simulink model "COMPONENT_MDL_Lag_QUAD_and_PEND_with_Ab"  (R2020b)
(part 3 of 12)

A = reshape([sin(THE_Theta).*(I_xx.*sin(THE_Theta).*(-1.0./2.0)+(I_xz.*cos(THE_Psi).*cos(THE_Theta))./2.0+(I_xy.*cos(THE_Theta).*sin(THE_Psi))./2.0).*-2.0-sin(THE_Theta).*(Iprop_xx.*sin(THE_Theta).*(-1.0./2.0)+(Iprop_xz.*cos(THE_Psi).*cos(THE_Theta))./2.0+(Iprop_xy.*cos(THE_Theta).*sin(THE_Psi))./2.0).*8.0+mprop.*(-cos(THE_Theta).*sin(THE_Psi).*(cg_to_mot_H.*sin(THE_Theta)+cg_to_mot_L.*cos(THE_Psi).*cos(THE_Theta))+cg_to_mot_H.*cos(THE_Theta).*sin(THE_Psi).*sin(THE_Theta)+cg_to_mot_L.*cos(THE_Psi).*cos(THE_Theta).^2.*sin(THE_Psi)).*(cos(THE_Theta).*sin(THE_Psi).*(cg_to_mot_H.*sin(THE_Theta)+cg_to_mot_L.*cos(THE_Psi).*cos(THE_Theta)).*(-1.0./2.0)+(cg_to_mot_H.*cos(THE_Theta).*sin(THE_Psi).*sin(THE_Theta))./2.0+(cg_to_mot_L.*cos(THE_Psi).*cos(THE_Theta).^2.*sin(THE_Psi))./2.0).*2.0+mprop.*(cos(THE_Theta).*sin(THE_Psi).*(cg_to_mot_H.*sin(THE_Theta)-cg_to_mot_L.*cos(THE_Psi).*cos(THE_Theta))-cg_to_mot_H.*cos(THE_Theta).*sin(THE_Psi).*sin(THE_Theta)+cg_to_mot_L.*cos(THE_Psi).*cos(THE_Theta).^2.*sin(THE_Psi)).*((cos(THE_Theta).*sin(THE_Psi).*(cg_to_mot_H.*sin(THE_Theta)-cg_to_mot_L.*cos(THE_Psi).*cos(THE_Theta)))./2.0-(cg_to_mot_H.*cos(THE_Theta).*sin(THE_Psi).*sin(THE_Theta))./2.0+(cg_to_mot_L.*cos(THE_Psi).*cos(THE_Theta).^2.*sin(THE_Psi))./2.0).*2.0+mprop.*((cg_to_mot_H.*sin(THE_Theta)+cg_to_mot_L.*cos(THE_Psi).*cos(THE_Theta)).*(cos(THE_Psi).*sin(THE_Phi)-cos(THE_Phi).*sin(THE_Psi).*sin(THE_Theta))+cg_to_mot_L.*cos(THE_Theta).*sin(THE_Psi).*(sin(THE_Phi).*sin(THE_Psi)+cos(THE_Phi).*cos(THE_Psi).*sin(THE_Theta))-cg_to_mot_H.*cos(THE_Phi).*cos(THE_Theta).^2.*sin(THE_Psi)).*(((cg_to_mot_H.*sin(THE_Theta)+cg_to_mot_L.*cos(THE_Psi).*cos(THE_Theta)).*(cos(THE_Psi).*sin(THE_Phi)-cos(THE_Phi).*sin(THE_Psi).*sin(THE_Theta)))./2.0+(cg_to_mot_L.*cos(THE_Theta).*sin(THE_Psi).*(sin(THE_Phi).*sin(THE_Psi)+cos(THE_Phi).*cos(THE_Psi).*sin(THE_Theta)))./2.0-(cg_to_mot_H.*cos(THE_Phi).*cos(THE_Theta).^2.*sin(THE_Psi))./2.0).*2.0+mprop.*(-(cg_to_mot_H.*sin(THE_Theta)-cg_to_mot_L.*cos(THE_Psi).*cos(THE_Theta)).*(cos(THE_Psi).*sin(THE_Phi)-cos(THE_Phi).*sin(THE_Psi).*sin(THE_Theta))+cg_to_mot_L.*cos(THE_Theta).*sin(THE_Psi).*(sin(THE_Phi).*sin(THE_Psi)+cos(THE_Phi).*cos(THE_Psi).*sin(THE_Theta))+cg_to_mot_H.*cos(THE_Phi).*cos(THE_Theta).^2.*sin(THE_Psi)).*((cg_to_mot_H.*sin(THE_Theta)-cg_to_mot_L.*cos(THE_Psi).*cos(THE_Theta)).*(cos(THE_Psi).*sin(THE_Phi)-cos(THE_Phi).*sin(THE_Psi).*sin(THE_Theta)).*(-1.0./2.0)+(cg_to_mot_L.*cos(THE_Theta).*sin(THE_Psi).*(sin(THE_Phi).*sin(THE_Psi)+cos(THE_Phi).*cos(THE_Psi).*sin(THE_Theta)))./2.0+(cg_to_mot_H.*cos(THE_Phi).*cos(THE_Theta).^2.*sin(THE_Psi))./2.0).*2.0+mprop.*((cg_to_mot_H.*sin(THE_Theta)+cg_to_mot_L.*cos(THE_Psi).*cos(THE_Theta)).*(cos(THE_Phi).*cos(THE_Psi)+sin(THE_Phi).*sin(THE_Psi).*sin(THE_Theta))+cg_to_mot_L.*cos(THE_Theta).*sin(THE_Psi).*(cos(THE_Phi).*sin(THE_Psi)-cos(THE_Psi).*sin(THE_Phi).*sin(THE_Theta))+cg_to_mot_H.*cos(THE_Theta).^2.*sin(THE_Phi).*sin(THE_Psi)).*(((cg_to_mot_H.*sin(THE_Theta)+cg_to_mot_L.*cos(THE_Psi).*cos(THE_Theta)).*(cos(THE_Phi).*cos(THE_Psi)+sin(THE_Phi).*sin(THE_Psi).*sin(THE_Theta)))./2.0+(cg_to_mot_L.*cos(THE_Theta).*sin(THE_Psi).*(cos(THE_Phi).*sin(THE_Psi)-cos(THE_Psi).*sin(THE_Phi).*sin(THE_Theta)))./2.0+(cg_to_mot_H.*cos(THE_Theta).^2.*sin(THE_Phi).*sin(THE_Psi))./2.0).*2.0+mprop.*((cg_to_mot_H.*sin(THE_Theta)-cg_to_mot_L.*cos(THE_Psi).*cos(THE_Theta)).*(cos(THE_Phi).*cos(THE_Psi)+sin(THE_Phi).*sin(THE_Psi).*sin(THE_Theta))-cg_to_mot_L.*cos(THE_Theta).*sin(THE_Psi).*(cos(THE_Phi).*sin(THE_Psi)-cos(THE_Psi).*sin(THE_Phi).*sin(THE_Theta))+cg_to_mot_H.*cos(THE_Theta).^2.*sin(THE_Phi).*sin(THE_Psi)).*(((cg_to_mot_H.*sin(THE_Theta)-cg_to_mot_L.*cos(THE_Psi).*cos(THE_Theta)).*(cos(THE_Phi).*cos(THE_Psi)+sin(THE_Phi).*sin(THE_Psi).*sin(THE_Theta)))./2.0-(cg_to_mot_L.*cos(THE_Theta).*sin(THE_Psi).*(cos(THE_Phi).*sin(THE_Psi)-cos(THE_Psi).*sin(THE_Phi).*sin(THE_Theta)))./2.0+(cg_to_mot_H.*cos(THE_Theta).^2.*sin(THE_Phi).*sin(THE_Psi))./2.0).*2.0+mprop.*(-sin(THE_Theta).*(cg_to_mot_L.*cos(THE_Psi).*cos(THE_Theta)+cg_to_mot_H.*cos(THE_Theta).*sin(THE_Psi))+cg_to_mot_H.*cos(THE_Theta).*sin(THE_Psi).*sin(THE_Theta)+cg_to_mot_L.*cos(THE_Psi).*cos(THE_Theta).*sin(THE_Theta)).*(sin(THE_Theta).*(cg_to_mot_L.*cos(THE_Psi).*cos(THE_Theta)+cg_to_mot_H.*cos(THE_Theta).*sin(THE_Psi)).*(-1.0./2.0)+(cg_to_mot_H.*cos(THE_Theta).*sin(THE_Psi).*sin(THE_Theta))./2.0+(cg_to_mot_L.*cos(THE_Psi).*cos(THE_Theta).*sin(THE_Theta))./2.0).*2.0+mprop.*(sin(THE_Theta).*(cg_to_mot_L.*cos(THE_Psi).*cos(THE_Theta)-cg_to_mot_H.*cos(THE_Theta).*sin(THE_Psi))+cg_to_mot_H.*cos(THE_Theta).*sin(THE_Psi).*sin(THE_Theta)-cg_to_mot_L.*cos(THE_Psi).*cos(THE_Theta).*sin(THE_Theta)).*((sin(THE_Theta).*(cg_to_mot_L.*cos(THE_Psi).*cos(THE_Theta)-cg_to_mot_H.*cos(THE_Theta).*sin(THE_Psi)))./2.0+(cg_to_mot_H.*cos(THE_Theta).*sin(THE_Psi).*sin(THE_Theta))./2.0-(cg_to_mot_L.*cos(THE_Psi).*cos(THE_Theta).*sin(THE_Theta))./2.0).*2.0+mprop.*(-cg_to_mot_H.*sin(THE_Theta).*(cos(THE_Psi).*sin(THE_Phi)-cos(THE_Phi).*sin(THE_Psi).*sin(THE_Theta))+cg_to_mot_L.*sin(THE_Theta).*(sin(THE_Phi).*sin(THE_Psi)+cos(THE_Phi).*cos(THE_Psi).*sin(THE_Theta))+cos(THE_Phi).*cos(THE_Theta).*(cg_to_mot_L.*cos(THE_Psi).*cos(THE_Theta)+cg_to_mot_H.*cos(THE_Theta).*sin(THE_Psi))).*(cg_to_mot_H.*sin(THE_Theta).*(cos(THE_Psi).*sin(THE_Phi)-cos(THE_Phi).*sin(THE_Psi).*sin(THE_Theta)).*(-1.0./2.0)+(cg_to_mot_L.*sin(THE_Theta).*(sin(THE_Phi).*sin(THE_Psi)+cos(THE_Phi).*cos(THE_Psi).*sin(THE_Theta)))./2.0+(cos(THE_Phi).*cos(THE_Theta).*(cg_to_mot_L.*cos(THE_Psi).*cos(THE_Theta)+cg_to_mot_H.*cos(THE_Theta).*sin(THE_Psi)))./2.0).*2.0+mprop.*(cg_to_mot_H.*sin(THE_Theta).*(cos(THE_Psi).*sin(THE_Phi)-cos(THE_Phi).*sin(THE_Psi).*sin(THE_Theta))+cg_to_mot_L.*sin(THE_Theta).*(sin(THE_Phi).*sin(THE_Psi)+cos(THE_Phi).*cos(THE_Psi).*sin(THE_Theta))+cos(THE_Phi).*cos(THE_Theta).*(cg_to_mot_L.*cos(THE_Psi).*cos(THE_Theta)-cg_to_mot_H.*cos(THE_Theta).*sin(THE_Psi))).*((cg_to_mot_H.*sin(THE_Theta).*(cos(THE_Psi).*sin(THE_Phi)-cos(THE_Phi).*sin(THE_Psi).*sin(THE_Theta)))./2.0+(cg_to_mot_L.*sin(THE_Theta).*(sin(THE_Phi).*sin(THE_Psi)+cos(THE_Phi).*cos(THE_Psi).*sin(THE_Theta)))./2.0+(cos(THE_Phi).*cos(THE_Theta).*(cg_to_mot_L.*cos(THE_Psi).*cos(THE_Theta)-cg_to_mot_H.*cos(THE_Theta).*sin(THE_Psi)))./2.0).*2.0+m_pend.*((Tv_Z_pend+(Lz_pend.*cos(THE_Psi_pend).*cos(THE_Theta_pend))./2.0).*(sin(THE_Phi).*sin(THE_Psi)+cos(THE_Phi).*cos(THE_Psi).*sin(THE_Theta))+(Lz_pend.*(cos(THE_Psi).*sin(THE_Phi)-cos(THE_Phi).*sin(THE_Psi).*sin(THE_Theta)).*(cos(THE_Phi_pend).*sin(THE_Psi_pend)-cos(THE_Psi_pend).*sin(THE_Phi_pend).*sin(THE_Theta_pend)))./2.0+(Lz_pend.*cos(THE_Phi).*cos(THE_Theta).*(sin(THE_Phi_pend).*sin(THE_Psi_pend)+cos(THE_Phi_pend).*cos(THE_Psi_pend).*sin(THE_Theta_pend)))./2.0).*(((Tv_Z_pend+(Lz_pend.*cos(THE_Psi_pend).*cos(THE_Theta_pend))./2.0).*(sin(THE_Phi).*sin(THE_Psi)+cos(THE_Phi).*cos(THE_Psi).*sin(THE_Theta)))./2.0+(Lz_pend.*(cos(THE_Psi).*sin(THE_Phi)-cos(THE_Phi).*sin(THE_Psi).*sin(THE_Theta)).*(cos(THE_Phi_pend).*sin(THE_Psi_pend)-cos(THE_Psi_pend).*sin(THE_Phi_pend).*sin(THE_Theta_pend)))./4.0+(Lz_pend.*cos(THE_Phi).*cos(THE_Theta).*(sin(THE_Phi_pend).*sin(THE_Psi_pend)+cos(THE_Phi_pend).*cos(THE_Psi_pend).*sin(THE_Theta_pend)))./4.0).*2.0+mprop.*(cg_to_mot_H.*sin(THE_Theta).*(cos(THE_Phi).*cos(THE_Psi)+sin(THE_Phi).*sin(THE_Psi).*sin(THE_Theta))-cg_to_mot_L.*sin(THE_Theta).*(cos(THE_Phi).*sin(THE_Psi)-cos(THE_Psi).*sin(THE_Phi).*sin(THE_Theta))+cos(THE_Theta).*sin(THE_Phi).*(cg_to_mot_L.*cos(THE_Psi).*cos(THE_Theta)+cg_to_mot_H.*cos(THE_Theta).*sin(THE_Psi))).*((cg_to_mot_H.*sin(THE_Theta).*(cos(THE_Phi).*cos(THE_Psi)+sin(THE_Phi).*sin(THE_Psi).*sin(THE_Theta)))./2.0-(cg_to_mot_L.*sin(THE_Theta).*(cos(THE_Phi).*sin(THE_Psi)-cos(THE_Psi).*sin(THE_Phi).*sin(THE_Theta)))./2.0+(cos(THE_Theta).*sin(THE_Phi).*(cg_to_mot_L.*cos(THE_Psi).*cos(THE_Theta)+cg_to_mot_H.*cos(THE_Theta).*sin(THE_Psi)))./2.0).*2.0+mprop.*(cg_to_mot_H.*sin(THE_Theta).*(cos(THE_Phi).*cos(THE_Psi)+sin(THE_Phi).*sin(THE_Psi).*sin(THE_Theta))+cg_to_mot_L.*sin(THE_Theta).*(cos(THE_Phi).*sin(THE_Psi)-cos(THE_Psi).*sin(THE_Phi).*sin(THE_Theta))-cos(THE_Theta).*sin(THE_Phi).*(cg_to_mot_L.*cos(THE_Psi).*cos(THE_Theta)-cg_to_mot_H.*cos(THE_Theta).*sin(THE_Psi))).*((cg_to_mot_H.*sin(THE_Theta).*(cos(THE_Phi).*cos(THE_Psi)+sin(THE_Phi).*sin(THE_Psi).*sin(THE_Theta)))./2.0+(cg_to_mot_L.*sin(THE_Theta).*(cos(THE_Phi).*sin(THE_Psi)-cos(THE_Psi).*sin(THE_Phi).*sin(THE_Theta)))./2.0-(cos(THE_Theta).*sin(THE_Phi).*(cg_to_mot_L.*cos(THE_Psi).*cos(THE_Theta)-cg_to_mot_H.*cos(THE_Theta).*sin(THE_Psi)))./2.0).*2.0+m_pend.*((Tv_Z_pend+(Lz_pend.*cos(THE_Psi_pend).*cos(THE_Theta_pend))./2.0).*(cos(THE_Phi).*sin(THE_Psi)-cos(THE_Psi).*sin(THE_Phi).*sin(THE_Theta))+(Lz_pend.*(cos(THE_Phi).*cos(THE_Psi)+sin(THE_Phi).*sin(THE_Psi).*sin(THE_Theta)).*(cos(THE_Phi_pend).*sin(THE_Psi_pend)-cos(THE_Psi_pend).*sin(THE_Phi_pend).*sin(THE_Theta_pend)))./2.0-(Lz_pend.*cos(THE_Theta).*sin(THE_Phi).*(sin(THE_Phi_pend).*sin(THE_Psi_pend)+cos(THE_Phi_pend).*cos(THE_Psi_pend).*sin(THE_Theta_pend)))./2.0).*(((Tv_Z_pend+(Lz_pend.*cos(THE_Psi_pend).*cos(THE_Theta_pend))./2.0).*(cos(THE_Phi).*sin(THE_Psi)-cos(THE_Psi).*sin(THE_Phi).*sin(THE_Theta)))./2.0+(Lz_pend.*(cos(THE_Phi).*cos(THE_Psi)+sin(THE_Phi).*sin(THE_Psi).*sin(THE_Theta)).*(cos(THE_Phi_pend).*sin(THE_Psi_pend)-cos(THE_Psi_pend).*sin(THE_Phi_pend).*sin(THE_Theta_pend)))./4.0-(Lz_pend.*cos(THE_Theta).*sin(THE_Phi).*(sin(THE_Phi_pend).*sin(THE_Psi_pend)+cos(THE_Phi_pend).*cos(THE_Psi_pend).*sin(THE_Theta_pend)))./4.0).*2.0+cos(THE_Psi).*cos(THE_Theta).*(I_xz.*sin(THE_Theta).*(-1.0./2.0)+(I_zz.*cos(THE_Psi).*cos(THE_Theta))./2.0+(I_yz.*cos(THE_Theta).*sin(THE_Psi))./2.0).*2.0+cos(THE_Psi).*cos(THE_Theta).*(Iprop_xz.*sin(THE_Theta).*(-1.0./2.0)+(Iprop_zz.*cos(THE_Psi).*cos(THE_Theta))./2.0+(Iprop_yz.*cos(THE_Theta).*sin(THE_Psi))./2.0).*8.0+cos(THE_Theta).*sin(THE_Psi).*(I_xy.*sin(THE_Theta).*(-1.0./2.0)+(I_yz.*cos(THE_Psi).*cos(THE_Theta))./2.0+(I_yy.*cos(THE_Theta).*sin(THE_Psi))./2.0).*2.0+cos(THE_Theta).*sin(THE_Psi).*(Iprop_xy.*sin(THE_Theta).*(-1.0./2.0)+(Iprop_yz.*cos(THE_Psi).*cos(THE_Theta))./2.0+(Iprop_yy.*cos(THE_Theta).*sin(THE_Psi))./2.0).*8.0+m_pend.*(Ly_pend.^2./1.2e+1+Lz_pend.^2./1.2e+1).*(cos(THE_Psi).*cos(THE_Theta).*sin(THE_Theta_pend)+cos(THE_Phi_pend).*cos(THE_Theta_pend).*sin(THE_Theta)-cos(THE_Theta).*cos(THE_Theta_pend).*sin(THE_Psi).*sin(THE_Phi_pend)).*((cos(THE_Psi).*cos(THE_Theta).*sin(THE_Theta_pend))./2.0+(cos(THE_Phi_pend).*cos(THE_Theta_pend).*sin(THE_Theta))./2.0-(cos(THE_Theta).*cos(THE_Theta_pend).*sin(THE_Psi).*sin(THE_Phi_pend))./2.0).*2.0+m_pend.*(Lx_pend.^2./1.2e+1+Ly_pend.^2./1.2e+1).*(sin(THE_Theta).*(sin(THE_Phi_pend).*sin(THE_Psi_pend)+cos(THE_Phi_pend).*cos(THE_Psi_pend).*sin(THE_Theta_pend))+cos(THE_Theta).*sin(THE_Psi).*(cos(THE_Phi_pend).*sin(THE_Psi_pend)-cos(THE_Psi_pend).*sin(THE_Phi_pend).*sin(THE_Theta_pend))-cos(THE_Psi).*cos(THE_Theta).*cos(THE_Psi_pend).*cos(THE_Theta_pend)).*((sin(THE_Theta).*(sin(THE_Phi_pend).*sin(THE_Psi_pend)+cos(THE_Phi_pend).*cos(THE_Psi_pend).*sin(THE_Theta_pend)))./2.0+(cos(THE_Theta).*sin(THE_Psi).*(cos(THE_Phi_pend).*sin(THE_Psi_pend)-cos(THE_Psi_pend).*sin(THE_Phi_pend).*sin(THE_Theta_pend)))./2.0-(cos(THE_Psi).*cos(THE_Theta).*cos(THE_Psi_pend).*cos(THE_Theta_pend))./2.0).*2.0+m_pend.*(Lx_pend.^2./1.2e+1+Lz_pend.^2./1.2e+1).*(sin(THE_Theta).*(cos(THE_Psi_pend).*sin(THE_Phi_pend)-cos(THE_Phi_pend).*sin(THE_Psi_pend).*sin(THE_Theta_pend))+cos(THE_Theta).*sin(THE_Psi).*(cos(THE_Phi_pend).*cos(THE_Psi_pend)+sin(THE_Phi_pend).*sin(THE_Psi_pend).*sin(THE_Theta_pend))+cos(THE_Psi).*cos(THE_Theta).*cos(THE_Theta_pend).*sin(THE_Psi_pend)).*((sin(THE_Theta).*(cos(THE_Psi_pend).*sin(THE_Phi_pend)-cos(THE_Phi_pend).*sin(THE_Psi_pend).*sin(THE_Theta_pend)))./2.0+(cos(THE_Theta).*sin(THE_Psi).*(cos(THE_Phi_pend).*cos(THE_Psi_pend)+sin(THE_Phi_pend).*sin(THE_Psi_pend).*sin(THE_Theta_pend)))./2.0+(cos(THE_Psi).*cos(THE_Theta).*cos(THE_Theta_pend).*sin(THE_Psi_pend))./2.0).*2.0,cos(THE_Psi).*(I_xy.*sin(THE_Theta).*(-1.0./2.0)+(I_yz.*cos(THE_Psi).*cos(THE_Theta))./2.0+(I_yy.*cos(THE_Theta).*sin(THE_Psi))./2.0)+cos(THE_Psi).*(Iprop_xy.*sin(THE_Theta).*(-1.0./2.0)+(Iprop_yz.*cos(THE_Psi).*cos(THE_Theta))./2.0+(Iprop_yy.*cos(THE_Theta).*sin(THE_Psi))./2.0).*4.0-sin(THE_Psi).*(I_xz.*sin(THE_Theta).*(-1.0./2.0)+(I_zz.*cos(THE_Psi).*cos(THE_Theta))./2.0+(I_yz.*cos(THE_Theta).*sin(THE_Psi))./2.0)-sin(THE_Psi).*(Iprop_xz.*sin(THE_Theta).*(-1.0./2.0)+(Iprop_zz.*cos(THE_Psi).*cos(THE_Theta))./2.0+(Iprop_yz.*cos(THE_Theta).*sin(THE_Psi))./2.0).*4.0-sin(THE_Theta).*((I_xy.*cos(THE_Psi))./2.0-(I_xz.*sin(THE_Psi))./2.0)-sin(THE_Theta).*((Iprop_xy.*cos(THE_Psi))./2.0-(Iprop_xz.*sin(THE_Psi))./2.0).*4.0+cos(THE_Theta).*sin(THE_Psi).*((I_yy.*cos(THE_Psi))./2.0-(I_yz.*sin(THE_Psi))./2.0)+cos(THE_Theta).*sin(THE_Psi).*((Iprop_yy.*cos(THE_Psi))./2.0-(Iprop_yz.*sin(THE_Psi))./2.0).*4.0-mprop.*(-cg_to_mot_L.*cos(THE_Psi).*(sin(THE_Phi).*sin(THE_Psi)+cos(THE_Phi).*cos(THE_Psi).*sin(THE_Theta))+cg_to_mot_L.*sin(THE_Psi).*(cos(THE_Psi).*sin(THE_Phi)-cos(THE_Phi).*sin(THE_Psi).*sin(THE_Theta))+cg_to_mot_H.*cos(THE_Phi).*cos(THE_Psi).*cos(THE_Theta)).*(((cg_to_mot_H.*sin(THE_Theta)+cg_to_mot_L.*cos(THE_Psi).*cos(THE_Theta)).*(cos(THE_Psi).*sin(THE_Phi)-cos(THE_Phi).*sin(THE_Psi).*sin(THE_Theta)))./2.0+(cg_to_mot_L.*cos(THE_Theta).*sin(THE_Psi).*(sin(THE_Phi).*sin(THE_Psi)+cos(THE_Phi).*cos(THE_Psi).*sin(THE_Theta)))./2.0-(cg_to_mot_H.*cos(THE_Phi).*cos(THE_Theta).^2.*sin(THE_Psi))./2.0)-mprop.*(cg_to_mot_L.*cos(THE_Psi).*(sin(THE_Phi).*sin(THE_Psi)+cos(THE_Phi).*cos(THE_Psi).*sin(THE_Theta)).*(-1.0./2.0)+(cg_to_mot_L.*sin(THE_Psi).*(cos(THE_Psi).*sin(THE_Phi)-cos(THE_Phi).*sin(THE_Psi).*sin(THE_Theta)))./2.0+(cg_to_mot_H.*cos(THE_Phi).*cos(THE_Psi).*cos(THE_Theta))./2.0).*((cg_to_mot_H.*sin(THE_Theta)+cg_to_mot_L.*cos(THE_Psi).*cos(THE_Theta)).*(cos(THE_Psi).*sin(THE_Phi)-cos(THE_Phi).*sin(THE_Psi).*sin(THE_Theta))+cg_to_mot_L.*cos(THE_Theta).*sin(THE_Psi).*(sin(THE_Phi).*sin(THE_Psi)+cos(THE_Phi).*cos(THE_Psi).*sin(THE_Theta))-cg_to_mot_H.*cos(THE_Phi).*cos(THE_Theta).^2.*sin(THE_Psi))+mprop.*(cg_to_mot_L.*cos(THE_Psi).*(sin(THE_Phi).*sin(THE_Psi)+cos(THE_Phi).*cos(THE_Psi).*sin(THE_Theta))-cg_to_mot_L.*sin(THE_Psi).*(cos(THE_Psi).*sin(THE_Phi)-cos(THE_Phi).*sin(THE_Psi).*sin(THE_Theta))+cg_to_mot_H.*cos(THE_Phi).*cos(THE_Psi).*cos(THE_Theta)).*((cg_to_mot_H.*sin(THE_Theta)-cg_to_mot_L.*cos(THE_Psi).*cos(THE_Theta)).*(cos(THE_Psi).*sin(THE_Phi)-cos(THE_Phi).*sin(THE_Psi).*sin(THE_Theta)).*(-1.0./2.0)+(cg_to_mot_L.*cos(THE_Theta).*sin(THE_Psi).*(sin(THE_Phi).*sin(THE_Psi)+cos(THE_Phi).*cos(THE_Psi).*sin(THE_Theta)))./2.0+(cg_to_mot_H.*cos(THE_Phi).*cos(THE_Theta).^2.*sin(THE_Psi))./2.0)+mprop.*((cg_to_mot_L.*cos(THE_Psi).*(sin(THE_Phi).*sin(THE_Psi)+cos(THE_Phi).*cos(THE_Psi).*sin(THE_Theta)))./2.0-(cg_to_mot_L.*sin(THE_Psi).*(cos(THE_Psi).*sin(THE_Phi)-cos(THE_Phi).*sin(THE_Psi).*sin(THE_Theta)))./2.0+(cg_to_mot_H.*cos(THE_Phi).*cos(THE_Psi).*cos(THE_Theta))./2.0).*(-(cg_to_mot_H.*sin(THE_Theta)-cg_to_mot_L.*cos(THE_Psi).*cos(THE_Theta)).*(cos(THE_Psi).*sin(THE_Phi)-cos(THE_Phi).*sin(THE_Psi).*sin(THE_Theta))+cg_to_mot_L.*cos(THE_Theta).*sin(THE_Psi).*(sin(THE_Phi).*sin(THE_Psi)+cos(THE_Phi).*cos(THE_Psi).*sin(THE_Theta))+cg_to_mot_H.*cos(THE_Phi).*cos(THE_Theta).^2.*sin(THE_Psi))+mprop.*((cg_to_mot_L.*cos(THE_Psi).*(cos(THE_Phi).*sin(THE_Psi)-cos(THE_Psi).*sin(THE_Phi).*sin(THE_Theta)))./2.0-(cg_to_mot_L.*sin(THE_Psi).*(cos(THE_Phi).*cos(THE_Psi)+sin(THE_Phi).*sin(THE_Psi).*sin(THE_Theta)))./2.0+(cg_to_mot_H.*cos(THE_Psi).*cos(THE_Theta).*sin(THE_Phi))./2.0).*((cg_to_mot_H.*sin(THE_Theta)+cg_to_mot_L.*cos(THE_Psi).*cos(THE_Theta)).*(cos(THE_Phi).*cos(THE_Psi)+sin(THE_Phi).*sin(THE_Psi).*sin(THE_Theta))+cg_to_mot_L.*cos(THE_Theta).*sin(THE_Psi).*(cos(THE_Phi).*sin(THE_Psi)-cos(THE_Psi).*sin(THE_Phi).*sin(THE_Theta))+cg_to_mot_H.*cos(THE_Theta).^2.*sin(THE_Phi).*sin(THE_Psi))+mprop.*(cg_to_mot_L.*cos(THE_Psi).*(cos(THE_Phi).*sin(THE_Psi)-cos(THE_Psi).*sin(THE_Phi).*sin(THE_Theta))-cg_to_mot_L.*sin(THE_Psi).*(cos(THE_Phi).*cos(THE_Psi)+sin(THE_Phi).*sin(THE_Psi).*sin(THE_Theta))+cg_to_mot_H.*cos(THE_Psi).*cos(THE_Theta).*sin(THE_Phi)).*(((cg_to_mot_H.*sin(THE_Theta)+cg_to_mot_L.*cos(THE_Psi).*cos(THE_Theta)).*(cos(THE_Phi).*cos(THE_Psi)+sin(THE_Phi).*sin(THE_Psi).*sin(THE_Theta)))./2.0+(cg_to_mot_L.*cos(THE_Theta).*sin(THE_Psi).*(cos(THE_Phi).*sin(THE_Psi)-cos(THE_Psi).*sin(THE_Phi).*sin(THE_Theta)))./2.0+(cg_to_mot_H.*cos(THE_Theta).^2.*sin(THE_Phi).*sin(THE_Psi))./2.0)+mprop.*(-cg_to_mot_L.*cos(THE_Psi).*(cos(THE_Phi).*sin(THE_Psi)-cos(THE_Psi).*sin(THE_Phi).*sin(THE_Theta))+cg_to_mot_L.*sin(THE_Psi).*(cos(THE_Phi).*cos(THE_Psi)+sin(THE_Phi).*sin(THE_Psi).*sin(THE_Theta))+cg_to_mot_H.*cos(THE_Psi).*cos(THE_Theta).*sin(THE_Phi)).*(((cg_to_mot_H.*sin(THE_Theta)-cg_to_mot_L.*cos(THE_Psi).*cos(THE_Theta)).*(cos(THE_Phi).*cos(THE_Psi)+sin(THE_Phi).*sin(THE_Psi).*sin(THE_Theta)))./2.0-(cg_to_mot_L.*cos(THE_Theta).*sin(THE_Psi).*(cos(THE_Phi).*sin(THE_Psi)-cos(THE_Psi).*sin(THE_Phi).*sin(THE_Theta)))./2.0+(cg_to_mot_H.*cos(THE_Theta).^2.*sin(THE_Phi).*sin(THE_Psi))./2.0)+mprop.*(cg_to_mot_L.*cos(THE_Psi).*(cos(THE_Phi).*sin(THE_Psi)-cos(THE_Psi).*sin(THE_Phi).*sin(THE_Theta)).*(-1.0./2.0)+(cg_to_mot_L.*sin(THE_Psi).*(cos(THE_Phi).*cos(THE_Psi)+sin(THE_Phi).*sin(THE_Psi).*sin(THE_Theta)))./2.0+(cg_to_mot_H.*cos(THE_Psi).*cos(THE_Theta).*sin(THE_Phi))./2.0).*((cg_to_mot_H.*sin(THE_Theta)-cg_to_mot_L.*cos(THE_Psi).*cos(THE_Theta)).*(cos(THE_Phi).*cos(THE_Psi)+sin(THE_Phi).*sin(THE_Psi).*sin(THE_Theta))-cg_to_mot_L.*cos(THE_Theta).*sin(THE_Psi).*(cos(THE_Phi).*sin(THE_Psi)-cos(THE_Psi).*sin(THE_Phi).*sin(THE_Theta))+cg_to_mot_H.*cos(THE_Theta).^2.*sin(THE_Phi).*sin(THE_Psi))-m_pend.*((Lz_pend.*cos(THE_Phi).*sin(THE_Theta).*(sin(THE_Phi_pend).*sin(THE_Psi_pend)+cos(THE_Phi_pend).*cos(THE_Psi_pend).*sin(THE_Theta_pend)))./4.0-(cos(THE_Phi).*cos(THE_Psi).*cos(THE_Theta).*(Tv_Z_pend+(Lz_pend.*cos(THE_Psi_pend).*cos(THE_Theta_pend))./2.0))./2.0+(Lz_pend.*cos(THE_Phi).*cos(THE_Theta).*sin(THE_Psi).*(cos(THE_Phi_pend).*sin(THE_Psi_pend)-cos(THE_Psi_pend).*sin(THE_Phi_pend).*sin(THE_Theta_pend)))./4.0).*((Tv_Z_pend+(Lz_pend.*cos(THE_Psi_pend).*cos(THE_Theta_pend))./2.0).*(cos(THE_Phi).*sin(THE_Psi)-cos(THE_Psi).*sin(THE_Phi).*sin(THE_Theta))+(Lz_pend.*(cos(THE_Phi).*cos(THE_Psi)+sin(THE_Phi).*sin(THE_Psi).*sin(THE_Theta)).*(cos(THE_Phi_pend).*sin(THE_Psi_pend)-cos(THE_Psi_pend).*sin(THE_Phi_pend).*sin(THE_Theta_pend)))./2.0-(Lz_pend.*cos(THE_Theta).*sin(THE_Phi).*(sin(THE_Phi_pend).*sin(THE_Psi_pend)+cos(THE_Phi_pend).*cos(THE_Psi_pend).*sin(THE_Theta_pend)))./2.0)-m_pend.*((Lz_pend.*cos(THE_Phi).*sin(THE_Theta).*(sin(THE_Phi_pend).*sin(THE_Psi_pend)+cos(THE_Phi_pend).*cos(THE_Psi_pend).*sin(THE_Theta_pend)))./2.0-cos(THE_Phi).*cos(THE_Psi).*cos(THE_Theta).*(Tv_Z_pend+(Lz_pend.*cos(THE_Psi_pend).*cos(THE_Theta_pend))./2.0)+(Lz_pend.*cos(THE_Phi).*cos(THE_Theta).*sin(THE_Psi).*(cos(THE_Phi_pend).*sin(THE_Psi_pend)-cos(THE_Psi_pend).*sin(THE_Phi_pend).*sin(THE_Theta_pend)))./2.0).*(((Tv_Z_pend+(Lz_pend.*cos(THE_Psi_pend).*cos(THE_Theta_pend))./2.0).*(cos(THE_Phi).*sin(THE_Psi)-cos(THE_Psi).*sin(THE_Phi).*sin(THE_Theta)))./2.0+(Lz_pend.*(cos(THE_Phi).*cos(THE_Psi)+sin(THE_Phi).*sin(THE_Psi).*sin(THE_Theta)).*(cos(THE_Phi_pend).*sin(THE_Psi_pend)-cos(THE_Psi_pend).*sin(THE_Phi_pend).*sin(THE_Theta_pend)))./4.0-(Lz_pend.*cos(THE_Theta).*sin(THE_Phi).*(sin(THE_Phi_pend).*sin(THE_Psi_pend)+cos(THE_Phi_pend).*cos(THE_Psi_pend).*sin(THE_Theta_pend)))./4.0)+mprop.*(cos(THE_Theta).*sin(THE_Psi).*(cg_to_mot_H.*sin(THE_Theta)+cg_to_mot_L.*cos(THE_Psi).*cos(THE_Theta)).*(-1.0./2.0)+(cg_to_mot_H.*cos(THE_Theta).*sin(THE_Psi).*sin(THE_Theta))./2.0+(cg_to_mot_L.*cos(THE_Psi).*cos(THE_Theta).^2.*sin(THE_Psi))./2.0).*(cg_to_mot_H.*cos(THE_Psi).*sin(THE_Theta)+cg_to_mot_L.*cos(THE_Psi).^2.*cos(THE_Theta)+cg_to_mot_L.*cos(THE_Theta).*sin(THE_Psi).^2)+mprop.*(-cos(THE_Theta).*sin(THE_Psi).*(cg_to_mot_H.*sin(THE_Theta)+cg_to_mot_L.*cos(THE_Psi).*cos(THE_Theta))+cg_to_mot_H.*cos(THE_Theta).*sin(THE_Psi).*sin(THE_Theta)+cg_to_mot_L.*cos(THE_Psi).*cos(THE_Theta).^2.*sin(THE_Psi)).*((cg_to_mot_H.*cos(THE_Psi).*sin(THE_Theta))./2.0+(cg_to_mot_L.*cos(THE_Psi).^2.*cos(THE_Theta))./2.0+(cg_to_mot_L.*cos(THE_Theta).*sin(THE_Psi).^2)./2.0)+mprop.*(cos(THE_Theta).*sin(THE_Psi).*(cg_to_mot_H.*sin(THE_Theta)-cg_to_mot_L.*cos(THE_Psi).*cos(THE_Theta))-cg_to_mot_H.*cos(THE_Theta).*sin(THE_Psi).*sin(THE_Theta)+cg_to_mot_L.*cos(THE_Psi).*cos(THE_Theta).^2.*sin(THE_Psi)).*(cg_to_mot_H.*cos(THE_Psi).*sin(THE_Theta).*(-1.0./2.0)+(cg_to_mot_L.*cos(THE_Psi).^2.*cos(THE_Theta))./2.0+(cg_to_mot_L.*cos(THE_Theta).*sin(THE_Psi).^2)./2.0)+mprop.*((cos(THE_Theta).*sin(THE_Psi).*(cg_to_mot_H.*sin(THE_Theta)-cg_to_mot_L.*cos(THE_Psi).*cos(THE_Theta)))./2.0-(cg_to_mot_H.*cos(THE_Theta).*sin(THE_Psi).*sin(THE_Theta))./2.0+(cg_to_mot_L.*cos(THE_Psi).*cos(THE_Theta).^2.*sin(THE_Psi))./2.0).*(-cg_to_mot_H.*cos(THE_Psi).*sin(THE_Theta)+cg_to_mot_L.*cos(THE_Psi).^2.*cos(THE_Theta)+cg_to_mot_L.*cos(THE_Theta).*sin(THE_Psi).^2)-m_pend.*((Lz_pend.*sin(THE_Phi).*sin(THE_Theta).*(sin(THE_Phi_pend).*sin(THE_Psi_pend)+cos(THE_Phi_pend).*cos(THE_Psi_pend).*sin(THE_Theta_pend)))./4.0-(cos(THE_Psi).*cos(THE_Theta).*sin(THE_Phi).*(Tv_Z_pend+(Lz_pend.*cos(THE_Psi_pend).*cos(THE_Theta_pend))./2.0))./2.0+(Lz_pend.*cos(THE_Theta).*sin(THE_Phi).*sin(THE_Psi).*(cos(THE_Phi_pend).*sin(THE_Psi_pend)-cos(THE_Psi_pend).*sin(THE_Phi_pend).*sin(THE_Theta_pend)))./4.0).*((Tv_Z_pend+(Lz_pend.*cos(THE_Psi_pend).*cos(THE_Theta_pend))./2.0).*(sin(THE_Phi).*sin(THE_Psi)+cos(THE_Phi).*cos(THE_Psi).*sin(THE_Theta))+(Lz_pend.*(cos(THE_Psi).*sin(THE_Phi)-cos(THE_Phi).*sin(THE_Psi).*sin(THE_Theta)).*(cos(THE_Phi_pend).*sin(THE_Psi_pend)-cos(THE_Psi_pend).*sin(THE_Phi_pend).*sin(THE_Theta_pend)))./2.0+(Lz_pend.*cos(THE_Phi).*cos(THE_Theta).*(sin(THE_Phi_pend).*sin(THE_Psi_pend)+cos(THE_Phi_pend).*cos(THE_Psi_pend).*sin(THE_Theta_pend)))./2.0)-m_pend.*((Lz_pend.*sin(THE_Phi).*sin(THE_Theta).*(sin(THE_Phi_pend).*sin(THE_Psi_pend)+cos(THE_Phi_pend).*cos(THE_Psi_pend).*sin(THE_Theta_pend)))./2.0-cos(THE_Psi).*cos(THE_Theta).*sin(THE_Phi).*(Tv_Z_pend+(Lz_pend.*cos(THE_Psi_pend).*cos(THE_Theta_pend))./2.0)+(Lz_pend.*cos(THE_Theta).*sin(THE_Phi).*sin(THE_Psi).*(cos(THE_Phi_pend).*sin(THE_Psi_pend)-cos(THE_Psi_pend).*sin(THE_Phi_pend).*sin(THE_Theta_pend)))./2.0).*(((Tv_Z_pend+(Lz_pend.*cos(THE_Psi_pend).*cos(THE_Theta_pend))./2.0).*(sin(THE_Phi).*sin(THE_Psi)+cos(THE_Phi).*cos(THE_Psi).*sin(THE_Theta)))./2.0+(Lz_pend.*(cos(THE_Psi).*sin(THE_Phi)-cos(THE_Phi).*sin(THE_Psi).*sin(THE_Theta)).*(cos(THE_Phi_pend).*sin(THE_Psi_pend)-cos(THE_Psi_pend).*sin(THE_Phi_pend).*sin(THE_Theta_pend)))./4.0+(Lz_pend.*cos(THE_Phi).*cos(THE_Theta).*(sin(THE_Phi_pend).*sin(THE_Psi_pend)+cos(THE_Phi_pend).*cos(THE_Psi_pend).*sin(THE_Theta_pend)))./4.0)+cos(THE_Psi).*cos(THE_Theta).*((I_yz.*cos(THE_Psi))./2.0-(I_zz.*sin(THE_Psi))./2.0)+cos(THE_Psi).*cos(THE_Theta).*((Iprop_yz.*cos(THE_Psi))./2.0-(Iprop_zz.*sin(THE_Psi))./2.0).*4.0-m_pend.*(Ly_pend.^2./1.2e+1+Lz_pend.^2./1.2e+1).*((sin(THE_Psi).*sin(THE_Theta_pend))./2.0+(cos(THE_Psi).*cos(THE_Theta_pend).*sin(THE_Phi_pend))./2.0).*(cos(THE_Psi).*cos(THE_Theta).*sin(THE_Theta_pend)+cos(THE_Phi_pend).*cos(THE_Theta_pend).*sin(THE_Theta)-cos(THE_Theta).*cos(THE_Theta_pend).*sin(THE_Psi).*sin(THE_Phi_pend))-m_pend.*(Ly_pend.^2./1.2e+1+Lz_pend.^2./1.2e+1).*(sin(THE_Psi).*sin(THE_Theta_pend)+cos(THE_Psi).*cos(THE_Theta_pend).*sin(THE_Phi_pend)).*((cos(THE_Psi).*cos(THE_Theta).*sin(THE_Theta_pend))./2.0+(cos(THE_Phi_pend).*cos(THE_Theta_pend).*sin(THE_Theta))./2.0-(cos(THE_Theta).*cos(THE_Theta_pend).*sin(THE_Psi).*sin(THE_Phi_pend))./2.0)-(mprop.*sin(THE_Theta).*(cg_to_mot_H.*cos(THE_Psi)+cg_to_mot_L.*sin(THE_Psi)).*(sin(THE_Theta).*(cg_to_mot_L.*cos(THE_Psi).*cos(THE_Theta)-cg_to_mot_H.*cos(THE_Theta).*sin(THE_Psi))+cg_to_mot_H.*cos(THE_Theta).*sin(THE_Psi).*sin(THE_Theta)-cg_to_mot_L.*cos(THE_Psi).*cos(THE_Theta).*sin(THE_Theta)))./2.0-(mprop.*sin(THE_Theta).*(cg_to_mot_H.*cos(THE_Psi)-cg_to_mot_L.*sin(THE_Psi)).*(-sin(THE_Theta).*(cg_to_mot_L.*cos(THE_Psi).*cos(THE_Theta)+cg_to_mot_H.*cos(THE_Theta).*sin(THE_Psi))+cg_to_mot_H.*cos(THE_Theta).*sin(THE_Psi).*sin(THE_Theta)+cg_to_mot_L.*cos(THE_Psi).*cos(THE_Theta).*sin(THE_Theta)))./2.0-mprop.*sin(THE_Theta).*(cg_to_mot_H.*cos(THE_Psi)+cg_to_mot_L.*sin(THE_Psi)).*((sin(THE_Theta).*(cg_to_mot_L.*cos(THE_Psi).*cos(THE_Theta)-cg_to_mot_H.*cos(THE_Theta).*sin(THE_Psi)))./2.0+(cg_to_mot_H.*cos(THE_Theta).*sin(THE_Psi).*sin(THE_Theta))./2.0-(cg_to_mot_L.*cos(THE_Psi).*cos(THE_Theta).*sin(THE_Theta))./2.0)-mprop.*sin(THE_Theta).*(cg_to_mot_H.*cos(THE_Psi)-cg_to_mot_L.*sin(THE_Psi)).*(sin(THE_Theta).*(cg_to_mot_L.*cos(THE_Psi).*cos(THE_Theta)+cg_to_mot_H.*cos(THE_Theta).*sin(THE_Psi)).*(-1.0./2.0)+(cg_to_mot_H.*cos(THE_Theta).*sin(THE_Psi).*sin(THE_Theta))./2.0+(cg_to_mot_L.*cos(THE_Psi).*cos(THE_Theta).*sin(THE_Theta))./2.0)+m_pend.*(Lx_pend.^2./1.2e+1+Ly_pend.^2./1.2e+1).*((cos(THE_Psi).*(cos(THE_Phi_pend).*sin(THE_Psi_pend)-cos(THE_Psi_pend).*sin(THE_Phi_pend).*sin(THE_Theta_pend)))./2.0+(cos(THE_Psi_pend).*cos(THE_Theta_pend).*sin(THE_Psi))./2.0).*(sin(THE_Theta).*(sin(THE_Phi_pend).*sin(THE_Psi_pend)+cos(THE_Phi_pend).*cos(THE_Psi_pend).*sin(THE_Theta_pend))+cos(THE_Theta).*sin(THE_Psi).*(cos(THE_Phi_pend).*sin(THE_Psi_pend)-cos(THE_Psi_pend).*sin(THE_Phi_pend).*sin(THE_Theta_pend))-cos(THE_Psi).*cos(THE_Theta).*cos(THE_Psi_pend).*cos(THE_Theta_pend))+m_pend.*(Lx_pend.^2./1.2e+1+Ly_pend.^2./1.2e+1).*(cos(THE_Psi).*(cos(THE_Phi_pend).*sin(THE_Psi_pend)-cos(THE_Psi_pend).*sin(THE_Phi_pend).*sin(THE_Theta_pend))+cos(THE_Psi_pend).*cos(THE_Theta_pend).*sin(THE_Psi)).*((sin(THE_Theta).*(sin(THE_Phi_pend).*sin(THE_Psi_pend)+cos(THE_Phi_pend).*cos(THE_Psi_pend).*sin(THE_Theta_pend)))./2.0+(cos(THE_Theta).*sin(THE_Psi).*(cos(THE_Phi_pend).*sin(THE_Psi_pend)-cos(THE_Psi_pend).*sin(THE_Phi_pend).*sin(THE_Theta_pend)))./2.0-(cos(THE_Psi).*cos(THE_Theta).*cos(THE_Psi_pend).*cos(THE_Theta_pend))./2.0)+m_pend.*((cos(THE_Psi).*(cos(THE_Phi_pend).*cos(THE_Psi_pend)+sin(THE_Phi_pend).*sin(THE_Psi_pend).*sin(THE_Theta_pend)))./2.0-(cos(THE_Theta_pend).*sin(THE_Psi).*sin(THE_Psi_pend))./2.0).*(Lx_pend.^2./1.2e+1+Lz_pend.^2./1.2e+1).*(sin(THE_Theta).*(cos(THE_Psi_pend).*sin(THE_Phi_pend)-cos(THE_Phi_pend).*sin(THE_Psi_pend).*sin(THE_Theta_pend))+cos(THE_Theta).*sin(THE_Psi).*(cos(THE_Phi_pend).*cos(THE_Psi_pend)+sin(THE_Phi_pend).*sin(THE_Psi_pend).*sin(THE_Theta_pend))+cos(THE_Psi).*cos(THE_Theta).*cos(THE_Theta_pend).*sin(THE_Psi_pend))+m_pend.*(cos(THE_Psi).*(cos(THE_Phi_pend).*cos(THE_Psi_pend)+sin(THE_Phi_pend).*sin(THE_Psi_pend).*sin(THE_Theta_pend))-cos(THE_Theta_pend).*sin(THE_Psi).*sin(THE_Psi_pend)).*(Lx_pend.^2./1.2e+1+Lz_pend.^2./1.2e+1).*((sin(THE_Theta).*(cos(THE_Psi_pend).*sin(THE_Phi_pend)-cos(THE_Phi_pend).*sin(THE_Psi_pend).*sin(THE_Theta_pend)))./2.0+(cos(THE_Theta).*sin(THE_Psi).*(cos(THE_Phi_pend).*cos(THE_Psi_pend)+sin(THE_Phi_pend).*sin(THE_Psi_pend).*sin(THE_Theta_pend)))./2.0+(cos(THE_Psi).*cos(THE_Theta).*cos(THE_Theta_pend).*sin(THE_Psi_pend))./2.0)-(mprop.*cos(THE_Phi).*cos(THE_Theta).*(cg_to_mot_H.*cos(THE_Psi)+cg_to_mot_L.*sin(THE_Psi)).*(cg_to_mot_H.*sin(THE_Theta).*(cos(THE_Psi).*sin(THE_Phi)-cos(THE_Phi).*sin(THE_Psi).*sin(THE_Theta))+cg_to_mot_L.*sin(THE_Theta).*(sin(THE_Phi).*sin(THE_Psi)+cos(THE_Phi).*cos(THE_Psi).*sin(THE_Theta))+cos(THE_Phi).*cos(THE_Theta).*(cg_to_mot_L.*cos(THE_Psi).*cos(THE_Theta)-cg_to_mot_H.*cos(THE_Theta).*sin(THE_Psi))))./2.0+(mprop.*cos(THE_Phi).*cos(THE_Theta).*(cg_to_mot_H.*cos(THE_Psi)-cg_to_mot_L.*sin(THE_Psi)).*(-cg_to_mot_H.*sin(THE_Theta).*(cos(THE_Psi).*sin(THE_Phi)-cos(THE_Phi).*sin(THE_Psi).*sin(THE_Theta))+cg_to_mot_L.*sin(THE_Theta).*(sin(THE_Phi).*sin(THE_Psi)+cos(THE_Phi).*cos(THE_Psi).*sin(THE_Theta))+cos(THE_Phi).*cos(THE_Theta).*(cg_to_mot_L.*cos(THE_Psi).*cos(THE_Theta)+cg_to_mot_H.*cos(THE_Theta).*sin(THE_Psi))))./2.0-mprop.*cos(THE_Phi).*cos(THE_Theta).*(cg_to_mot_H.*cos(THE_Psi)+cg_to_mot_L.*sin(THE_Psi)).*((cg_to_mot_H.*sin(THE_Theta).*(cos(THE_Psi).*sin(THE_Phi)-cos(THE_Phi).*sin(THE_Psi).*sin(THE_Theta)))./2.0+(cg_to_mot_L.*sin(THE_Theta).*(sin(THE_Phi).*sin(THE_Psi)+cos(THE_Phi).*cos(THE_Psi).*sin(THE_Theta)))./2.0+(cos(THE_Phi).*cos(THE_Theta).*(cg_to_mot_L.*cos(THE_Psi).*cos(THE_Theta)-cg_to_mot_H.*cos(THE_Theta).*sin(THE_Psi)))./2.0)+mprop.*cos(THE_Phi).*cos(THE_Theta).*(cg_to_mot_H.*cos(THE_Psi)-cg_to_mot_L.*sin(THE_Psi)).*(cg_to_mot_H.*sin(THE_Theta).*(cos(THE_Psi).*sin(THE_Phi)-cos(THE_Phi).*sin(THE_Psi).*sin(THE_Theta)).*(-1.0./2.0)+(cg_to_mot_L.*sin(THE_Theta).*(sin(THE_Phi).*sin(THE_Psi)+cos(THE_Phi).*cos(THE_Psi).*sin(THE_Theta)))./2.0+(cos(THE_Phi).*cos(THE_Theta).*(cg_to_mot_L.*cos(THE_Psi).*cos(THE_Theta)+cg_to_mot_H.*cos(THE_Theta).*sin(THE_Psi)))./2.0)+(mprop.*cos(THE_Theta).*sin(THE_Phi).*(cg_to_mot_H.*cos(THE_Psi)+cg_to_mot_L.*sin(THE_Psi)).*(cg_to_mot_H.*sin(THE_Theta).*(cos(THE_Phi).*cos(THE_Psi)+sin(THE_Phi).*sin(THE_Psi).*sin(THE_Theta))+cg_to_mot_L.*sin(THE_Theta).*(cos(THE_Phi).*sin(THE_Psi)-cos(THE_Psi).*sin(THE_Phi).*sin(THE_Theta))-cos(THE_Theta).*sin(THE_Phi).*(cg_to_mot_L.*cos(THE_Psi).*cos(THE_Theta)-cg_to_mot_H.*cos(THE_Theta).*sin(THE_Psi))))./2.0+(mprop.*cos(THE_Theta).*sin(THE_Phi).*(cg_to_mot_H.*cos(THE_Psi)-cg_to_mot_L.*sin(THE_Psi)).*(cg_to_mot_H.*sin(THE_Theta).*(cos(THE_Phi).*cos(THE_Psi)+sin(THE_Phi).*sin(THE_Psi).*sin(THE_Theta))-cg_to_mot_L.*sin(THE_Theta).*(cos(THE_Phi).*sin(THE_Psi)-cos(THE_Psi).*sin(THE_Phi).*sin(THE_Theta))+cos(THE_Theta).*sin(THE_Phi).*(cg_to_mot_L.*cos(THE_Psi).*cos(THE_Theta)+cg_to_mot_H.*cos(THE_Theta).*sin(THE_Psi))))./2.0+mprop.*cos(THE_Theta).*sin(THE_Phi).*(cg_to_mot_H.*cos(THE_Psi)+cg_to_mot_L.*sin(THE_Psi)).*((cg_to_mot_H.*sin(THE_Theta).*(cos(THE_Phi).*cos(THE_Psi)+sin(THE_Phi).*sin(THE_Psi).*sin(THE_Theta)))./2.0+(cg_to_mot_L.*sin(THE_Theta).*(cos(THE_Phi).*sin(THE_Psi)-cos(THE_Psi).*sin(THE_Phi).*sin(THE_Theta)))./2.0-(cos(THE_Theta).*sin(THE_Phi).*(cg_to_mot_L.*cos(THE_Psi).*cos(THE_Theta)-cg_to_mot_H.*cos(THE_Theta).*sin(THE_Psi)))./2.0)+mprop.*cos(THE_Theta).*sin(THE_Phi).*(cg_to_mot_H.*cos(THE_Psi)-cg_to_mot_L.*sin(THE_Psi)).*((cg_to_mot_H.*sin(THE_Theta).*(cos(THE_Phi).*cos(THE_Psi)+sin(THE_Phi).*sin(THE_Psi).*sin(THE_Theta)))./2.0-(cg_to_mot_L.*sin(THE_Theta).*(cos(THE_Phi).*sin(THE_Psi)-cos(THE_Psi).*sin(THE_Phi).*sin(THE_Theta)))./2.0+(cos(THE_Theta).*sin(THE_Phi).*(cg_to_mot_L.*cos(THE_Psi).*cos(THE_Theta)+cg_to_mot_H.*cos(THE_Theta).*sin(THE_Psi)))./2.0),-I_xx.*sin(THE_Theta)-Iprop_xx.*sin(THE_Theta).*4.0+I_xz.*cos(THE_Psi).*cos(THE_Theta)+Iprop_xz.*cos(THE_Psi).*cos(THE_Theta).*4.0+I_xy.*cos(THE_Theta).*sin(THE_Psi)+Iprop_xy.*cos(THE_Theta).*sin(THE_Psi).*4.0+mprop.*((cg_to_mot_H.*(cos(THE_Psi).*sin(THE_Phi)-cos(THE_Phi).*sin(THE_Psi).*sin(THE_Theta)))./2.0-(cg_to_mot_L.*(sin(THE_Phi).*sin(THE_Psi)+cos(THE_Phi).*cos(THE_Psi).*sin(THE_Theta)))./2.0).*(-cg_to_mot_H.*sin(THE_Theta).*(cos(THE_Psi).*sin(THE_Phi)-cos(THE_Phi).*sin(THE_Psi).*sin(THE_Theta))+cg_to_mot_L.*sin(THE_Theta).*(sin(THE_Phi).*sin(THE_Psi)+cos(THE_Phi).*cos(THE_Psi).*sin(THE_Theta))+cos(THE_Phi).*cos(THE_Theta).*(cg_to_mot_L.*cos(THE_Psi).*cos(THE_Theta)+cg_to_mot_H.*cos(THE_Theta).*sin(THE_Psi)))-mprop.*((cg_to_mot_H.*(cos(THE_Psi).*sin(THE_Phi)-cos(THE_Phi).*sin(THE_Psi).*sin(THE_Theta)))./2.0+(cg_to_mot_L.*(sin(THE_Phi).*sin(THE_Psi)+cos(THE_Phi).*cos(THE_Psi).*sin(THE_Theta)))./2.0).*(cg_to_mot_H.*sin(THE_Theta).*(cos(THE_Psi).*sin(THE_Phi)-cos(THE_Phi).*sin(THE_Psi).*sin(THE_Theta))+cg_to_mot_L.*sin(THE_Theta).*(sin(THE_Phi).*sin(THE_Psi)+cos(THE_Phi).*cos(THE_Psi).*sin(THE_Theta))+cos(THE_Phi).*cos(THE_Theta).*(cg_to_mot_L.*cos(THE_Psi).*cos(THE_Theta)-cg_to_mot_H.*cos(THE_Theta).*sin(THE_Psi)))-mprop.*(cg_to_mot_H.*(cos(THE_Psi).*sin(THE_Phi)-cos(THE_Phi).*sin(THE_Psi).*sin(THE_Theta))+cg_to_mot_L.*(sin(THE_Phi).*sin(THE_Psi)+cos(THE_Phi).*cos(THE_Psi).*sin(THE_Theta))).*((cg_to_mot_H.*sin(THE_Theta).*(cos(THE_Psi).*sin(THE_Phi)-cos(THE_Phi).*sin(THE_Psi).*sin(THE_Theta)))./2.0+(cg_to_mot_L.*sin(THE_Theta).*(sin(THE_Phi).*sin(THE_Psi)+cos(THE_Phi).*cos(THE_Psi).*sin(THE_Theta)))./2.0+(cos(THE_Phi).*cos(THE_Theta).*(cg_to_mot_L.*cos(THE_Psi).*cos(THE_Theta)-cg_to_mot_H.*cos(THE_Theta).*sin(THE_Psi)))./2.0)+mprop.*(cg_to_mot_H.*(cos(THE_Psi).*sin(THE_Phi)-cos(THE_Phi).*sin(THE_Psi).*sin(THE_Theta))-cg_to_mot_L.*(sin(THE_Phi).*sin(THE_Psi)+cos(THE_Phi).*cos(THE_Psi).*sin(THE_Theta))).*(cg_to_mot_H.*sin(THE_Theta).*(cos(THE_Psi).*sin(THE_Phi)-cos(THE_Phi).*sin(THE_Psi).*sin(THE_Theta)).*(-1.0./2.0)+(cg_to_mot_L.*sin(THE_Theta).*(sin(THE_Phi).*sin(THE_Psi)+cos(THE_Phi).*cos(THE_Psi).*sin(THE_Theta)))./2.0+(cos(THE_Phi).*cos(THE_Theta).*(cg_to_mot_L.*cos(THE_Psi).*cos(THE_Theta)+cg_to_mot_H.*cos(THE_Theta).*sin(THE_Psi)))./2.0)-mprop.*((cg_to_mot_H.*(cos(THE_Phi).*cos(THE_Psi)+sin(THE_Phi).*sin(THE_Psi).*sin(THE_Theta)))./2.0-(cg_to_mot_L.*(cos(THE_Phi).*sin(THE_Psi)-cos(THE_Psi).*sin(THE_Phi).*sin(THE_Theta)))./2.0).*(cg_to_mot_H.*sin(THE_Theta).*(cos(THE_Phi).*cos(THE_Psi)+sin(THE_Phi).*sin(THE_Psi).*sin(THE_Theta))-cg_to_mot_L.*sin(THE_Theta).*(cos(THE_Phi).*sin(THE_Psi)-cos(THE_Psi).*sin(THE_Phi).*sin(THE_Theta))+cos(THE_Theta).*sin(THE_Phi).*(cg_to_mot_L.*cos(THE_Psi).*cos(THE_Theta)+cg_to_mot_H.*cos(THE_Theta).*sin(THE_Psi)))-mprop.*((cg_to_mot_H.*(cos(THE_Phi).*cos(THE_Psi)+sin(THE_Phi).*sin(THE_Psi).*sin(THE_Theta)))./2.0+(cg_to_mot_L.*(cos(THE_Phi).*sin(THE_Psi)-cos(THE_Psi).*sin(THE_Phi).*sin(THE_Theta)))./2.0).*(cg_to_mot_H.*sin(THE_Theta).*(cos(THE_Phi).*cos(THE_Psi)+sin(THE_Phi).*sin(THE_Psi).*sin(THE_Theta))+cg_to_mot_L.*sin(THE_Theta).*(cos(THE_Phi).*sin(THE_Psi)-cos(THE_Psi).*sin(THE_Phi).*sin(THE_Theta))-cos(THE_Theta).*sin(THE_Phi).*(cg_to_mot_L.*cos(THE_Psi).*cos(THE_Theta)-cg_to_mot_H.*cos(THE_Theta).*sin(THE_Psi)))-mprop.*(cg_to_mot_H.*(cos(THE_Phi).*cos(THE_Psi)+sin(THE_Phi).*sin(THE_Psi).*sin(THE_Theta))+cg_to_mot_L.*(cos(THE_Phi).*sin(THE_Psi)-cos(THE_Psi).*sin(THE_Phi).*sin(THE_Theta))).*((cg_to_mot_H.*sin(THE_Theta).*(cos(THE_Phi).*cos(THE_Psi)+sin(THE_Phi).*sin(THE_Psi).*sin(THE_Theta)))./2.0+(cg_to_mot_L.*sin(THE_Theta).*(cos(THE_Phi).*sin(THE_Psi)-cos(THE_Psi).*sin(THE_Phi).*sin(THE_Theta)))./2.0-(cos(THE_Theta).*sin(THE_Phi).*(cg_to_mot_L.*cos(THE_Psi).*cos(THE_Theta)-cg_to_mot_H.*cos(THE_Theta).*sin(THE_Psi)))./2.0)-mprop.*(cg_to_mot_H.*(cos(THE_Phi).*cos(THE_Psi)+sin(THE_Phi).*sin(THE_Psi).*sin(THE_Theta))-cg_to_mot_L.*(cos(THE_Phi).*sin(THE_Psi)-cos(THE_Psi).*sin(THE_Phi).*sin(THE_Theta))).*((cg_to_mot_H.*sin(THE_Theta).*(cos(THE_Phi).*cos(THE_Psi)+sin(THE_Phi).*sin(THE_Psi).*sin(THE_Theta)))./2.0-(cg_to_mot_L.*sin(THE_Theta).*(cos(THE_Phi).*sin(THE_Psi)-cos(THE_Psi).*sin(THE_Phi).*sin(THE_Theta)))./2.0+(cos(THE_Theta).*sin(THE_Phi).*(cg_to_mot_L.*cos(THE_Psi).*cos(THE_Theta)+cg_to_mot_H.*cos(THE_Theta).*sin(THE_Psi)))./2.0)-m_pend.*(((Tv_Z_pend+(Lz_pend.*cos(THE_Psi_pend).*cos(THE_Theta_pend))./2.0).*(cos(THE_Phi).*cos(THE_Psi)+sin(THE_Phi).*sin(THE_Psi).*sin(THE_Theta)))./2.0-(Lz_pend.*(cos(THE_Phi).*sin(THE_Psi)-cos(THE_Psi).*sin(THE_Phi).*sin(THE_Theta)).*(cos(THE_Phi_pend).*sin(THE_Psi_pend)-cos(THE_Psi_pend).*sin(THE_Phi_pend).*sin(THE_Theta_pend)))./4.0).*((Tv_Z_pend+(Lz_pend.*cos(THE_Psi_pend).*cos(THE_Theta_pend))./2.0).*(sin(THE_Phi).*sin(THE_Psi)+cos(THE_Phi).*cos(THE_Psi).*sin(THE_Theta))+(Lz_pend.*(cos(THE_Psi).*sin(THE_Phi)-cos(THE_Phi).*sin(THE_Psi).*sin(THE_Theta)).*(cos(THE_Phi_pend).*sin(THE_Psi_pend)-cos(THE_Psi_pend).*sin(THE_Phi_pend).*sin(THE_Theta_pend)))./2.0+(Lz_pend.*cos(THE_Phi).*cos(THE_Theta).*(sin(THE_Phi_pend).*sin(THE_Psi_pend)+cos(THE_Phi_pend).*cos(THE_Psi_pend).*sin(THE_Theta_pend)))./2.0)-m_pend.*((Tv_Z_pend+(Lz_pend.*cos(THE_Psi_pend).*cos(THE_Theta_pend))./2.0).*(cos(THE_Phi).*cos(THE_Psi)+sin(THE_Phi).*sin(THE_Psi).*sin(THE_Theta))-(Lz_pend.*(cos(THE_Phi).*sin(THE_Psi)-cos(THE_Psi).*sin(THE_Phi).*sin(THE_Theta)).*(cos(THE_Phi_pend).*sin(THE_Psi_pend)-cos(THE_Psi_pend).*sin(THE_Phi_pend).*sin(THE_Theta_pend)))./2.0).*(((Tv_Z_pend+(Lz_pend.*cos(THE_Psi_pend).*cos(THE_Theta_pend))./2.0).*(sin(THE_Phi).*sin(THE_Psi)+cos(THE_Phi).*cos(THE_Psi).*sin(THE_Theta)))./2.0+(Lz_pend.*(cos(THE_Psi).*sin(THE_Phi)-cos(THE_Phi).*sin(THE_Psi).*sin(THE_Theta)).*(cos(THE_Phi_pend).*sin(THE_Psi_pend)-cos(THE_Psi_pend).*sin(THE_Phi_pend).*sin(THE_Theta_pend)))./4.0+(Lz_pend.*cos(THE_Phi).*cos(THE_Theta).*(sin(THE_Phi_pend).*sin(THE_Psi_pend)+cos(THE_Phi_pend).*cos(THE_Psi_pend).*sin(THE_Theta_pend)))./4.0)+m_pend.*(((Tv_Z_pend+(Lz_pend.*cos(THE_Psi_pend).*cos(THE_Theta_pend))./2.0).*(cos(THE_Psi).*sin(THE_Phi)-cos(THE_Phi).*sin(THE_Psi).*sin(THE_Theta)))./2.0-(Lz_pend.*(sin(THE_Phi).*sin(THE_Psi)+cos(THE_Phi).*cos(THE_Psi).*sin(THE_Theta)).*(cos(THE_Phi_pend).*sin(THE_Psi_pend)-cos(THE_Psi_pend).*sin(THE_Phi_pend).*sin(THE_Theta_pend)))./4.0).*((Tv_Z_pend+(Lz_pend.*cos(THE_Psi_pend).*cos(THE_Theta_pend))./2.0).*(cos(THE_Phi).*sin(THE_Psi)-cos(THE_Psi).*sin(THE_Phi).*sin(THE_Theta))+(Lz_pend.*(cos(THE_Phi).*cos(THE_Psi)+sin(THE_Phi).*sin(THE_Psi).*sin(THE_Theta)).*(cos(THE_Phi_pend).*sin(THE_Psi_pend)-cos(THE_Psi_pend).*sin(THE_Phi_pend).*sin(THE_Theta_pend)))./2.0-(Lz_pend.*cos(THE_Theta).*sin(THE_Phi).*(sin(THE_Phi_pend).*sin(THE_Psi_pend)+cos(THE_Phi_pend).*cos(THE_Psi_pend).*sin(THE_Theta_pend)))./2.0)+m_pend.*((Tv_Z_pend+(Lz_pend.*cos(THE_Psi_pend).*cos(THE_Theta_pend))./2.0).*(cos(THE_Psi).*sin(THE_Phi)-cos(THE_Phi).*sin(THE_Psi).*sin(THE_Theta))-(Lz_pend.*(sin(THE_Phi).*sin(THE_Psi)+cos(THE_Phi).*cos(THE_Psi).*sin(THE_Theta)).*(cos(THE_Phi_pend).*sin(THE_Psi_pend)-cos(THE_Psi_pend).*sin(THE_Phi_pend).*sin(THE_Theta_pend)))./2.0).*(((Tv_Z_pend+(Lz_pend.*cos(THE_Psi_pend).*cos(THE_Theta_pend))./2.0).*(cos(THE_Phi).*sin(THE_Psi)-cos(THE_Psi).*sin(THE_Phi).*sin(THE_Theta)))./2.0+(Lz_pend.*(cos(THE_Phi).*cos(THE_Psi)+sin(THE_Phi).*sin(THE_Psi).*sin(THE_Theta)).*(cos(THE_Phi_pend).*sin(THE_Psi_pend)-cos(THE_Psi_pend).*sin(THE_Phi_pend).*sin(THE_Theta_pend)))./4.0-(Lz_pend.*cos(THE_Theta).*sin(THE_Phi).*(sin(THE_Phi_pend).*sin(THE_Psi_pend)+cos(THE_Phi_pend).*cos(THE_Psi_pend).*sin(THE_Theta_pend)))./4.0)-mprop.*((cg_to_mot_L.*cos(THE_Psi).*cos(THE_Theta))./2.0+(cg_to_mot_H.*cos(THE_Theta).*sin(THE_Psi))./2.0).*(-sin(THE_Theta).*(cg_to_mot_L.*cos(THE_Psi).*cos(THE_Theta)+cg_to_mot_H.*cos(THE_Theta).*sin(THE_Psi))+cg_to_mot_H.*cos(THE_Theta).*sin(THE_Psi).*sin(THE_Theta)+cg_to_mot_L.*cos(THE_Psi).*cos(THE_Theta).*sin(THE_Theta))+mprop.*((cg_to_mot_L.*cos(THE_Psi).*cos(THE_Theta))./2.0-(cg_to_mot_H.*cos(THE_Theta).*sin(THE_Psi))./2.0).*(sin(THE_Theta).*(cg_to_mot_L.*cos(THE_Psi).*cos(THE_Theta)-cg_to_mot_H.*cos(THE_Theta).*sin(THE_Psi))+cg_to_mot_H.*cos(THE_Theta).*sin(THE_Psi).*sin(THE_Theta)-cg_to_mot_L.*cos(THE_Psi).*cos(THE_Theta).*sin(THE_Theta))-mprop.*(cg_to_mot_L.*cos(THE_Psi).*cos(THE_Theta)+cg_to_mot_H.*cos(THE_Theta).*sin(THE_Psi)).*(sin(THE_Theta).*(cg_to_mot_L.*cos(THE_Psi).*cos(THE_Theta)+cg_to_mot_H.*cos(THE_Theta).*sin(THE_Psi)).*(-1.0./2.0)+(cg_to_mot_H.*cos(THE_Theta).*sin(THE_Psi).*sin(THE_Theta))./2.0+(cg_to_mot_L.*cos(THE_Psi).*cos(THE_Theta).*sin(THE_Theta))./2.0)+mprop.*(cg_to_mot_L.*cos(THE_Psi).*cos(THE_Theta)-cg_to_mot_H.*cos(THE_Theta).*sin(THE_Psi)).*((sin(THE_Theta).*(cg_to_mot_L.*cos(THE_Psi).*cos(THE_Theta)-cg_to_mot_H.*cos(THE_Theta).*sin(THE_Psi)))./2.0+(cg_to_mot_H.*cos(THE_Theta).*sin(THE_Psi).*sin(THE_Theta))./2.0-(cg_to_mot_L.*cos(THE_Psi).*cos(THE_Theta).*sin(THE_Theta))./2.0)-(cg_to_mot_H.*mprop.*(cos(THE_Psi).*sin(THE_Phi)-cos(THE_Phi).*sin(THE_Psi).*sin(THE_Theta)).*((cg_to_mot_H.*sin(THE_Theta)+cg_to_mot_L.*cos(THE_Psi).*cos(THE_Theta)).*(cos(THE_Psi).*sin(THE_Phi)-cos(THE_Phi).*sin(THE_Psi).*sin(THE_Theta))+cg_to_mot_L.*cos(THE_Theta).*sin(THE_Psi).*(sin(THE_Phi).*sin(THE_Psi)+cos(THE_Phi).*cos(THE_Psi).*sin(THE_Theta))-cg_to_mot_H.*cos(THE_Phi).*cos(THE_Theta).^2.*sin(THE_Psi)))./2.0+(cg_to_mot_H.*mprop.*(cos(THE_Psi).*sin(THE_Phi)-cos(THE_Phi).*sin(THE_Psi).*sin(THE_Theta)).*(-(cg_to_mot_H.*sin(THE_Theta)-cg_to_mot_L.*cos(THE_Psi).*cos(THE_Theta)).*(cos(THE_Psi).*sin(THE_Phi)-cos(THE_Phi).*sin(THE_Psi).*sin(THE_Theta))+cg_to_mot_L.*cos(THE_Theta).*sin(THE_Psi).*(sin(THE_Phi).*sin(THE_Psi)+cos(THE_Phi).*cos(THE_Psi).*sin(THE_Theta))+cg_to_mot_H.*cos(THE_Phi).*cos(THE_Theta).^2.*sin(THE_Psi)))./2.0-cg_to_mot_H.*mprop.*(cos(THE_Psi).*sin(THE_Phi)-cos(THE_Phi).*sin(THE_Psi).*sin(THE_Theta)).*(((cg_to_mot_H.*sin(THE_Theta)+cg_to_mot_L.*cos(THE_Psi).*cos(THE_Theta)).*(cos(THE_Psi).*sin(THE_Phi)-cos(THE_Phi).*sin(THE_Psi).*sin(THE_Theta)))./2.0+(cg_to_mot_L.*cos(THE_Theta).*sin(THE_Psi).*(sin(THE_Phi).*sin(THE_Psi)+cos(THE_Phi).*cos(THE_Psi).*sin(THE_Theta)))./2.0-(cg_to_mot_H.*cos(THE_Phi).*cos(THE_Theta).^2.*sin(THE_Psi))./2.0)+cg_to_mot_H.*mprop.*(cos(THE_Psi).*sin(THE_Phi)-cos(THE_Phi).*sin(THE_Psi).*sin(THE_Theta)).*((cg_to_mot_H.*sin(THE_Theta)-cg_to_mot_L.*cos(THE_Psi).*cos(THE_Theta)).*(cos(THE_Psi).*sin(THE_Phi)-cos(THE_Phi).*sin(THE_Psi).*sin(THE_Theta)).*(-1.0./2.0)+(cg_to_mot_L.*cos(THE_Theta).*sin(THE_Psi).*(sin(THE_Phi).*sin(THE_Psi)+cos(THE_Phi).*cos(THE_Psi).*sin(THE_Theta)))./2.0+(cg_to_mot_H.*cos(THE_Phi).*cos(THE_Theta).^2.*sin(THE_Psi))./2.0)-(cg_to_mot_H.*mprop.*(cos(THE_Phi).*cos(THE_Psi)+sin(THE_Phi).*sin(THE_Psi).*sin(THE_Theta)).*((cg_to_mot_H.*sin(THE_Theta)+cg_to_mot_L.*cos(THE_Psi).*cos(THE_Theta)).*(cos(THE_Phi).*cos(THE_Psi)+sin(THE_Phi).*sin(THE_Psi).*sin(THE_Theta))+cg_to_mot_L.*cos(THE_Theta).*sin(THE_Psi).*(cos(THE_Phi).*sin(THE_Psi)-cos(THE_Psi).*sin(THE_Phi).*sin(THE_Theta))+cg_to_mot_H.*cos(THE_Theta).^2.*sin(THE_Phi).*sin(THE_Psi)))./2.0-(cg_to_mot_H.*mprop.*(cos(THE_Phi).*cos(THE_Psi)+sin(THE_Phi).*sin(THE_Psi).*sin(THE_Theta)).*((cg_to_mot_H.*sin(THE_Theta)-cg_to_mot_L.*cos(THE_Psi).*cos(THE_Theta)).*(cos(THE_Phi).*cos(THE_Psi)+sin(THE_Phi).*sin(THE_Psi).*sin(THE_Theta))-cg_to_mot_L.*cos(THE_Theta).*sin(THE_Psi).*(cos(THE_Phi).*sin(THE_Psi)-cos(THE_Psi).*sin(THE_Phi).*sin(THE_Theta))+cg_to_mot_H.*cos(THE_Theta).^2.*sin(THE_Phi).*sin(THE_Psi)))./2.0-cg_to_mot_H.*mprop.*(cos(THE_Phi).*cos(THE_Psi)+sin(THE_Phi).*sin(THE_Psi).*sin(THE_Theta)).*(((cg_to_mot_H.*sin(THE_Theta)+cg_to_mot_L.*cos(THE_Psi).*cos(THE_Theta)).*(cos(THE_Phi).*cos(THE_Psi)+sin(THE_Phi).*sin(THE_Psi).*sin(THE_Theta)))./2.0+(cg_to_mot_L.*cos(THE_Theta).*sin(THE_Psi).*(cos(THE_Phi).*sin(THE_Psi)-cos(THE_Psi).*sin(THE_Phi).*sin(THE_Theta)))./2.0+(cg_to_mot_H.*cos(THE_Theta).^2.*sin(THE_Phi).*sin(THE_Psi))./2.0)-cg_to_mot_H.*mprop.*(cos(THE_Phi).*cos(THE_Psi)+sin(THE_Phi).*sin(THE_Psi).*sin(THE_Theta)).*(((cg_to_mot_H.*sin(THE_Theta)-cg_to_mot_L.*cos(THE_Psi).*cos(THE_Theta)).*(cos(THE_Phi).*cos(THE_Psi)+sin(THE_Phi).*sin(THE_Psi).*sin(THE_Theta)))./2.0-(cg_to_mot_L.*cos(THE_Theta).*sin(THE_Psi).*(cos(THE_Phi).*sin(THE_Psi)-cos(THE_Psi).*sin(THE_Phi).*sin(THE_Theta)))./2.0+(cg_to_mot_H.*cos(THE_Theta).^2.*sin(THE_Phi).*sin(THE_Psi))./2.0)-m_pend.*(Lx_pend.^2./1.2e+1+Ly_pend.^2./1.2e+1).*((sin(THE_Phi_pend).*sin(THE_Psi_pend))./2.0+(cos(THE_Phi_pend).*cos(THE_Psi_pend).*sin(THE_Theta_pend))./2.0).*(sin(THE_Theta).*(sin(THE_Phi_pend).*sin(THE_Psi_pend)+cos(THE_Phi_pend).*cos(THE_Psi_pend).*sin(THE_Theta_pend))+cos(THE_Theta).*sin(THE_Psi).*(cos(THE_Phi_pend).*sin(THE_Psi_pend)-cos(THE_Psi_pend).*sin(THE_Phi_pend).*sin(THE_Theta_pend))-cos(THE_Psi).*cos(THE_Theta).*cos(THE_Psi_pend).*cos(THE_Theta_pend))-m_pend.*(Lx_pend.^2./1.2e+1+Ly_pend.^2./1.2e+1).*(sin(THE_Phi_pend).*sin(THE_Psi_pend)+cos(THE_Phi_pend).*cos(THE_Psi_pend).*sin(THE_Theta_pend)).*((sin(THE_Theta).*(sin(THE_Phi_pend).*sin(THE_Psi_pend)+cos(THE_Phi_pend).*cos(THE_Psi_pend).*sin(THE_Theta_pend)))./2.0+(cos(THE_Theta).*sin(THE_Psi).*(cos(THE_Phi_pend).*sin(THE_Psi_pend)-cos(THE_Psi_pend).*sin(THE_Phi_pend).*sin(THE_Theta_pend)))./2.0-(cos(THE_Psi).*cos(THE_Theta).*cos(THE_Psi_pend).*cos(THE_Theta_pend))./2.0)-m_pend.*(Lx_pend.^2./1.2e+1+Lz_pend.^2./1.2e+1).*((cos(THE_Psi_pend).*sin(THE_Phi_pend))./2.0-(cos(THE_Phi_pend).*sin(THE_Psi_pend).*sin(THE_Theta_pend))./2.0).*(sin(THE_Theta).*(cos(THE_Psi_pend).*sin(THE_Phi_pend)-cos(THE_Phi_pend).*sin(THE_Psi_pend).*sin(THE_Theta_pend))+cos(THE_Theta).*sin(THE_Psi).*(cos(THE_Phi_pend).*cos(THE_Psi_pend)+sin(THE_Phi_pend).*sin(THE_Psi_pend).*sin(THE_Theta_pend))+cos(THE_Psi).*cos(THE_Theta).*cos(THE_Theta_pend).*sin(THE_Psi_pend))-m_pend.*(Lx_pend.^2./1.2e+1+Lz_pend.^2./1.2e+1).*(cos(THE_Psi_pend).*sin(THE_Phi_pend)-cos(THE_Phi_pend).*sin(THE_Psi_pend).*sin(THE_Theta_pend)).*((sin(THE_Theta).*(cos(THE_Psi_pend).*sin(THE_Phi_pend)-cos(THE_Phi_pend).*sin(THE_Psi_pend).*sin(THE_Theta_pend)))./2.0+(cos(THE_Theta).*sin(THE_Psi).*(cos(THE_Phi_pend).*cos(THE_Psi_pend)+sin(THE_Phi_pend).*sin(THE_Psi_pend).*sin(THE_Theta_pend)))./2.0+(cos(THE_Psi).*cos(THE_Theta).*cos(THE_Theta_pend).*sin(THE_Psi_pend))./2.0)+(cg_to_mot_H.*mprop.*cos(THE_Theta).*sin(THE_Psi).*(-cos(THE_Theta).*sin(THE_Psi).*(cg_to_mot_H.*sin(THE_Theta)+cg_to_mot_L.*cos(THE_Psi).*cos(THE_Theta))+cg_to_mot_H.*cos(THE_Theta).*sin(THE_Psi).*sin(THE_Theta)+cg_to_mot_L.*cos(THE_Psi).*cos(THE_Theta).^2.*sin(THE_Psi)))./2.0-(cg_to_mot_H.*mprop.*cos(THE_Theta).*sin(THE_Psi).*(cos(THE_Theta).*sin(THE_Psi).*(cg_to_mot_H.*sin(THE_Theta)-cg_to_mot_L.*cos(THE_Psi).*cos(THE_Theta))-cg_to_mot_H.*cos(THE_Theta).*sin(THE_Psi).*sin(THE_Theta)+cg_to_mot_L.*cos(THE_Psi).*cos(THE_Theta).^2.*sin(THE_Psi)))./2.0+cg_to_mot_H.*mprop.*cos(THE_Theta).*sin(THE_Psi).*(cos(THE_Theta).*sin(THE_Psi).*(cg_to_mot_H.*sin(THE_Theta)+cg_to_mot_L.*cos(THE_Psi).*cos(THE_Theta)).*(-1.0./2.0)+(cg_to_mot_H.*cos(THE_Theta).*sin(THE_Psi).*sin(THE_Theta))./2.0+(cg_to_mot_L.*cos(THE_Psi).*cos(THE_Theta).^2.*sin(THE_Psi))./2.0)-cg_to_mot_H.*mprop.*cos(THE_Theta).*sin(THE_Psi).*((cos(THE_Theta).*sin(THE_Psi).*(cg_to_mot_H.*sin(THE_Theta)-cg_to_mot_L.*cos(THE_Psi).*cos(THE_Theta)))./2.0-(cg_to_mot_H.*cos(THE_Theta).*sin(THE_Psi).*sin(THE_Theta))./2.0+(cg_to_mot_L.*cos(THE_Psi).*cos(THE_Theta).^2.*sin(THE_Psi))./2.0)-(m_pend.*cos(THE_Phi_pend).*cos(THE_Theta_pend).*(Ly_pend.^2./1.2e+1+Lz_pend.^2./1.2e+1).*(cos(THE_Psi).*cos(THE_Theta).*sin(THE_Theta_pend)+cos(THE_Phi_pend).*cos(THE_Theta_pend).*sin(THE_Theta)-cos(THE_Theta).*cos(THE_Theta_pend).*sin(THE_Psi).*sin(THE_Phi_pend)))./2.0-m_pend.*cos(THE_Phi_pend).*cos(THE_Theta_pend).*(Ly_pend.^2./1.2e+1+Lz_pend.^2./1.2e+1).*((cos(THE_Psi).*cos(THE_Theta).*sin(THE_Theta_pend))./2.0+(cos(THE_Phi_pend).*cos(THE_Theta_pend).*sin(THE_Theta))./2.0-(cos(THE_Theta).*cos(THE_Theta_pend).*sin(THE_Psi).*sin(THE_Phi_pend))./2.0),mprop.*((cg_to_mot_H.*sin(THE_Theta)+cg_to_mot_L.*cos(THE_Psi).*cos(THE_Theta)).*(cos(THE_Psi).*sin(THE_Phi)-cos(THE_Phi).*sin(THE_Psi).*sin(THE_Theta))+cg_to_mot_L.*cos(THE_Theta).*sin(THE_Psi).*(sin(THE_Phi).*sin(THE_Psi)+cos(THE_Phi).*cos(THE_Psi).*sin(THE_Theta))-cg_to_mot_H.*cos(THE_Phi).*cos(THE_Theta).^2.*sin(THE_Psi)).*(-1.0./2.0)+(mprop.*(-(cg_to_mot_H.*sin(THE_Theta)-cg_to_mot_L.*cos(THE_Psi).*cos(THE_Theta)).*(cos(THE_Psi).*sin(THE_Phi)-cos(THE_Phi).*sin(THE_Psi).*sin(THE_Theta))+cg_to_mot_L.*cos(THE_Theta).*sin(THE_Psi).*(sin(THE_Phi).*sin(THE_Psi)+cos(THE_Phi).*cos(THE_Psi).*sin(THE_Theta))+cg_to_mot_H.*cos(THE_Phi).*cos(THE_Theta).^2.*sin(THE_Psi)))./2.0-mprop.*(((cg_to_mot_H.*sin(THE_Theta)+cg_to_mot_L.*cos(THE_Psi).*cos(THE_Theta)).*(cos(THE_Psi).*sin(THE_Phi)-cos(THE_Phi).*sin(THE_Psi).*sin(THE_Theta)))./2.0+(cg_to_mot_L.*cos(THE_Theta).*sin(THE_Psi).*(sin(THE_Phi).*sin(THE_Psi)+cos(THE_Phi).*cos(THE_Psi).*sin(THE_Theta)))./2.0-(cg_to_mot_H.*cos(THE_Phi).*cos(THE_Theta).^2.*sin(THE_Psi))./2.0)+mprop.*((cg_to_mot_H.*sin(THE_Theta)-cg_to_mot_L.*cos(THE_Psi).*cos(THE_Theta)).*(cos(THE_Psi).*sin(THE_Phi)-cos(THE_Phi).*sin(THE_Psi).*sin(THE_Theta)).*(-1.0./2.0)+(cg_to_mot_L.*cos(THE_Theta).*sin(THE_Psi).*(sin(THE_Phi).*sin(THE_Psi)+cos(THE_Phi).*cos(THE_Psi).*sin(THE_Theta)))./2.0+(cg_to_mot_H.*cos(THE_Phi).*cos(THE_Theta).^2.*sin(THE_Psi))./2.0)-(mprop.*(cg_to_mot_H.*sin(THE_Theta).*(cos(THE_Psi).*sin(THE_Phi)-cos(THE_Phi).*sin(THE_Psi).*sin(THE_Theta))+cg_to_mot_L.*sin(THE_Theta).*(sin(THE_Phi).*sin(THE_Psi)+cos(THE_Phi).*cos(THE_Psi).*sin(THE_Theta))+cos(THE_Phi).*cos(THE_Theta).*(cg_to_mot_L.*cos(THE_Psi).*cos(THE_Theta)-cg_to_mot_H.*cos(THE_Theta).*sin(THE_Psi))))./2.0+(mprop.*(-cg_to_mot_H.*sin(THE_Theta).*(cos(THE_Psi).*sin(THE_Phi)-cos(THE_Phi).*sin(THE_Psi).*sin(THE_Theta))+cg_to_mot_L.*sin(THE_Theta).*(sin(THE_Phi).*sin(THE_Psi)+cos(THE_Phi).*cos(THE_Psi).*sin(THE_Theta))+cos(THE_Phi).*cos(THE_Theta).*(cg_to_mot_L.*cos(THE_Psi).*cos(THE_Theta)+cg_to_mot_H.*cos(THE_Theta).*sin(THE_Psi))))./2.0+mprop.*(cg_to_mot_H.*sin(THE_Theta).*(cos(THE_Psi).*sin(THE_Phi)-cos(THE_Phi).*sin(THE_Psi).*sin(THE_Theta)).*(-1.0./2.0)+(cg_to_mot_L.*sin(THE_Theta).*(sin(THE_Phi).*sin(THE_Psi)+cos(THE_Phi).*cos(THE_Psi).*sin(THE_Theta)))./2.0+(cos(THE_Phi).*cos(THE_Theta).*(cg_to_mot_L.*cos(THE_Psi).*cos(THE_Theta)+cg_to_mot_H.*cos(THE_Theta).*sin(THE_Psi)))./2.0)-mprop.*((cg_to_mot_H.*sin(THE_Theta).*(cos(THE_Psi).*sin(THE_Phi)-cos(THE_Phi).*sin(THE_Psi).*sin(THE_Theta)))./2.0+(cg_to_mot_L.*sin(THE_Theta).*(sin(THE_Phi).*sin(THE_Psi)+cos(THE_Phi).*cos(THE_Psi).*sin(THE_Theta)))./2.0+(cos(THE_Phi).*cos(THE_Theta).*(cg_to_mot_L.*cos(THE_Psi).*cos(THE_Theta)-cg_to_mot_H.*cos(THE_Theta).*sin(THE_Psi)))./2.0)+(m_pend.*((Tv_Z_pend+(Lz_pend.*cos(THE_Psi_pend).*cos(THE_Theta_pend))./2.0).*(cos(THE_Phi).*sin(THE_Psi)-cos(THE_Psi).*sin(THE_Phi).*sin(THE_Theta))+(Lz_pend.*(cos(THE_Phi).*cos(THE_Psi)+sin(THE_Phi).*sin(THE_Psi).*sin(THE_Theta)).*(cos(THE_Phi_pend).*sin(THE_Psi_pend)-cos(THE_Psi_pend).*sin(THE_Phi_pend).*sin(THE_Theta_pend)))./2.0-(Lz_pend.*cos(THE_Theta).*sin(THE_Phi).*(sin(THE_Phi_pend).*sin(THE_Psi_pend)+cos(THE_Phi_pend).*cos(THE_Psi_pend).*sin(THE_Theta_pend)))./2.0))./2.0+m_pend.*(((Tv_Z_pend+(Lz_pend.*cos(THE_Psi_pend).*cos(THE_Theta_pend))./2.0).*(cos(THE_Phi).*sin(THE_Psi)-cos(THE_Psi).*sin(THE_Phi).*sin(THE_Theta)))./2.0+(Lz_pend.*(cos(THE_Phi).*cos(THE_Psi)+sin(THE_Phi).*sin(THE_Psi).*sin(THE_Theta)).*(cos(THE_Phi_pend).*sin(THE_Psi_pend)-cos(THE_Psi_pend).*sin(THE_Phi_pend).*sin(THE_Theta_pend)))./4.0-(Lz_pend.*cos(THE_Theta).*sin(THE_Phi).*(sin(THE_Phi_pend).*sin(THE_Psi_pend)+cos(THE_Phi_pend).*cos(THE_Psi_pend).*sin(THE_Theta_pend)))./4.0),(mprop.*((cg_to_mot_H.*sin(THE_Theta)+cg_to_mot_L.*cos(THE_Psi).*cos(THE_Theta)).*(cos(THE_Phi).*cos(THE_Psi)+sin(THE_Phi).*sin(THE_Psi).*sin(THE_Theta))+cg_to_mot_L.*cos(THE_Theta).*sin(THE_Psi).*(cos(THE_Phi).*sin(THE_Psi)-cos(THE_Psi).*sin(THE_Phi).*sin(THE_Theta))+cg_to_mot_H.*cos(THE_Theta).^2.*sin(THE_Phi).*sin(THE_Psi)))./2.0+(mprop.*((cg_to_mot_H.*sin(THE_Theta)-cg_to_mot_L.*cos(THE_Psi).*cos(THE_Theta)).*(cos(THE_Phi).*cos(THE_Psi)+sin(THE_Phi).*sin(THE_Psi).*sin(THE_Theta))-cg_to_mot_L.*cos(THE_Theta).*sin(THE_Psi).*(cos(THE_Phi).*sin(THE_Psi)-cos(THE_Psi).*sin(THE_Phi).*sin(THE_Theta))+cg_to_mot_H.*cos(THE_Theta).^2.*sin(THE_Phi).*sin(THE_Psi)))./2.0+mprop.*(((cg_to_mot_H.*sin(THE_Theta)+cg_to_mot_L.*cos(THE_Psi).*cos(THE_Theta)).*(cos(THE_Phi).*cos(THE_Psi)+sin(THE_Phi).*sin(THE_Psi).*sin(THE_Theta)))./2.0+(cg_to_mot_L.*cos(THE_Theta).*sin(THE_Psi).*(cos(THE_Phi).*sin(THE_Psi)-cos(THE_Psi).*sin(THE_Phi).*sin(THE_Theta)))./2.0+(cg_to_mot_H.*cos(THE_Theta).^2.*sin(THE_Phi).*sin(THE_Psi))./2.0)+mprop.*(((cg_to_mot_H.*sin(THE_Theta)-cg_to_mot_L.*cos(THE_Psi).*cos(THE_Theta)).*(cos(THE_Phi).*cos(THE_Psi)+sin(THE_Phi).*sin(THE_Psi).*sin(THE_Theta)))./2.0-(cg_to_mot_L.*cos(THE_Theta).*sin(THE_Psi).*(cos(THE_Phi).*sin(THE_Psi)-cos(THE_Psi).*sin(THE_Phi).*sin(THE_Theta)))./2.0+(cg_to_mot_H.*cos(THE_Theta).^2.*sin(THE_Phi).*sin(THE_Psi))./2.0)+(m_pend.*((Tv_Z_pend+(Lz_pend.*cos(THE_Psi_pend).*cos(THE_Theta_pend))./2.0).*(sin(THE_Phi).*sin(THE_Psi)+cos(THE_Phi).*cos(THE_Psi).*sin(THE_Theta))+(Lz_pend.*(cos(THE_Psi).*sin(THE_Phi)-cos(THE_Phi).*sin(THE_Psi).*sin(THE_Theta)).*(cos(THE_Phi_pend).*sin(THE_Psi_pend)-cos(THE_Psi_pend).*sin(THE_Phi_pend).*sin(THE_Theta_pend)))./2.0+(Lz_pend.*cos(THE_Phi).*cos(THE_Theta).*(sin(THE_Phi_pend).*sin(THE_Psi_pend)+cos(THE_Phi_pend).*cos(THE_Psi_pend).*sin(THE_Theta_pend)))./2.0))./2.0+m_pend.*(((Tv_Z_pend+(Lz_pend.*cos(THE_Psi_pend).*cos(THE_Theta_pend))./2.0).*(sin(THE_Phi).*sin(THE_Psi)+cos(THE_Phi).*cos(THE_Psi).*sin(THE_Theta)))./2.0+(Lz_pend.*(cos(THE_Psi).*sin(THE_Phi)-cos(THE_Phi).*sin(THE_Psi).*sin(THE_Theta)).*(cos(THE_Phi_pend).*sin(THE_Psi_pend)-cos(THE_Psi_pend).*sin(THE_Phi_pend).*sin(THE_Theta_pend)))./4.0+(Lz_pend.*cos(THE_Phi).*cos(THE_Theta).*(sin(THE_Phi_pend).*sin(THE_Psi_pend)+cos(THE_Phi_pend).*cos(THE_Psi_pend).*sin(THE_Theta_pend)))./4.0)+(mprop.*(cg_to_mot_H.*sin(THE_Theta).*(cos(THE_Phi).*cos(THE_Psi)+sin(THE_Phi).*sin(THE_Psi).*sin(THE_Theta))-cg_to_mot_L.*sin(THE_Theta).*(cos(THE_Phi).*sin(THE_Psi)-cos(THE_Psi).*sin(THE_Phi).*sin(THE_Theta))+cos(THE_Theta).*sin(THE_Phi).*(cg_to_mot_L.*cos(THE_Psi).*cos(THE_Theta)+cg_to_mot_H.*cos(THE_Theta).*sin(THE_Psi))))./2.0+(mprop.*(cg_to_mot_H.*sin(THE_Theta).*(cos(THE_Phi).*cos(THE_Psi)+sin(THE_Phi).*sin(THE_Psi).*sin(THE_Theta))+cg_to_mot_L.*sin(THE_Theta).*(cos(THE_Phi).*sin(THE_Psi)-cos(THE_Psi).*sin(THE_Phi).*sin(THE_Theta))-cos(THE_Theta).*sin(THE_Phi).*(cg_to_mot_L.*cos(THE_Psi).*cos(THE_Theta)-cg_to_mot_H.*cos(THE_Theta).*sin(THE_Psi))))./2.0+mprop.*((cg_to_mot_H.*sin(THE_Theta).*(cos(THE_Phi).*cos(THE_Psi)+sin(THE_Phi).*sin(THE_Psi).*sin(THE_Theta)))./2.0-(cg_to_mot_L.*sin(THE_Theta).*(cos(THE_Phi).*sin(THE_Psi)-cos(THE_Psi).*sin(THE_Phi).*sin(THE_Theta)))./2.0+(cos(THE_Theta).*sin(THE_Phi).*(cg_to_mot_L.*cos(THE_Psi).*cos(THE_Theta)+cg_to_mot_H.*cos(THE_Theta).*sin(THE_Psi)))./2.0)+mprop.*((cg_to_mot_H.*sin(THE_Theta).*(cos(THE_Phi).*cos(THE_Psi)+sin(THE_Phi).*sin(THE_Psi).*sin(THE_Theta)))./2.0+(cg_to_mot_L.*sin(THE_Theta).*(cos(THE_Phi).*sin(THE_Psi)-cos(THE_Psi).*sin(THE_Phi).*sin(THE_Theta)))./2.0-(cos(THE_Theta).*sin(THE_Phi).*(cg_to_mot_L.*cos(THE_Psi).*cos(THE_Theta)-cg_to_mot_H.*cos(THE_Theta).*sin(THE_Psi)))./2.0),(mprop.*(-sin(THE_Theta).*(cg_to_mot_L.*cos(THE_Psi).*cos(THE_Theta)+cg_to_mot_H.*cos(THE_Theta).*sin(THE_Psi))+cg_to_mot_H.*cos(THE_Theta).*sin(THE_Psi).*sin(THE_Theta)+cg_to_mot_L.*cos(THE_Psi).*cos(THE_Theta).*sin(THE_Theta)))./2.0+(mprop.*(sin(THE_Theta).*(cg_to_mot_L.*cos(THE_Psi).*cos(THE_Theta)-cg_to_mot_H.*cos(THE_Theta).*sin(THE_Psi))+cg_to_mot_H.*cos(THE_Theta).*sin(THE_Psi).*sin(THE_Theta)-cg_to_mot_L.*cos(THE_Psi).*cos(THE_Theta).*sin(THE_Theta)))./2.0+mprop.*(sin(THE_Theta).*(cg_to_mot_L.*cos(THE_Psi).*cos(THE_Theta)+cg_to_mot_H.*cos(THE_Theta).*sin(THE_Psi)).*(-1.0./2.0)+(cg_to_mot_H.*cos(THE_Theta).*sin(THE_Psi).*sin(THE_Theta))./2.0+(cg_to_mot_L.*cos(THE_Psi).*cos(THE_Theta).*sin(THE_Theta))./2.0)+mprop.*((sin(THE_Theta).*(cg_to_mot_L.*cos(THE_Psi).*cos(THE_Theta)-cg_to_mot_H.*cos(THE_Theta).*sin(THE_Psi)))./2.0+(cg_to_mot_H.*cos(THE_Theta).*sin(THE_Psi).*sin(THE_Theta))./2.0-(cg_to_mot_L.*cos(THE_Psi).*cos(THE_Theta).*sin(THE_Theta))./2.0)-(mprop.*(-cos(THE_Theta).*sin(THE_Psi).*(cg_to_mot_H.*sin(THE_Theta)+cg_to_mot_L.*cos(THE_Psi).*cos(THE_Theta))+cg_to_mot_H.*cos(THE_Theta).*sin(THE_Psi).*sin(THE_Theta)+cg_to_mot_L.*cos(THE_Psi).*cos(THE_Theta).^2.*sin(THE_Psi)))./2.0+(mprop.*(cos(THE_Theta).*sin(THE_Psi).*(cg_to_mot_H.*sin(THE_Theta)-cg_to_mot_L.*cos(THE_Psi).*cos(THE_Theta))-cg_to_mot_H.*cos(THE_Theta).*sin(THE_Psi).*sin(THE_Theta)+cg_to_mot_L.*cos(THE_Psi).*cos(THE_Theta).^2.*sin(THE_Psi)))./2.0-mprop.*(cos(THE_Theta).*sin(THE_Psi).*(cg_to_mot_H.*sin(THE_Theta)+cg_to_mot_L.*cos(THE_Psi).*cos(THE_Theta)).*(-1.0./2.0)+(cg_to_mot_H.*cos(THE_Theta).*sin(THE_Psi).*sin(THE_Theta))./2.0+(cg_to_mot_L.*cos(THE_Psi).*cos(THE_Theta).^2.*sin(THE_Psi))./2.0)+mprop.*((cos(THE_Theta).*sin(THE_Psi).*(cg_to_mot_H.*sin(THE_Theta)-cg_to_mot_L.*cos(THE_Psi).*cos(THE_Theta)))./2.0-(cg_to_mot_H.*cos(THE_Theta).*sin(THE_Psi).*sin(THE_Theta))./2.0+(cg_to_mot_L.*cos(THE_Psi).*cos(THE_Theta).^2.*sin(THE_Psi))./2.0),m_pend.*((Lz_pend.*(cos(THE_Phi).*cos(THE_Psi)+sin(THE_Phi).*sin(THE_Psi).*sin(THE_Theta)).*(sin(THE_Phi_pend).*sin(THE_Psi_pend)+cos(THE_Phi_pend).*cos(THE_Psi_pend).*sin(THE_Theta_pend)))./4.0+(Lz_pend.*cos(THE_Theta).*sin(THE_Phi).*(cos(THE_Phi_pend).*sin(THE_Psi_pend)-cos(THE_Psi_pend).*sin(THE_Phi_pend).*sin(THE_Theta_pend)))./4.0).*((Tv_Z_pend+(Lz_pend.*cos(THE_Psi_pend).*cos(THE_Theta_pend))./2.0).*(sin(THE_Phi).*sin(THE_Psi)+cos(THE_Phi).*cos(THE_Psi).*sin(THE_Theta))+(Lz_pend.*(cos(THE_Psi).*sin(THE_Phi)-cos(THE_Phi).*sin(THE_Psi).*sin(THE_Theta)).*(cos(THE_Phi_pend).*sin(THE_Psi_pend)-cos(THE_Psi_pend).*sin(THE_Phi_pend).*sin(THE_Theta_pend)))./2.0+(Lz_pend.*cos(THE_Phi).*cos(THE_Theta).*(sin(THE_Phi_pend).*sin(THE_Psi_pend)+cos(THE_Phi_pend).*cos(THE_Psi_pend).*sin(THE_Theta_pend)))./2.0)-m_pend.*((Lz_pend.*(cos(THE_Psi).*sin(THE_Phi)-cos(THE_Phi).*sin(THE_Psi).*sin(THE_Theta)).*(sin(THE_Phi_pend).*sin(THE_Psi_pend)+cos(THE_Phi_pend).*cos(THE_Psi_pend).*sin(THE_Theta_pend)))./4.0-(Lz_pend.*cos(THE_Phi).*cos(THE_Theta).*(cos(THE_Phi_pend).*sin(THE_Psi_pend)-cos(THE_Psi_pend).*sin(THE_Phi_pend).*sin(THE_Theta_pend)))./4.0).*((Tv_Z_pend+(Lz_pend.*cos(THE_Psi_pend).*cos(THE_Theta_pend))./2.0).*(cos(THE_Phi).*sin(THE_Psi)-cos(THE_Psi).*sin(THE_Phi).*sin(THE_Theta))+(Lz_pend.*(cos(THE_Phi).*cos(THE_Psi)+sin(THE_Phi).*sin(THE_Psi).*sin(THE_Theta)).*(cos(THE_Phi_pend).*sin(THE_Psi_pend)-cos(THE_Psi_pend).*sin(THE_Phi_pend).*sin(THE_Theta_pend)))./2.0-(Lz_pend.*cos(THE_Theta).*sin(THE_Phi).*(sin(THE_Phi_pend).*sin(THE_Psi_pend)+cos(THE_Phi_pend).*cos(THE_Psi_pend).*sin(THE_Theta_pend)))./2.0)+m_pend.*((Lz_pend.*(cos(THE_Phi).*cos(THE_Psi)+sin(THE_Phi).*sin(THE_Psi).*sin(THE_Theta)).*(sin(THE_Phi_pend).*sin(THE_Psi_pend)+cos(THE_Phi_pend).*cos(THE_Psi_pend).*sin(THE_Theta_pend)))./2.0+(Lz_pend.*cos(THE_Theta).*sin(THE_Phi).*(cos(THE_Phi_pend).*sin(THE_Psi_pend)-cos(THE_Psi_pend).*sin(THE_Phi_pend).*sin(THE_Theta_pend)))./2.0).*(((Tv_Z_pend+(Lz_pend.*cos(THE_Psi_pend).*cos(THE_Theta_pend))./2.0).*(sin(THE_Phi).*sin(THE_Psi)+cos(THE_Phi).*cos(THE_Psi).*sin(THE_Theta)))./2.0+(Lz_pend.*(cos(THE_Psi).*sin(THE_Phi)-cos(THE_Phi).*sin(THE_Psi).*sin(THE_Theta)).*(cos(THE_Phi_pend).*sin(THE_Psi_pend)-cos(THE_Psi_pend).*sin(THE_Phi_pend).*sin(THE_Theta_pend)))./4.0+(Lz_pend.*cos(THE_Phi).*cos(THE_Theta).*(sin(THE_Phi_pend).*sin(THE_Psi_pend)+cos(THE_Phi_pend).*cos(THE_Psi_pend).*sin(THE_Theta_pend)))./4.0)-m_pend.*((Lz_pend.*(cos(THE_Psi).*sin(THE_Phi)-cos(THE_Phi).*sin(THE_Psi).*sin(THE_Theta)).*(sin(THE_Phi_pend).*sin(THE_Psi_pend)+cos(THE_Phi_pend).*cos(THE_Psi_pend).*sin(THE_Theta_pend)))./2.0-(Lz_pend.*cos(THE_Phi).*cos(THE_Theta).*(cos(THE_Phi_pend).*sin(THE_Psi_pend)-cos(THE_Psi_pend).*sin(THE_Phi_pend).*sin(THE_Theta_pend)))./2.0).*(((Tv_Z_pend+(Lz_pend.*cos(THE_Psi_pend).*cos(THE_Theta_pend))./2.0).*(cos(THE_Phi).*sin(THE_Psi)-cos(THE_Psi).*sin(THE_Phi).*sin(THE_Theta)))./2.0+(Lz_pend.*(cos(THE_Phi).*cos(THE_Psi)+sin(THE_Phi).*sin(THE_Psi).*sin(THE_Theta)).*(cos(THE_Phi_pend).*sin(THE_Psi_pend)-cos(THE_Psi_pend).*sin(THE_Phi_pend).*sin(THE_Theta_pend)))./4.0-(Lz_pend.*cos(THE_Theta).*sin(THE_Phi).*(sin(THE_Phi_pend).*sin(THE_Psi_pend)+cos(THE_Phi_pend).*cos(THE_Psi_pend).*sin(THE_Theta_pend)))./4.0)+(m_pend.*sin(THE_Theta_pend).*(Ly_pend.^2./1.2e+1+Lz_pend.^2./1.2e+1).*(cos(THE_Psi).*cos(THE_Theta).*sin(THE_Theta_pend)+cos(THE_Phi_pend).*cos(THE_Theta_pend).*sin(THE_Theta)-cos(THE_Theta).*cos(THE_Theta_pend).*sin(THE_Psi).*sin(THE_Phi_pend)))./2.0+m_pend.*sin(THE_Theta_pend).*(Ly_pend.^2./1.2e+1+Lz_pend.^2./1.2e+1).*((cos(THE_Psi).*cos(THE_Theta).*sin(THE_Theta_pend))./2.0+(cos(THE_Phi_pend).*cos(THE_Theta_pend).*sin(THE_Theta))./2.0-(cos(THE_Theta).*cos(THE_Theta_pend).*sin(THE_Psi).*sin(THE_Phi_pend))./2.0)-(m_pend.*cos(THE_Psi_pend).*cos(THE_Theta_pend).*(Lx_pend.^2./1.2e+1+Ly_pend.^2./1.2e+1).*(sin(THE_Theta).*(sin(THE_Phi_pend).*sin(THE_Psi_pend)+cos(THE_Phi_pend).*cos(THE_Psi_pend).*sin(THE_Theta_pend))+cos(THE_Theta).*sin(THE_Psi).*(cos(THE_Phi_pend).*sin(THE_Psi_pend)-cos(THE_Psi_pend).*sin(THE_Phi_pend).*sin(THE_Theta_pend))-cos(THE_Psi).*cos(THE_Theta).*cos(THE_Psi_pend).*cos(THE_Theta_pend)))./2.0-m_pend.*cos(THE_Psi_pend).*cos(THE_Theta_pend).*(Lx_pend.^2./1.2e+1+Ly_pend.^2./1.2e+1).*((sin(THE_Theta).*(sin(THE_Phi_pend).*sin(THE_Psi_pend)+cos(THE_Phi_pend).*cos(THE_Psi_pend).*sin(THE_Theta_pend)))./2.0+(cos(THE_Theta).*sin(THE_Psi).*(cos(THE_Phi_pend).*sin(THE_Psi_pend)-cos(THE_Psi_pend).*sin(THE_Phi_pend).*sin(THE_Theta_pend)))./2.0-(cos(THE_Psi).*cos(THE_Theta).*cos(THE_Psi_pend).*cos(THE_Theta_pend))./2.0)+(m_pend.*cos(THE_Theta_pend).*sin(THE_Psi_pend).*(Lx_pend.^2./1.2e+1+Lz_pend.^2./1.2e+1).*(sin(THE_Theta).*(cos(THE_Psi_pend).*sin(THE_Phi_pend)-cos(THE_Phi_pend).*sin(THE_Psi_pend).*sin(THE_Theta_pend))+cos(THE_Theta).*sin(THE_Psi).*(cos(THE_Phi_pend).*cos(THE_Psi_pend)+sin(THE_Phi_pend).*sin(THE_Psi_pend).*sin(THE_Theta_pend))+cos(THE_Psi).*cos(THE_Theta).*cos(THE_Theta_pend).*sin(THE_Psi_pend)))./2.0+m_pend.*cos(THE_Theta_pend).*sin(THE_Psi_pend).*(Lx_pend.^2./1.2e+1+Lz_pend.^2./1.2e+1).*((sin(THE_Theta).*(cos(THE_Psi_pend).*sin(THE_Phi_pend)-cos(THE_Phi_pend).*sin(THE_Psi_pend).*sin(THE_Theta_pend)))./2.0+(cos(THE_Theta).*sin(THE_Psi).*(cos(THE_Phi_pend).*cos(THE_Psi_pend)+sin(THE_Phi_pend).*sin(THE_Psi_pend).*sin(THE_Theta_pend)))./2.0+(cos(THE_Psi).*cos(THE_Theta).*cos(THE_Theta_pend).*sin(THE_Psi_pend))./2.0),-m_pend.*((Lz_pend.*cos(THE_Psi_pend).*sin(THE_Theta_pend).*(sin(THE_Phi).*sin(THE_Psi)+cos(THE_Phi).*cos(THE_Psi).*sin(THE_Theta)))./4.0+(Lz_pend.*cos(THE_Psi_pend).*cos(THE_Theta_pend).*sin(THE_Phi_pend).*(cos(THE_Psi).*sin(THE_Phi)-cos(THE_Phi).*sin(THE_Psi).*sin(THE_Theta)))./4.0-(Lz_pend.*cos(THE_Phi).*cos(THE_Theta).*cos(THE_Phi_pend).*cos(THE_Psi_pend).*cos(THE_Theta_pend))./4.0).*((Tv_Z_pend+(Lz_pend.*cos(THE_Psi_pend).*cos(THE_Theta_pend))./2.0).*(cos(THE_Phi).*sin(THE_Psi)-cos(THE_Psi).*sin(THE_Phi).*sin(THE_Theta))+(Lz_pend.*(cos(THE_Phi).*cos(THE_Psi)+sin(THE_Phi).*sin(THE_Psi).*sin(THE_Theta)).*(cos(THE_Phi_pend).*sin(THE_Psi_pend)-cos(THE_Psi_pend).*sin(THE_Phi_pend).*sin(THE_Theta_pend)))./2.0-(Lz_pend.*cos(THE_Theta).*sin(THE_Phi).*(sin(THE_Phi_pend).*sin(THE_Psi_pend)+cos(THE_Phi_pend).*cos(THE_Psi_pend).*sin(THE_Theta_pend)))./2.0)+m_pend.*((Lz_pend.*cos(THE_Psi_pend).*sin(THE_Theta_pend).*(cos(THE_Phi).*sin(THE_Psi)-cos(THE_Psi).*sin(THE_Phi).*sin(THE_Theta)))./4.0+(Lz_pend.*cos(THE_Psi_pend).*cos(THE_Theta_pend).*sin(THE_Phi_pend).*(cos(THE_Phi).*cos(THE_Psi)+sin(THE_Phi).*sin(THE_Psi).*sin(THE_Theta)))./4.0+(Lz_pend.*cos(THE_Theta).*cos(THE_Phi_pend).*cos(THE_Psi_pend).*cos(THE_Theta_pend).*sin(THE_Phi))./4.0).*((Tv_Z_pend+(Lz_pend.*cos(THE_Psi_pend).*cos(THE_Theta_pend))./2.0).*(sin(THE_Phi).*sin(THE_Psi)+cos(THE_Phi).*cos(THE_Psi).*sin(THE_Theta))+(Lz_pend.*(cos(THE_Psi).*sin(THE_Phi)-cos(THE_Phi).*sin(THE_Psi).*sin(THE_Theta)).*(cos(THE_Phi_pend).*sin(THE_Psi_pend)-cos(THE_Psi_pend).*sin(THE_Phi_pend).*sin(THE_Theta_pend)))./2.0+(Lz_pend.*cos(THE_Phi).*cos(THE_Theta).*(sin(THE_Phi_pend).*sin(THE_Psi_pend)+cos(THE_Phi_pend).*cos(THE_Psi_pend).*sin(THE_Theta_pend)))./2.0)-m_pend.*((Lz_pend.*cos(THE_Psi_pend).*sin(THE_Theta_pend).*(sin(THE_Phi).*sin(THE_Psi)+cos(THE_Phi).*cos(THE_Psi).*sin(THE_Theta)))./2.0+(Lz_pend.*cos(THE_Psi_pend).*cos(THE_Theta_pend).*sin(THE_Phi_pend).*(cos(THE_Psi).*sin(THE_Phi)-cos(THE_Phi).*sin(THE_Psi).*sin(THE_Theta)))./2.0-(Lz_pend.*cos(THE_Phi).*cos(THE_Theta).*cos(THE_Phi_pend).*cos(THE_Psi_pend).*cos(THE_Theta_pend))./2.0).*(((Tv_Z_pend+(Lz_pend.*cos(THE_Psi_pend).*cos(THE_Theta_pend))./2.0).*(cos(THE_Phi).*sin(THE_Psi)-cos(THE_Psi).*sin(THE_Phi).*sin(THE_Theta)))./2.0+(Lz_pend.*(cos(THE_Phi).*cos(THE_Psi)+sin(THE_Phi).*sin(THE_Psi).*sin(THE_Theta)).*(cos(THE_Phi_pend).*sin(THE_Psi_pend)-cos(THE_Psi_pend).*sin(THE_Phi_pend).*sin(THE_Theta_pend)))./4.0-(Lz_pend.*cos(THE_Theta).*sin(THE_Phi).*(sin(THE_Phi_pend).*sin(THE_Psi_pend)+cos(THE_Phi_pend).*cos(THE_Psi_pend).*sin(THE_Theta_pend)))./4.0)+m_pend.*((Lz_pend.*cos(THE_Psi_pend).*sin(THE_Theta_pend).*(cos(THE_Phi).*sin(THE_Psi)-cos(THE_Psi).*sin(THE_Phi).*sin(THE_Theta)))./2.0+(Lz_pend.*cos(THE_Psi_pend).*cos(THE_Theta_pend).*sin(THE_Phi_pend).*(cos(THE_Phi).*cos(THE_Psi)+sin(THE_Phi).*sin(THE_Psi).*sin(THE_Theta)))./2.0+(Lz_pend.*cos(THE_Theta).*cos(THE_Phi_pend).*cos(THE_Psi_pend).*cos(THE_Theta_pend).*sin(THE_Phi))./2.0).*(((Tv_Z_pend+(Lz_pend.*cos(THE_Psi_pend).*cos(THE_Theta_pend))./2.0).*(sin(THE_Phi).*sin(THE_Psi)+cos(THE_Phi).*cos(THE_Psi).*sin(THE_Theta)))./2.0+(Lz_pend.*(cos(THE_Psi).*sin(THE_Phi)-cos(THE_Phi).*sin(THE_Psi).*sin(THE_Theta)).*(cos(THE_Phi_pend).*sin(THE_Psi_pend)-cos(THE_Psi_pend).*sin(THE_Phi_pend).*sin(THE_Theta_pend)))./4.0+(Lz_pend.*cos(THE_Phi).*cos(THE_Theta).*(sin(THE_Phi_pend).*sin(THE_Psi_pend)+cos(THE_Phi_pend).*cos(THE_Psi_pend).*sin(THE_Theta_pend)))./4.0)+(m_pend.*sin(THE_Psi_pend).*(Lx_pend.^2./1.2e+1+Ly_pend.^2./1.2e+1).*(sin(THE_Theta).*(sin(THE_Phi_pend).*sin(THE_Psi_pend)+cos(THE_Phi_pend).*cos(THE_Psi_pend).*sin(THE_Theta_pend))+cos(THE_Theta).*sin(THE_Psi).*(cos(THE_Phi_pend).*sin(THE_Psi_pend)-cos(THE_Psi_pend).*sin(THE_Phi_pend).*sin(THE_Theta_pend))-cos(THE_Psi).*cos(THE_Theta).*cos(THE_Psi_pend).*cos(THE_Theta_pend)))./2.0+m_pend.*sin(THE_Psi_pend).*(Lx_pend.^2./1.2e+1+Ly_pend.^2./1.2e+1).*((sin(THE_Theta).*(sin(THE_Phi_pend).*sin(THE_Psi_pend)+cos(THE_Phi_pend).*cos(THE_Psi_pend).*sin(THE_Theta_pend)))./2.0+(cos(THE_Theta).*sin(THE_Psi).*(cos(THE_Phi_pend).*sin(THE_Psi_pend)-cos(THE_Psi_pend).*sin(THE_Phi_pend).*sin(THE_Theta_pend)))./2.0-(cos(THE_Psi).*cos(THE_Theta).*cos(THE_Psi_pend).*cos(THE_Theta_pend))./2.0)+(m_pend.*cos(THE_Psi_pend).*(Lx_pend.^2./1.2e+1+Lz_pend.^2./1.2e+1).*(sin(THE_Theta).*(cos(THE_Psi_pend).*sin(THE_Phi_pend)-cos(THE_Phi_pend).*sin(THE_Psi_pend).*sin(THE_Theta_pend))+cos(THE_Theta).*sin(THE_Psi).*(cos(THE_Phi_pend).*cos(THE_Psi_pend)+sin(THE_Phi_pend).*sin(THE_Psi_pend).*sin(THE_Theta_pend))+cos(THE_Psi).*cos(THE_Theta).*cos(THE_Theta_pend).*sin(THE_Psi_pend)))./2.0+m_pend.*cos(THE_Psi_pend).*(Lx_pend.^2./1.2e+1+Lz_pend.^2./1.2e+1).*((sin(THE_Theta).*(cos(THE_Psi_pend).*sin(THE_Phi_pend)-cos(THE_Phi_pend).*sin(THE_Psi_pend).*sin(THE_Theta_pend)))./2.0+(cos(THE_Theta).*sin(THE_Psi).*(cos(THE_Phi_pend).*cos(THE_Psi_pend)+sin(THE_Phi_pend).*sin(THE_Psi_pend).*sin(THE_Theta_pend)))./2.0+(cos(THE_Psi).*cos(THE_Theta).*cos(THE_Theta_pend).*sin(THE_Psi_pend))./2.0),m_pend.*(Ly_pend.^2./1.2e+1+Lz_pend.^2./1.2e+1).*(cos(THE_Psi).*cos(THE_Theta).*sin(THE_Theta_pend)+cos(THE_Phi_pend).*cos(THE_Theta_pend).*sin(THE_Theta)-cos(THE_Theta).*cos(THE_Theta_pend).*sin(THE_Psi).*sin(THE_Phi_pend)).*(-1.0./2.0)-m_pend.*(Ly_pend.^2./1.2e+1+Lz_pend.^2./1.2e+1).*((cos(THE_Psi).*cos(THE_Theta).*sin(THE_Theta_pend))./2.0+(cos(THE_Phi_pend).*cos(THE_Theta_pend).*sin(THE_Theta))./2.0-(cos(THE_Theta).*cos(THE_Theta_pend).*sin(THE_Psi).*sin(THE_Phi_pend))./2.0)+m_pend.*((Lz_pend.*(cos(THE_Psi).*sin(THE_Phi)-cos(THE_Phi).*sin(THE_Psi).*sin(THE_Theta)).*(cos(THE_Phi_pend).*cos(THE_Psi_pend)+sin(THE_Phi_pend).*sin(THE_Psi_pend).*sin(THE_Theta_pend)))./4.0+(Lz_pend.*cos(THE_Phi).*cos(THE_Theta).*(cos(THE_Psi_pend).*sin(THE_Phi_pend)-cos(THE_Phi_pend).*sin(THE_Psi_pend).*sin(THE_Theta_pend)))./4.0-(Lz_pend.*cos(THE_Theta_pend).*sin(THE_Psi_pend).*(sin(THE_Phi).*sin(THE_Psi)+cos(THE_Phi).*cos(THE_Psi).*sin(THE_Theta)))./4.0).*((Tv_Z_pend+(Lz_pend.*cos(THE_Psi_pend).*cos(THE_Theta_pend))./2.0).*(cos(THE_Phi).*sin(THE_Psi)-cos(THE_Psi).*sin(THE_Phi).*sin(THE_Theta))+(Lz_pend.*(cos(THE_Phi).*cos(THE_Psi)+sin(THE_Phi).*sin(THE_Psi).*sin(THE_Theta)).*(cos(THE_Phi_pend).*sin(THE_Psi_pend)-cos(THE_Psi_pend).*sin(THE_Phi_pend).*sin(THE_Theta_pend)))./2.0-(Lz_pend.*cos(THE_Theta).*sin(THE_Phi).*(sin(THE_Phi_pend).*sin(THE_Psi_pend)+cos(THE_Phi_pend).*cos(THE_Psi_pend).*sin(THE_Theta_pend)))./2.0)+m_pend.*((Tv_Z_pend+(Lz_pend.*cos(THE_Psi_pend).*cos(THE_Theta_pend))./2.0).*(sin(THE_Phi).*sin(THE_Psi)+cos(THE_Phi).*cos(THE_Psi).*sin(THE_Theta))+(Lz_pend.*(cos(THE_Psi).*sin(THE_Phi)-cos(THE_Phi).*sin(THE_Psi).*sin(THE_Theta)).*(cos(THE_Phi_pend).*sin(THE_Psi_pend)-cos(THE_Psi_pend).*sin(THE_Phi_pend).*sin(THE_Theta_pend)))./2.0+(Lz_pend.*cos(THE_Phi).*cos(THE_Theta).*(sin(THE_Phi_pend).*sin(THE_Psi_pend)+cos(THE_Phi_pend).*cos(THE_Psi_pend).*sin(THE_Theta_pend)))./2.0).*(Lz_pend.*(cos(THE_Phi).*cos(THE_Psi)+sin(THE_Phi).*sin(THE_Psi).*sin(THE_Theta)).*(cos(THE_Phi_pend).*cos(THE_Psi_pend)+sin(THE_Phi_pend).*sin(THE_Psi_pend).*sin(THE_Theta_pend)).*(-1.0./4.0)+(Lz_pend.*cos(THE_Theta_pend).*sin(THE_Psi_pend).*(cos(THE_Phi).*sin(THE_Psi)-cos(THE_Psi).*sin(THE_Phi).*sin(THE_Theta)))./4.0+(Lz_pend.*cos(THE_Theta).*sin(THE_Phi).*(cos(THE_Psi_pend).*sin(THE_Phi_pend)-cos(THE_Phi_pend).*sin(THE_Psi_pend).*sin(THE_Theta_pend)))./4.0)+m_pend.*((Lz_pend.*(cos(THE_Psi).*sin(THE_Phi)-cos(THE_Phi).*sin(THE_Psi).*sin(THE_Theta)).*(cos(THE_Phi_pend).*cos(THE_Psi_pend)+sin(THE_Phi_pend).*sin(THE_Psi_pend).*sin(THE_Theta_pend)))./2.0+(Lz_pend.*cos(THE_Phi).*cos(THE_Theta).*(cos(THE_Psi_pend).*sin(THE_Phi_pend)-cos(THE_Phi_pend).*sin(THE_Psi_pend).*sin(THE_Theta_pend)))./2.0-(Lz_pend.*cos(THE_Theta_pend).*sin(THE_Psi_pend).*(sin(THE_Phi).*sin(THE_Psi)+cos(THE_Phi).*cos(THE_Psi).*sin(THE_Theta)))./2.0).*(((Tv_Z_pend+(Lz_pend.*cos(THE_Psi_pend).*cos(THE_Theta_pend))./2.0).*(cos(THE_Phi).*sin(THE_Psi)-cos(THE_Psi).*sin(THE_Phi).*sin(THE_Theta)))./2.0+(Lz_pend.*(cos(THE_Phi).*cos(THE_Psi)+sin(THE_Phi).*sin(THE_Psi).*sin(THE_Theta)).*(cos(THE_Phi_pend).*sin(THE_Psi_pend)-cos(THE_Psi_pend).*sin(THE_Phi_pend).*sin(THE_Theta_pend)))./4.0-(Lz_pend.*cos(THE_Theta).*sin(THE_Phi).*(sin(THE_Phi_pend).*sin(THE_Psi_pend)+cos(THE_Phi_pend).*cos(THE_Psi_pend).*sin(THE_Theta_pend)))./4.0)+m_pend.*(((Tv_Z_pend+(Lz_pend.*cos(THE_Psi_pend).*cos(THE_Theta_pend))./2.0).*(sin(THE_Phi).*sin(THE_Psi)+cos(THE_Phi).*cos(THE_Psi).*sin(THE_Theta)))./2.0+(Lz_pend.*(cos(THE_Psi).*sin(THE_Phi)-cos(THE_Phi).*sin(THE_Psi).*sin(THE_Theta)).*(cos(THE_Phi_pend).*sin(THE_Psi_pend)-cos(THE_Psi_pend).*sin(THE_Phi_pend).*sin(THE_Theta_pend)))./4.0+(Lz_pend.*cos(THE_Phi).*cos(THE_Theta).*(sin(THE_Phi_pend).*sin(THE_Psi_pend)+cos(THE_Phi_pend).*cos(THE_Psi_pend).*sin(THE_Theta_pend)))./4.0).*(Lz_pend.*(cos(THE_Phi).*cos(THE_Psi)+sin(THE_Phi).*sin(THE_Psi).*sin(THE_Theta)).*(cos(THE_Phi_pend).*cos(THE_Psi_pend)+sin(THE_Phi_pend).*sin(THE_Psi_pend).*sin(THE_Theta_pend)).*(-1.0./2.0)+(Lz_pend.*cos(THE_Theta_pend).*sin(THE_Psi_pend).*(cos(THE_Phi).*sin(THE_Psi)-cos(THE_Psi).*sin(THE_Phi).*sin(THE_Theta)))./2.0+(Lz_pend.*cos(THE_Theta).*sin(THE_Phi).*(cos(THE_Psi_pend).*sin(THE_Phi_pend)-cos(THE_Phi_pend).*sin(THE_Psi_pend).*sin(THE_Theta_pend)))./2.0),cos(THE_Psi).*(I_xy.*sin(THE_Theta).*(-1.0./2.0)+(I_yz.*cos(THE_Psi).*cos(THE_Theta))./2.0+(I_yy.*cos(THE_Theta).*sin(THE_Psi))./2.0)+cos(THE_Psi).*(Iprop_xy.*sin(THE_Theta).*(-1.0./2.0)+(Iprop_yz.*cos(THE_Psi).*cos(THE_Theta))./2.0+(Iprop_yy.*cos(THE_Theta).*sin(THE_Psi))./2.0).*4.0-sin(THE_Psi).*(I_xz.*sin(THE_Theta).*(-1.0./2.0)+(I_zz.*cos(THE_Psi).*cos(THE_Theta))./2.0+(I_yz.*cos(THE_Theta).*sin(THE_Psi))./2.0)-sin(THE_Psi).*(Iprop_xz.*sin(THE_Theta).*(-1.0./2.0)+(Iprop_zz.*cos(THE_Psi).*cos(THE_Theta))./2.0+(Iprop_yz.*cos(THE_Theta).*sin(THE_Psi))./2.0).*4.0-sin(THE_Theta).*((I_xy.*cos(THE_Psi))./2.0-(I_xz.*sin(THE_Psi))./2.0)-sin(THE_Theta).*((Iprop_xy.*cos(THE_Psi))./2.0-(Iprop_xz.*sin(THE_Psi))./2.0).*4.0+cos(THE_Theta).*sin(THE_Psi).*((I_yy.*cos(THE_Psi))./2.0-(I_yz.*sin(THE_Psi))./2.0)+cos(THE_Theta).*sin(THE_Psi).*((Iprop_yy.*cos(THE_Psi))./2.0-(Iprop_yz.*sin(THE_Psi))./2.0).*4.0-mprop.*(-cg_to_mot_L.*cos(THE_Psi).*(sin(THE_Phi).*sin(THE_Psi)+cos(THE_Phi).*cos(THE_Psi).*sin(THE_Theta))+cg_to_mot_L.*sin(THE_Psi).*(cos(THE_Psi).*sin(THE_Phi)-cos(THE_Phi).*sin(THE_Psi).*sin(THE_Theta))+cg_to_mot_H.*cos(THE_Phi).*cos(THE_Psi).*cos(THE_Theta)).*(((cg_to_mot_H.*sin(THE_Theta)+cg_to_mot_L.*cos(THE_Psi).*cos(THE_Theta)).*(cos(THE_Psi).*sin(THE_Phi)-cos(THE_Phi).*sin(THE_Psi).*sin(THE_Theta)))./2.0+(cg_to_mot_L.*cos(THE_Theta).*sin(THE_Psi).*(sin(THE_Phi).*sin(THE_Psi)+cos(THE_Phi).*cos(THE_Psi).*sin(THE_Theta)))./2.0-(cg_to_mot_H.*cos(THE_Phi).*cos(THE_Theta).^2.*sin(THE_Psi))./2.0)-mprop.*(cg_to_mot_L.*cos(THE_Psi).*(sin(THE_Phi).*sin(THE_Psi)+cos(THE_Phi).*cos(THE_Psi).*sin(THE_Theta)).*(-1.0./2.0)+(cg_to_mot_L.*sin(THE_Psi).*(cos(THE_Psi).*sin(THE_Phi)-cos(THE_Phi).*sin(THE_Psi).*sin(THE_Theta)))./2.0+(cg_to_mot_H.*cos(THE_Phi).*cos(THE_Psi).*cos(THE_Theta))./2.0).*((cg_to_mot_H.*sin(THE_Theta)+cg_to_mot_L.*cos(THE_Psi).*cos(THE_Theta)).*(cos(THE_Psi).*sin(THE_Phi)-cos(THE_Phi).*sin(THE_Psi).*sin(THE_Theta))+cg_to_mot_L.*cos(THE_Theta).*sin(THE_Psi).*(sin(THE_Phi).*sin(THE_Psi)+cos(THE_Phi).*cos(THE_Psi).*sin(THE_Theta))-cg_to_mot_H.*cos(THE_Phi).*cos(THE_Theta).^2.*sin(THE_Psi))+mprop.*(cg_to_mot_L.*cos(THE_Psi).*(sin(THE_Phi).*sin(THE_Psi)+cos(THE_Phi).*cos(THE_Psi).*sin(THE_Theta))-cg_to_mot_L.*sin(THE_Psi).*(cos(THE_Psi).*sin(THE_Phi)-cos(THE_Phi).*sin(THE_Psi).*sin(THE_Theta))+cg_to_mot_H.*cos(THE_Phi).*cos(THE_Psi).*cos(THE_Theta)).*((cg_to_mot_H.*sin(THE_Theta)-cg_to_mot_L.*cos(THE_Psi).*cos(THE_Theta)).*(cos(THE_Psi).*sin(THE_Phi)-cos(THE_Phi).*sin(THE_Psi).*sin(THE_Theta)).*(-1.0./2.0)+(cg_to_mot_L.*cos(THE_Theta).*sin(THE_Psi).*(sin(THE_Phi).*sin(THE_Psi)+cos(THE_Phi).*cos(THE_Psi).*sin(THE_Theta)))./2.0+(cg_to_mot_H.*cos(THE_Phi).*cos(THE_Theta).^2.*sin(THE_Psi))./2.0)+mprop.*((cg_to_mot_L.*cos(THE_Psi).*(sin(THE_Phi).*sin(THE_Psi)+cos(THE_Phi).*cos(THE_Psi).*sin(THE_Theta)))./2.0-(cg_to_mot_L.*sin(THE_Psi).*(cos(THE_Psi).*sin(THE_Phi)-cos(THE_Phi).*sin(THE_Psi).*sin(THE_Theta)))./2.0+(cg_to_mot_H.*cos(THE_Phi).*cos(THE_Psi).*cos(THE_Theta))./2.0).*(-(cg_to_mot_H.*sin(THE_Theta)-cg_to_mot_L.*cos(THE_Psi).*cos(THE_Theta)).*(cos(THE_Psi).*sin(THE_Phi)-cos(THE_Phi).*sin(THE_Psi).*sin(THE_Theta))+cg_to_mot_L.*cos(THE_Theta).*sin(THE_Psi).*(sin(THE_Phi).*sin(THE_Psi)+cos(THE_Phi).*cos(THE_Psi).*sin(THE_Theta))+cg_to_mot_H.*cos(THE_Phi).*cos(THE_Theta).^2.*sin(THE_Psi))+mprop.*((cg_to_mot_L.*cos(THE_Psi).*(cos(THE_Phi).*sin(THE_Psi)-cos(THE_Psi).*sin(THE_Phi).*sin(THE_Theta)))./2.0-(cg_to_mot_L.*sin(THE_Psi).*(cos(THE_Phi).*cos(THE_Psi)+sin(THE_Phi).*sin(THE_Psi).*sin(THE_Theta)))./2.0+(cg_to_mot_H.*cos(THE_Psi).*cos(THE_Theta).*sin(THE_Phi))./2.0).*((cg_to_mot_H.*sin(THE_Theta)+cg_to_mot_L.*cos(THE_Psi).*cos(THE_Theta)).*(cos(THE_Phi).*cos(THE_Psi)+sin(THE_Phi).*sin(THE_Psi).*sin(THE_Theta))+cg_to_mot_L.*cos(THE_Theta).*sin(THE_Psi).*(cos(THE_Phi).*sin(THE_Psi)-cos(THE_Psi).*sin(THE_Phi).*sin(THE_Theta))+cg_to_mot_H.*cos(THE_Theta).^2.*sin(THE_Phi).*sin(THE_Psi))+mprop.*(cg_to_mot_L.*cos(THE_Psi).*(cos(THE_Phi).*sin(THE_Psi)-cos(THE_Psi).*sin(THE_Phi).*sin(THE_Theta))-cg_to_mot_L.*sin(THE_Psi).*(cos(THE_Phi).*cos(THE_Psi)+sin(THE_Phi).*sin(THE_Psi).*sin(THE_Theta))+cg_to_mot_H.*cos(THE_Psi).*cos(THE_Theta).*sin(THE_Phi)).*(((cg_to_mot_H.*sin(THE_Theta)+cg_to_mot_L.*cos(THE_Psi).*cos(THE_Theta)).*(cos(THE_Phi).*cos(THE_Psi)+sin(THE_Phi).*sin(THE_Psi).*sin(THE_Theta)))./2.0+(cg_to_mot_L.*cos(THE_Theta).*sin(THE_Psi).*(cos(THE_Phi).*sin(THE_Psi)-cos(THE_Psi).*sin(THE_Phi).*sin(THE_Theta)))./2.0+(cg_to_mot_H.*cos(THE_Theta).^2.*sin(THE_Phi).*sin(THE_Psi))./2.0)+mprop.*(-cg_to_mot_L.*cos(THE_Psi).*(cos(THE_Phi).*sin(THE_Psi)-cos(THE_Psi).*sin(THE_Phi).*sin(THE_Theta))+cg_to_mot_L.*sin(THE_Psi).*(cos(THE_Phi).*cos(THE_Psi)+sin(THE_Phi).*sin(THE_Psi).*sin(THE_Theta))+cg_to_mot_H.*cos(THE_Psi).*cos(THE_Theta).*sin(THE_Phi)).*(((cg_to_mot_H.*sin(THE_Theta)-cg_to_mot_L.*cos(THE_Psi).*cos(THE_Theta)).*(cos(THE_Phi).*cos(THE_Psi)+sin(THE_Phi).*sin(THE_Psi).*sin(THE_Theta)))./2.0-(cg_to_mot_L.*cos(THE_Theta).*sin(THE_Psi).*(cos(THE_Phi).*sin(THE_Psi)-cos(THE_Psi).*sin(THE_Phi).*sin(THE_Theta)))./2.0+(cg_to_mot_H.*cos(THE_Theta).^2.*sin(THE_Phi).*sin(THE_Psi))./2.0)+mprop.*(cg_to_mot_L.*cos(THE_Psi).*(cos(THE_Phi).*sin(THE_Psi)-cos(THE_Psi).*sin(THE_Phi).*sin(THE_Theta)).*(-1.0./2.0)+(cg_to_mot_L.*sin(THE_Psi).*(cos(THE_Phi).*cos(THE_Psi)+sin(THE_Phi).*sin(THE_Psi).*sin(THE_Theta)))./2.0+(cg_to_mot_H.*cos(THE_Psi).*cos(THE_Theta).*sin(THE_Phi))./2.0).*((cg_to_mot_H.*sin(THE_Theta)-cg_to_mot_L.*cos(THE_Psi).*cos(THE_Theta)).*(cos(THE_Phi).*cos(THE_Psi)+sin(THE_Phi).*sin(THE_Psi).*sin(THE_Theta))-cg_to_mot_L.*cos(THE_Theta).*sin(THE_Psi).*(cos(THE_Phi).*sin(THE_Psi)-cos(THE_Psi).*sin(THE_Phi).*sin(THE_Theta))+cg_to_mot_H.*cos(THE_Theta).^2.*sin(THE_Phi).*sin(THE_Psi))-m_pend.*((Lz_pend.*cos(THE_Phi).*sin(THE_Theta).*(sin(THE_Phi_pend).*sin(THE_Psi_pend)+cos(THE_Phi_pend).*cos(THE_Psi_pend).*sin(THE_Theta_pend)))./4.0-(cos(THE_Phi).*cos(THE_Psi).*cos(THE_Theta).*(Tv_Z_pend+(Lz_pend.*cos(THE_Psi_pend).*cos(THE_Theta_pend))./2.0))./2.0+(Lz_pend.*cos(THE_Phi).*cos(THE_Theta).*sin(THE_Psi).*(cos(THE_Phi_pend).*sin(THE_Psi_pend)-cos(THE_Psi_pend).*sin(THE_Phi_pend).*sin(THE_Theta_pend)))./4.0).*((Tv_Z_pend+(Lz_pend.*cos(THE_Psi_pend).*cos(THE_Theta_pend))./2.0).*(cos(THE_Phi).*sin(THE_Psi)-cos(THE_Psi).*sin(THE_Phi).*sin(THE_Theta))+(Lz_pend.*(cos(THE_Phi).*cos(THE_Psi)+sin(THE_Phi).*sin(THE_Psi).*sin(THE_Theta)).*(cos(THE_Phi_pend).*sin(THE_Psi_pend)-cos(THE_Psi_pend).*sin(THE_Phi_pend).*sin(THE_Theta_pend)))./2.0-(Lz_pend.*cos(THE_Theta).*sin(THE_Phi).*(sin(THE_Phi_pend).*sin(THE_Psi_pend)+cos(THE_Phi_pend).*cos(THE_Psi_pend).*sin(THE_Theta_pend)))./2.0)-m_pend.*((Lz_pend.*cos(THE_Phi).*sin(THE_Theta).*(sin(THE_Phi_pend).*sin(THE_Psi_pend)+cos(THE_Phi_pend).*cos(THE_Psi_pend).*sin(THE_Theta_pend)))./2.0-cos(THE_Phi).*cos(THE_Psi).*cos(THE_Theta).*(Tv_Z_pend+(Lz_pend.*cos(THE_Psi_pend).*cos(THE_Theta_pend))./2.0)+(Lz_pend.*cos(THE_Phi).*cos(THE_Theta).*sin(THE_Psi).*(cos(THE_Phi_pend).*sin(THE_Psi_pend)-cos(THE_Psi_pend).*sin(THE_Phi_pend).*sin(THE_Theta_pend)))./2.0).*(((Tv_Z_pend+(Lz_pend.*cos(THE_Psi_pend).*cos(THE_Theta_pend))./2.0).*(cos(THE_Phi).*sin(THE_Psi)-cos(THE_Psi).*sin(THE_Phi).*sin(THE_Theta)))./2.0+(Lz_pend.*(cos(THE_Phi).*cos(THE_Psi)+sin(THE_Phi).*sin(THE_Psi).*sin(THE_Theta)).*(cos(THE_Phi_pend).*sin(THE_Psi_pend)-cos(THE_Psi_pend).*sin(THE_Phi_pend).*sin(THE_Theta_pend)))./4.0-(Lz_pend.*cos(THE_Theta).*sin(THE_Phi).*(sin(THE_Phi_pend).*sin(THE_Psi_pend)+cos(THE_Phi_pend).*cos(THE_Psi_pend).*sin(THE_Theta_pend)))./4.0)+mprop.*(cos(THE_Theta).*sin(THE_Psi).*(cg_to_mot_H.*sin(THE_Theta)+cg_to_mot_L.*cos(THE_Psi).*cos(THE_Theta)).*(-1.0./2.0)+(cg_to_mot_H.*cos(THE_Theta).*sin(THE_Psi).*sin(THE_Theta))./2.0+(cg_to_mot_L.*cos(THE_Psi).*cos(THE_Theta).^2.*sin(THE_Psi))./2.0).*(cg_to_mot_H.*cos(THE_Psi).*sin(THE_Theta)+cg_to_mot_L.*cos(THE_Psi).^2.*cos(THE_Theta)+cg_to_mot_L.*cos(THE_Theta).*sin(THE_Psi).^2)+mprop.*(-cos(THE_Theta).*sin(THE_Psi).*(cg_to_mot_H.*sin(THE_Theta)+cg_to_mot_L.*cos(THE_Psi).*cos(THE_Theta))+cg_to_mot_H.*cos(THE_Theta).*sin(THE_Psi).*sin(THE_Theta)+cg_to_mot_L.*cos(THE_Psi).*cos(THE_Theta).^2.*sin(THE_Psi)).*((cg_to_mot_H.*cos(THE_Psi).*sin(THE_Theta))./2.0+(cg_to_mot_L.*cos(THE_Psi).^2.*cos(THE_Theta))./2.0+(cg_to_mot_L.*cos(THE_Theta).*sin(THE_Psi).^2)./2.0)+mprop.*(cos(THE_Theta).*sin(THE_Psi).*(cg_to_mot_H.*sin(THE_Theta)-cg_to_mot_L.*cos(THE_Psi).*cos(THE_Theta))-cg_to_mot_H.*cos(THE_Theta).*sin(THE_Psi).*sin(THE_Theta)+cg_to_mot_L.*cos(THE_Psi).*cos(THE_Theta).^2.*sin(THE_Psi)).*(cg_to_mot_H.*cos(THE_Psi).*sin(THE_Theta).*(-1.0./2.0)+(cg_to_mot_L.*cos(THE_Psi).^2.*cos(THE_Theta))./2.0+(cg_to_mot_L.*cos(THE_Theta).*sin(THE_Psi).^2)./2.0)+mprop.*((cos(THE_Theta).*sin(THE_Psi).*(cg_to_mot_H.*sin(THE_Theta)-cg_to_mot_L.*cos(THE_Psi).*cos(THE_Theta)))./2.0-(cg_to_mot_H.*cos(THE_Theta).*sin(THE_Psi).*sin(THE_Theta))./2.0+(cg_to_mot_L.*cos(THE_Psi).*cos(THE_Theta).^2.*sin(THE_Psi))./2.0).*(-cg_to_mot_H.*cos(THE_Psi).*sin(THE_Theta)+cg_to_mot_L.*cos(THE_Psi).^2.*cos(THE_Theta)+cg_to_mot_L.*cos(THE_Theta).*sin(THE_Psi).^2)-m_pend.*((Lz_pend.*sin(THE_Phi).*sin(THE_Theta).*(sin(THE_Phi_pend).*sin(THE_Psi_pend)+cos(THE_Phi_pend).*cos(THE_Psi_pend).*sin(THE_Theta_pend)))./4.0-(cos(THE_Psi).*cos(THE_Theta).*sin(THE_Phi).*(Tv_Z_pend+(Lz_pend.*cos(THE_Psi_pend).*cos(THE_Theta_pend))./2.0))./2.0+(Lz_pend.*cos(THE_Theta).*sin(THE_Phi).*sin(THE_Psi).*(cos(THE_Phi_pend).*sin(THE_Psi_pend)-cos(THE_Psi_pend).*sin(THE_Phi_pend).*sin(THE_Theta_pend)))./4.0).*((Tv_Z_pend+(Lz_pend.*cos(THE_Psi_pend).*cos(THE_Theta_pend))./2.0).*(sin(THE_Phi).*sin(THE_Psi)+cos(THE_Phi).*cos(THE_Psi).*sin(THE_Theta))+(Lz_pend.*(cos(THE_Psi).*sin(THE_Phi)-cos(THE_Phi).*sin(THE_Psi).*sin(THE_Theta)).*(cos(THE_Phi_pend).*sin(THE_Psi_pend)-cos(THE_Psi_pend).*sin(THE_Phi_pend).*sin(THE_Theta_pend)))./2.0+(Lz_pend.*cos(THE_Phi).*cos(THE_Theta).*(sin(THE_Phi_pend).*sin(THE_Psi_pend)+cos(THE_Phi_pend).*cos(THE_Psi_pend).*sin(THE_Theta_pend)))./2.0)-m_pend.*((Lz_pend.*sin(THE_Phi).*sin(THE_Theta).*(sin(THE_Phi_pend).*sin(THE_Psi_pend)+cos(THE_Phi_pend).*cos(THE_Psi_pend).*sin(THE_Theta_pend)))./2.0-cos(THE_Psi).*cos(THE_Theta).*sin(THE_Phi).*(Tv_Z_pend+(Lz_pend.*cos(THE_Psi_pend).*cos(THE_Theta_pend))./2.0)+(Lz_pend.*cos(THE_Theta).*sin(THE_Phi).*sin(THE_Psi).*(cos(THE_Phi_pend).*sin(THE_Psi_pend)-cos(THE_Psi_pend).*sin(THE_Phi_pend).*sin(THE_Theta_pend)))./2.0).*(((Tv_Z_pend+(Lz_pend.*cos(THE_Psi_pend).*cos(THE_Theta_pend))./2.0).*(sin(THE_Phi).*sin(THE_Psi)+cos(THE_Phi).*cos(THE_Psi).*sin(THE_Theta)))./2.0+(Lz_pend.*(cos(THE_Psi).*sin(THE_Phi)-cos(THE_Phi).*sin(THE_Psi).*sin(THE_Theta)).*(cos(THE_Phi_pend).*sin(THE_Psi_pend)-cos(THE_Psi_pend).*sin(THE_Phi_pend).*sin(THE_Theta_pend)))./4.0+(Lz_pend.*cos(THE_Phi).*cos(THE_Theta).*(sin(THE_Phi_pend).*sin(THE_Psi_pend)+cos(THE_Phi_pend).*cos(THE_Psi_pend).*sin(THE_Theta_pend)))./4.0)+cos(THE_Psi).*cos(THE_Theta).*((I_yz.*cos(THE_Psi))./2.0-(I_zz.*sin(THE_Psi))./2.0)+cos(THE_Psi).*cos(THE_Theta).*((Iprop_yz.*cos(THE_Psi))./2.0-(Iprop_zz.*sin(THE_Psi))./2.0).*4.0-m_pend.*(Ly_pend.^2./1.2e+1+Lz_pend.^2./1.2e+1).*((sin(THE_Psi).*sin(THE_Theta_pend))./2.0+(cos(THE_Psi).*cos(THE_Theta_pend).*sin(THE_Phi_pend))./2.0).*(cos(THE_Psi).*cos(THE_Theta).*sin(THE_Theta_pend)+cos(THE_Phi_pend).*cos(THE_Theta_pend).*sin(THE_Theta)-cos(THE_Theta).*cos(THE_Theta_pend).*sin(THE_Psi).*sin(THE_Phi_pend))-m_pend.*(Ly_pend.^2./1.2e+1+Lz_pend.^2./1.2e+1).*(sin(THE_Psi).*sin(THE_Theta_pend)+cos(THE_Psi).*cos(THE_Theta_pend).*sin(THE_Phi_pend)).*((cos(THE_Psi).*cos(THE_Theta).*sin(THE_Theta_pend))./2.0+(cos(THE_Phi_pend).*cos(THE_Theta_pend).*sin(THE_Theta))./2.0-(cos(THE_Theta).*cos(THE_Theta_pend).*sin(THE_Psi).*sin(THE_Phi_pend))./2.0)-(mprop.*sin(THE_Theta).*(cg_to_mot_H.*cos(THE_Psi)+cg_to_mot_L.*sin(THE_Psi)).*(sin(THE_Theta).*(cg_to_mot_L.*cos(THE_Psi).*cos(THE_Theta)-cg_to_mot_H.*cos(THE_Theta).*sin(THE_Psi))+cg_to_mot_H.*cos(THE_Theta).*sin(THE_Psi).*sin(THE_Theta)-cg_to_mot_L.*cos(THE_Psi).*cos(THE_Theta).*sin(THE_Theta)))./2.0-(mprop.*sin(THE_Theta).*(cg_to_mot_H.*cos(THE_Psi)-cg_to_mot_L.*sin(THE_Psi)).*(-sin(THE_Theta).*(cg_to_mot_L.*cos(THE_Psi).*cos(THE_Theta)+cg_to_mot_H.*cos(THE_Theta).*sin(THE_Psi))+cg_to_mot_H.*cos(THE_Theta).*sin(THE_Psi).*sin(THE_Theta)+cg_to_mot_L.*cos(THE_Psi).*cos(THE_Theta).*sin(THE_Theta)))./2.0-mprop.*sin(THE_Theta).*(cg_to_mot_H.*cos(THE_Psi)+cg_to_mot_L.*sin(THE_Psi)).*((sin(THE_Theta).*(cg_to_mot_L.*cos(THE_Psi).*cos(THE_Theta)-cg_to_mot_H.*cos(THE_Theta).*sin(THE_Psi)))./2.0+(cg_to_mot_H.*cos(THE_Theta).*sin(THE_Psi).*sin(THE_Theta))./2.0-(cg_to_mot_L.*cos(THE_Psi).*cos(THE_Theta).*sin(THE_Theta))./2.0)-mprop.*sin(THE_Theta).*(cg_to_mot_H.*cos(THE_Psi)-cg_to_mot_L.*sin(THE_Psi)).*(sin(THE_Theta).*(cg_to_mot_L.*cos(THE_Psi).*cos(THE_Theta)+cg_to_mot_H.*cos(THE_Theta).*sin(THE_Psi)).*(-1.0./2.0)+(cg_to_mot_H.*cos(THE_Theta).*sin(THE_Psi).*sin(THE_Theta))./2.0+(cg_to_mot_L.*cos(THE_Psi).*cos(THE_Theta).*sin(THE_Theta))./2.0)+m_pend.*(Lx_pend.^2./1.2e+1+Ly_pend.^2./1.2e+1).*((cos(THE_Psi).*(cos(THE_Phi_pend).*sin(THE_Psi_pend)-cos(THE_Psi_pend).*sin(THE_Phi_pend).*sin(THE_Theta_pend)))./2.0+(cos(THE_Psi_pend).*cos(THE_Theta_pend).*sin(THE_Psi))./2.0).*(sin(THE_Theta).*(sin(THE_Phi_pend).*sin(THE_Psi_pend)+cos(THE_Phi_pend).*cos(THE_Psi_pend).*sin(THE_Theta_pend))+cos(THE_Theta).*sin(THE_Psi).*(cos(THE_Phi_pend).*sin(THE_Psi_pend)-cos(THE_Psi_pend).*sin(THE_Phi_pend).*sin(THE_Theta_pend))-cos(THE_Psi).*cos(THE_Theta).*cos(THE_Psi_pend).*cos(THE_Theta_pend))+m_pend.*(Lx_pend.^2./1.2e+1+Ly_pend.^2./1.2e+1).*(cos(THE_Psi).*(cos(THE_Phi_pend).*sin(THE_Psi_pend)-cos(THE_Psi_pend).*sin(THE_Phi_pend).*sin(THE_Theta_pend))+cos(THE_Psi_pend).*cos(THE_Theta_pend).*sin(THE_Psi)).*((sin(THE_Theta).*(sin(THE_Phi_pend).*sin(THE_Psi_pend)+cos(THE_Phi_pend).*cos(THE_Psi_pend).*sin(THE_Theta_pend)))./2.0+(cos(THE_Theta).*sin(THE_Psi).*(cos(THE_Phi_pend).*sin(THE_Psi_pend)-cos(THE_Psi_pend).*sin(THE_Phi_pend).*sin(THE_Theta_pend)))./2.0-(cos(THE_Psi).*cos(THE_Theta).*cos(THE_Psi_pend).*cos(THE_Theta_pend))./2.0)+m_pend.*((cos(THE_Psi).*(cos(THE_Phi_pend).*cos(THE_Psi_pend)+sin(THE_Phi_pend).*sin(THE_Psi_pend).*sin(THE_Theta_pend)))./2.0-(cos(THE_Theta_pend).*sin(THE_Psi).*sin(THE_Psi_pend))./2.0).*(Lx_pend.^2./1.2e+1+Lz_pend.^2./1.2e+1).*(sin(THE_Theta).*(cos(THE_Psi_pend).*sin(THE_Phi_pend)-cos(THE_Phi_pend).*sin(THE_Psi_pend).*sin(THE_Theta_pend))+cos(THE_Theta).*sin(THE_Psi).*(cos(THE_Phi_pend).*cos(THE_Psi_pend)+sin(THE_Phi_pend).*sin(THE_Psi_pend).*sin(THE_Theta_pend))+cos(THE_Psi).*cos(THE_Theta).*cos(THE_Theta_pend).*sin(THE_Psi_pend))+m_pend.*(cos(THE_Psi).*(cos(THE_Phi_pend).*cos(THE_Psi_pend)+sin(THE_Phi_pend).*sin(THE_Psi_pend).*sin(THE_Theta_pend))-cos(THE_Theta_pend).*sin(THE_Psi).*sin(THE_Psi_pend)).*(Lx_pend.^2./1.2e+1+Lz_pend.^2./1.2e+1).*((sin(THE_Theta).*(cos(THE_Psi_pend).*sin(THE_Phi_pend)-cos(THE_Phi_pend).*sin(THE_Psi_pend).*sin(THE_Theta_pend)))./2.0+(cos(THE_Theta).*sin(THE_Psi).*(cos(THE_Phi_pend).*cos(THE_Psi_pend)+sin(THE_Phi_pend).*sin(THE_Psi_pend).*sin(THE_Theta_pend)))./2.0+(cos(THE_Psi).*cos(THE_Theta).*cos(THE_Theta_pend).*sin(THE_Psi_pend))./2.0)-(mprop.*cos(THE_Phi).*cos(THE_Theta).*(cg_to_mot_H.*cos(THE_Psi)+cg_to_mot_L.*sin(THE_Psi)).*(cg_to_mot_H.*sin(THE_Theta).*(cos(THE_Psi).*sin(THE_Phi)-cos(THE_Phi).*sin(THE_Psi).*sin(THE_Theta))+cg_to_mot_L.*sin(THE_Theta).*(sin(THE_Phi).*sin(THE_Psi)+cos(THE_Phi).*cos(THE_Psi).*sin(THE_Theta))+cos(THE_Phi).*cos(THE_Theta).*(cg_to_mot_L.*cos(THE_Psi).*cos(THE_Theta)-cg_to_mot_H.*cos(THE_Theta).*sin(THE_Psi))))./2.0+(mprop.*cos(THE_Phi).*cos(THE_Theta).*(cg_to_mot_H.*cos(THE_Psi)-cg_to_mot_L.*sin(THE_Psi)).*(-cg_to_mot_H.*sin(THE_Theta).*(cos(THE_Psi).*sin(THE_Phi)-cos(THE_Phi).*sin(THE_Psi).*sin(THE_Theta))+cg_to_mot_L.*sin(THE_Theta).*(sin(THE_Phi).*sin(THE_Psi)+cos(THE_Phi).*cos(THE_Psi).*sin(THE_Theta))+cos(THE_Phi).*cos(THE_Theta).*(cg_to_mot_L.*cos(THE_Psi).*cos(THE_Theta)+cg_to_mot_H.*cos(THE_Theta).*sin(THE_Psi))))./2.0-mprop.*cos(THE_Phi).*cos(THE_Theta).*(cg_to_mot_H.*cos(THE_Psi)+cg_to_mot_L.*sin(THE_Psi)).*((cg_to_mot_H.*sin(THE_Theta).*(cos(THE_Psi).*sin(THE_Phi)-cos(THE_Phi).*sin(THE_Psi).*sin(THE_Theta)))./2.0+(cg_to_mot_L.*sin(THE_Theta).*(sin(THE_Phi).*sin(THE_Psi)+cos(THE_Phi).*cos(THE_Psi).*sin(THE_Theta)))./2.0+(cos(THE_Phi).*cos(THE_Theta).*(cg_to_mot_L.*cos(THE_Psi).*cos(THE_Theta)-cg_to_mot_H.*cos(THE_Theta).*sin(THE_Psi)))./2.0)+mprop.*cos(THE_Phi).*cos(THE_Theta).*(cg_to_mot_H.*cos(THE_Psi)-cg_to_mot_L.*sin(THE_Psi)).*(cg_to_mot_H.*sin(THE_Theta).*(cos(THE_Psi).*sin(THE_Phi)-cos(THE_Phi).*sin(THE_Psi).*sin(THE_Theta)).*(-1.0./2.0)+(cg_to_mot_L.*sin(THE_Theta).*(sin(THE_Phi).*sin(THE_Psi)+cos(THE_Phi).*cos(THE_Psi).*sin(THE_Theta)))./2.0+(cos(THE_Phi).*cos(THE_Theta).*(cg_to_mot_L.*cos(THE_Psi).*cos(THE_Theta)+cg_to_mot_H.*cos(THE_Theta).*sin(THE_Psi)))./2.0)+(mprop.*cos(THE_Theta).*sin(THE_Phi).*(cg_to_mot_H.*cos(THE_Psi)+cg_to_mot_L.*sin(THE_Psi)).*(cg_to_mot_H.*sin(THE_Theta).*(cos(THE_Phi).*cos(THE_Psi)+sin(THE_Phi).*sin(THE_Psi).*sin(THE_Theta))+cg_to_mot_L.*sin(THE_Theta).*(cos(THE_Phi).*sin(THE_Psi)-cos(THE_Psi).*sin(THE_Phi).*sin(THE_Theta))-cos(THE_Theta).*sin(THE_Phi).*(cg_to_mot_L.*cos(THE_Psi).*cos(THE_Theta)-cg_to_mot_H.*cos(THE_Theta).*sin(THE_Psi))))./2.0+(mprop.*cos(THE_Theta).*sin(THE_Phi).*(cg_to_mot_H.*cos(THE_Psi)-cg_to_mot_L.*sin(THE_Psi)).*(cg_to_mot_H.*sin(THE_Theta).*(cos(THE_Phi).*cos(THE_Psi)+sin(THE_Phi).*sin(THE_Psi).*sin(THE_Theta))-cg_to_mot_L.*sin(THE_Theta).*(cos(THE_Phi).*sin(THE_Psi)-cos(THE_Psi).*sin(THE_Phi).*sin(THE_Theta))+cos(THE_Theta).*sin(THE_Phi).*(cg_to_mot_L.*cos(THE_Psi).*cos(THE_Theta)+cg_to_mot_H.*cos(THE_Theta).*sin(THE_Psi))))./2.0+mprop.*cos(THE_Theta).*sin(THE_Phi).*(cg_to_mot_H.*cos(THE_Psi)+cg_to_mot_L.*sin(THE_Psi)).*((cg_to_mot_H.*sin(THE_Theta).*(cos(THE_Phi).*cos(THE_Psi)+sin(THE_Phi).*sin(THE_Psi).*sin(THE_Theta)))./2.0+(cg_to_mot_L.*sin(THE_Theta).*(cos(THE_Phi).*sin(THE_Psi)-cos(THE_Psi).*sin(THE_Phi).*sin(THE_Theta)))./2.0-(cos(THE_Theta).*sin(THE_Phi).*(cg_to_mot_L.*cos(THE_Psi).*cos(THE_Theta)-cg_to_mot_H.*cos(THE_Theta).*sin(THE_Psi)))./2.0)+mprop.*cos(THE_Theta).*sin(THE_Phi).*(cg_to_mot_H.*cos(THE_Psi)-cg_to_mot_L.*sin(THE_Psi)).*((cg_to_mot_H.*sin(THE_Theta).*(cos(THE_Phi).*cos(THE_Psi)+sin(THE_Phi).*sin(THE_Psi).*sin(THE_Theta)))./2.0-(cg_to_mot_L.*sin(THE_Theta).*(cos(THE_Phi).*sin(THE_Psi)-cos(THE_Psi).*sin(THE_Phi).*sin(THE_Theta)))./2.0+(cos(THE_Theta).*sin(THE_Phi).*(cg_to_mot_L.*cos(THE_Psi).*cos(THE_Theta)+cg_to_mot_H.*cos(THE_Theta).*sin(THE_Psi)))./2.0),cos(THE_Psi).*((I_yy.*cos(THE_Psi))./2.0-(I_yz.*sin(THE_Psi))./2.0).*2.0+cos(THE_Psi).*((Iprop_yy.*cos(THE_Psi))./2.0-(Iprop_yz.*sin(THE_Psi))./2.0).*8.0-sin(THE_Psi).*((I_yz.*cos(THE_Psi))./2.0-(I_zz.*sin(THE_Psi))./2.0).*2.0-sin(THE_Psi).*((Iprop_yz.*cos(THE_Psi))./2.0-(Iprop_zz.*sin(THE_Psi))./2.0).*8.0+mprop.*(cg_to_mot_L.*cos(THE_Psi).*(cos(THE_Phi).*sin(THE_Psi)-cos(THE_Psi).*sin(THE_Phi).*sin(THE_Theta))-cg_to_mot_L.*sin(THE_Psi).*(cos(THE_Phi).*cos(THE_Psi)+sin(THE_Phi).*sin(THE_Psi).*sin(THE_Theta))+cg_to_mot_H.*cos(THE_Psi).*cos(THE_Theta).*sin(THE_Phi)).*((cg_to_mot_L.*cos(THE_Psi).*(cos(THE_Phi).*sin(THE_Psi)-cos(THE_Psi).*sin(THE_Phi).*sin(THE_Theta)))./2.0-(cg_to_mot_L.*sin(THE_Psi).*(cos(THE_Phi).*cos(THE_Psi)+sin(THE_Phi).*sin(THE_Psi).*sin(THE_Theta)))./2.0+(cg_to_mot_H.*cos(THE_Psi).*cos(THE_Theta).*sin(THE_Phi))./2.0).*2.0+mprop.*(-cg_to_mot_L.*cos(THE_Psi).*(cos(THE_Phi).*sin(THE_Psi)-cos(THE_Psi).*sin(THE_Phi).*sin(THE_Theta))+cg_to_mot_L.*sin(THE_Psi).*(cos(THE_Phi).*cos(THE_Psi)+sin(THE_Phi).*sin(THE_Psi).*sin(THE_Theta))+cg_to_mot_H.*cos(THE_Psi).*cos(THE_Theta).*sin(THE_Phi)).*(cg_to_mot_L.*cos(THE_Psi).*(cos(THE_Phi).*sin(THE_Psi)-cos(THE_Psi).*sin(THE_Phi).*sin(THE_Theta)).*(-1.0./2.0)+(cg_to_mot_L.*sin(THE_Psi).*(cos(THE_Phi).*cos(THE_Psi)+sin(THE_Phi).*sin(THE_Psi).*sin(THE_Theta)))./2.0+(cg_to_mot_H.*cos(THE_Psi).*cos(THE_Theta).*sin(THE_Phi))./2.0).*2.0+m_pend.*((Lz_pend.*sin(THE_Phi).*sin(THE_Theta).*(sin(THE_Phi_pend).*sin(THE_Psi_pend)+cos(THE_Phi_pend).*cos(THE_Psi_pend).*sin(THE_Theta_pend)))./2.0-cos(THE_Psi).*cos(THE_Theta).*sin(THE_Phi).*(Tv_Z_pend+(Lz_pend.*cos(THE_Psi_pend).*cos(THE_Theta_pend))./2.0)+(Lz_pend.*cos(THE_Theta).*sin(THE_Phi).*sin(THE_Psi).*(cos(THE_Phi_pend).*sin(THE_Psi_pend)-cos(THE_Psi_pend).*sin(THE_Phi_pend).*sin(THE_Theta_pend)))./2.0).*((Lz_pend.*sin(THE_Phi).*sin(THE_Theta).*(sin(THE_Phi_pend).*sin(THE_Psi_pend)+cos(THE_Phi_pend).*cos(THE_Psi_pend).*sin(THE_Theta_pend)))./4.0-(cos(THE_Psi).*cos(THE_Theta).*sin(THE_Phi).*(Tv_Z_pend+(Lz_pend.*cos(THE_Psi_pend).*cos(THE_Theta_pend))./2.0))./2.0+(Lz_pend.*cos(THE_Theta).*sin(THE_Phi).*sin(THE_Psi).*(cos(THE_Phi_pend).*sin(THE_Psi_pend)-cos(THE_Psi_pend).*sin(THE_Phi_pend).*sin(THE_Theta_pend)))./4.0).*2.0+mprop.*(cg_to_mot_H.*cos(THE_Psi).*sin(THE_Theta)+cg_to_mot_L.*cos(THE_Psi).^2.*cos(THE_Theta)+cg_to_mot_L.*cos(THE_Theta).*sin(THE_Psi).^2).*((cg_to_mot_H.*cos(THE_Psi).*sin(THE_Theta))./2.0+(cg_to_mot_L.*cos(THE_Psi).^2.*cos(THE_Theta))./2.0+(cg_to_mot_L.*cos(THE_Theta).*sin(THE_Psi).^2)./2.0).*2.0+mprop.*(-cg_to_mot_H.*cos(THE_Psi).*sin(THE_Theta)+cg_to_mot_L.*cos(THE_Psi).^2.*cos(THE_Theta)+cg_to_mot_L.*cos(THE_Theta).*sin(THE_Psi).^2).*(cg_to_mot_H.*cos(THE_Psi).*sin(THE_Theta).*(-1.0./2.0)+(cg_to_mot_L.*cos(THE_Psi).^2.*cos(THE_Theta))./2.0+(cg_to_mot_L.*cos(THE_Theta).*sin(THE_Psi).^2)./2.0).*2.0+mprop.*sin(THE_Theta).^2.*(cg_to_mot_H.*cos(THE_Psi)+cg_to_mot_L.*sin(THE_Psi)).^2+mprop.*sin(THE_Theta).^2.*(cg_to_mot_H.*cos(THE_Psi)-cg_to_mot_L.*sin(THE_Psi)).^2+m_pend.*((Lz_pend.*cos(THE_Theta).*(sin(THE_Phi_pend).*sin(THE_Psi_pend)+cos(THE_Phi_pend).*cos(THE_Psi_pend).*sin(THE_Theta_pend)))./2.0+cos(THE_Psi).*sin(THE_Theta).*(Tv_Z_pend+(Lz_pend.*cos(THE_Psi_pend).*cos(THE_Theta_pend))./2.0)-(Lz_pend.*sin(THE_Psi).*sin(THE_Theta).*(cos(THE_Phi_pend).*sin(THE_Psi_pend)-cos(THE_Psi_pend).*sin(THE_Phi_pend).*sin(THE_Theta_pend)))./2.0).*((Lz_pend.*cos(THE_Theta).*(sin(THE_Phi_pend).*sin(THE_Psi_pend)+cos(THE_Phi_pend).*cos(THE_Psi_pend).*sin(THE_Theta_pend)))./4.0+(cos(THE_Psi).*sin(THE_Theta).*(Tv_Z_pend+(Lz_pend.*cos(THE_Psi_pend).*cos(THE_Theta_pend))./2.0))./2.0-(Lz_pend.*sin(THE_Psi).*sin(THE_Theta).*(cos(THE_Phi_pend).*sin(THE_Psi_pend)-cos(THE_Psi_pend).*sin(THE_Phi_pend).*sin(THE_Theta_pend)))./4.0).*2.0+m_pend.*((Lz_pend.*cos(THE_Phi).*sin(THE_Theta).*(sin(THE_Phi_pend).*sin(THE_Psi_pend)+cos(THE_Phi_pend).*cos(THE_Psi_pend).*sin(THE_Theta_pend)))./2.0-cos(THE_Phi).*cos(THE_Psi).*cos(THE_Theta).*(Tv_Z_pend+(Lz_pend.*cos(THE_Psi_pend).*cos(THE_Theta_pend))./2.0)+(Lz_pend.*cos(THE_Phi).*cos(THE_Theta).*sin(THE_Psi).*(cos(THE_Phi_pend).*sin(THE_Psi_pend)-cos(THE_Psi_pend).*sin(THE_Phi_pend).*sin(THE_Theta_pend)))./2.0).*((Lz_pend.*cos(THE_Phi).*sin(THE_Theta).*(sin(THE_Phi_pend).*sin(THE_Psi_pend)+cos(THE_Phi_pend).*cos(THE_Psi_pend).*sin(THE_Theta_pend)))./4.0-(cos(THE_Phi).*cos(THE_Psi).*cos(THE_Theta).*(Tv_Z_pend+(Lz_pend.*cos(THE_Psi_pend).*cos(THE_Theta_pend))./2.0))./2.0+(Lz_pend.*cos(THE_Phi).*cos(THE_Theta).*sin(THE_Psi).*(cos(THE_Phi_pend).*sin(THE_Psi_pend)-cos(THE_Psi_pend).*sin(THE_Phi_pend).*sin(THE_Theta_pend)))./4.0).*2.0+mprop.*(cg_to_mot_L.*cos(THE_Psi).*(sin(THE_Phi).*sin(THE_Psi)+cos(THE_Phi).*cos(THE_Psi).*sin(THE_Theta))-cg_to_mot_L.*sin(THE_Psi).*(cos(THE_Psi).*sin(THE_Phi)-cos(THE_Phi).*sin(THE_Psi).*sin(THE_Theta))+cg_to_mot_H.*cos(THE_Phi).*cos(THE_Psi).*cos(THE_Theta)).*((cg_to_mot_L.*cos(THE_Psi).*(sin(THE_Phi).*sin(THE_Psi)+cos(THE_Phi).*cos(THE_Psi).*sin(THE_Theta)))./2.0-(cg_to_mot_L.*sin(THE_Psi).*(cos(THE_Psi).*sin(THE_Phi)-cos(THE_Phi).*sin(THE_Psi).*sin(THE_Theta)))./2.0+(cg_to_mot_H.*cos(THE_Phi).*cos(THE_Psi).*cos(THE_Theta))./2.0).*2.0+mprop.*(-cg_to_mot_L.*cos(THE_Psi).*(sin(THE_Phi).*sin(THE_Psi)+cos(THE_Phi).*cos(THE_Psi).*sin(THE_Theta))+cg_to_mot_L.*sin(THE_Psi).*(cos(THE_Psi).*sin(THE_Phi)-cos(THE_Phi).*sin(THE_Psi).*sin(THE_Theta))+cg_to_mot_H.*cos(THE_Phi).*cos(THE_Psi).*cos(THE_Theta)).*(cg_to_mot_L.*cos(THE_Psi).*(sin(THE_Phi).*sin(THE_Psi)+cos(THE_Phi).*cos(THE_Psi).*sin(THE_Theta)).*(-1.0./2.0)+(cg_to_mot_L.*sin(THE_Psi).*(cos(THE_Psi).*sin(THE_Phi)-cos(THE_Phi).*sin(THE_Psi).*sin(THE_Theta)))./2.0+(cg_to_mot_H.*cos(THE_Phi).*cos(THE_Psi).*cos(THE_Theta))./2.0).*2.0+m_pend.*(Ly_pend.^2./1.2e+1+Lz_pend.^2./1.2e+1).*(sin(THE_Psi).*sin(THE_Theta_pend)+cos(THE_Psi).*cos(THE_Theta_pend).*sin(THE_Phi_pend)).*((sin(THE_Psi).*sin(THE_Theta_pend))./2.0+(cos(THE_Psi).*cos(THE_Theta_pend).*sin(THE_Phi_pend))./2.0).*2.0+m_pend.*(Lx_pend.^2./1.2e+1+Ly_pend.^2./1.2e+1).*(cos(THE_Psi).*(cos(THE_Phi_pend).*sin(THE_Psi_pend)-cos(THE_Psi_pend).*sin(THE_Phi_pend).*sin(THE_Theta_pend))+cos(THE_Psi_pend).*cos(THE_Theta_pend).*sin(THE_Psi)).*((cos(THE_Psi).*(cos(THE_Phi_pend).*sin(THE_Psi_pend)-cos(THE_Psi_pend).*sin(THE_Phi_pend).*sin(THE_Theta_pend)))./2.0+(cos(THE_Psi_pend).*cos(THE_Theta_pend).*sin(THE_Psi))./2.0).*2.0+m_pend.*(cos(THE_Psi).*(cos(THE_Phi_pend).*cos(THE_Psi_pend)+sin(THE_Phi_pend).*sin(THE_Psi_pend).*sin(THE_Theta_pend))-cos(THE_Theta_pend).*sin(THE_Psi).*sin(THE_Psi_pend)).*((cos(THE_Psi).*(cos(THE_Phi_pend).*cos(THE_Psi_pend)+sin(THE_Phi_pend).*sin(THE_Psi_pend).*sin(THE_Theta_pend)))./2.0-(cos(THE_Theta_pend).*sin(THE_Psi).*sin(THE_Psi_pend))./2.0).*(Lx_pend.^2./1.2e+1+Lz_pend.^2./1.2e+1).*2.0+mprop.*cos(THE_Phi).^2.*cos(THE_Theta).^2.*(cg_to_mot_H.*cos(THE_Psi)+cg_to_mot_L.*sin(THE_Psi)).^2+mprop.*cos(THE_Phi).^2.*cos(THE_Theta).^2.*(cg_to_mot_H.*cos(THE_Psi)-cg_to_mot_L.*sin(THE_Psi)).^2+mprop.*cos(THE_Theta).^2.*sin(THE_Phi).^2.*(cg_to_mot_H.*cos(THE_Psi)+cg_to_mot_L.*sin(THE_Psi)).^2+mprop.*cos(THE_Theta).^2.*sin(THE_Phi).^2.*(cg_to_mot_H.*cos(THE_Psi)-cg_to_mot_L.*sin(THE_Psi)).^2,I_xy.*cos(THE_Psi)+Iprop_xy.*cos(THE_Psi).*4.0-I_xz.*sin(THE_Psi)-Iprop_xz.*sin(THE_Psi).*4.0-m_pend.*(((Tv_Z_pend+(Lz_pend.*cos(THE_Psi_pend).*cos(THE_Theta_pend))./2.0).*(cos(THE_Psi).*sin(THE_Phi)-cos(THE_Phi).*sin(THE_Psi).*sin(THE_Theta)))./2.0-(Lz_pend.*(sin(THE_Phi).*sin(THE_Psi)+cos(THE_Phi).*cos(THE_Psi).*sin(THE_Theta)).*(cos(THE_Phi_pend).*sin(THE_Psi_pend)-cos(THE_Psi_pend).*sin(THE_Phi_pend).*sin(THE_Theta_pend)))./4.0).*((Lz_pend.*cos(THE_Phi).*sin(THE_Theta).*(sin(THE_Phi_pend).*sin(THE_Psi_pend)+cos(THE_Phi_pend).*cos(THE_Psi_pend).*sin(THE_Theta_pend)))./2.0-cos(THE_Phi).*cos(THE_Psi).*cos(THE_Theta).*(Tv_Z_pend+(Lz_pend.*cos(THE_Psi_pend).*cos(THE_Theta_pend))./2.0)+(Lz_pend.*cos(THE_Phi).*cos(THE_Theta).*sin(THE_Psi).*(cos(THE_Phi_pend).*sin(THE_Psi_pend)-cos(THE_Psi_pend).*sin(THE_Phi_pend).*sin(THE_Theta_pend)))./2.0)-m_pend.*((Tv_Z_pend+(Lz_pend.*cos(THE_Psi_pend).*cos(THE_Theta_pend))./2.0).*(cos(THE_Psi).*sin(THE_Phi)-cos(THE_Phi).*sin(THE_Psi).*sin(THE_Theta))-(Lz_pend.*(sin(THE_Phi).*sin(THE_Psi)+cos(THE_Phi).*cos(THE_Psi).*sin(THE_Theta)).*(cos(THE_Phi_pend).*sin(THE_Psi_pend)-cos(THE_Psi_pend).*sin(THE_Phi_pend).*sin(THE_Theta_pend)))./2.0).*((Lz_pend.*cos(THE_Phi).*sin(THE_Theta).*(sin(THE_Phi_pend).*sin(THE_Psi_pend)+cos(THE_Phi_pend).*cos(THE_Psi_pend).*sin(THE_Theta_pend)))./4.0-(cos(THE_Phi).*cos(THE_Psi).*cos(THE_Theta).*(Tv_Z_pend+(Lz_pend.*cos(THE_Psi_pend).*cos(THE_Theta_pend))./2.0))./2.0+(Lz_pend.*cos(THE_Phi).*cos(THE_Theta).*sin(THE_Psi).*(cos(THE_Phi_pend).*sin(THE_Psi_pend)-cos(THE_Psi_pend).*sin(THE_Phi_pend).*sin(THE_Theta_pend)))./4.0)+m_pend.*((cos(THE_Theta).*sin(THE_Psi).*(Tv_Z_pend+(Lz_pend.*cos(THE_Psi_pend).*cos(THE_Theta_pend))./2.0))./2.0+(Lz_pend.*cos(THE_Psi).*cos(THE_Theta).*(cos(THE_Phi_pend).*sin(THE_Psi_pend)-cos(THE_Psi_pend).*sin(THE_Phi_pend).*sin(THE_Theta_pend)))./4.0).*((Lz_pend.*cos(THE_Theta).*(sin(THE_Phi_pend).*sin(THE_Psi_pend)+cos(THE_Phi_pend).*cos(THE_Psi_pend).*sin(THE_Theta_pend)))./2.0+cos(THE_Psi).*sin(THE_Theta).*(Tv_Z_pend+(Lz_pend.*cos(THE_Psi_pend).*cos(THE_Theta_pend))./2.0)-(Lz_pend.*sin(THE_Psi).*sin(THE_Theta).*(cos(THE_Phi_pend).*sin(THE_Psi_pend)-cos(THE_Psi_pend).*sin(THE_Phi_pend).*sin(THE_Theta_pend)))./2.0)+m_pend.*(cos(THE_Theta).*sin(THE_Psi).*(Tv_Z_pend+(Lz_pend.*cos(THE_Psi_pend).*cos(THE_Theta_pend))./2.0)+(Lz_pend.*cos(THE_Psi).*cos(THE_Theta).*(cos(THE_Phi_pend).*sin(THE_Psi_pend)-cos(THE_Psi_pend).*sin(THE_Phi_pend).*sin(THE_Theta_pend)))./2.0).*((Lz_pend.*cos(THE_Theta).*(sin(THE_Phi_pend).*sin(THE_Psi_pend)+cos(THE_Phi_pend).*cos(THE_Psi_pend).*sin(THE_Theta_pend)))./4.0+(cos(THE_Psi).*sin(THE_Theta).*(Tv_Z_pend+(Lz_pend.*cos(THE_Psi_pend).*cos(THE_Theta_pend))./2.0))./2.0-(Lz_pend.*sin(THE_Psi).*sin(THE_Theta).*(cos(THE_Phi_pend).*sin(THE_Psi_pend)-cos(THE_Psi_pend).*sin(THE_Phi_pend).*sin(THE_Theta_pend)))./4.0)+m_pend.*(((Tv_Z_pend+(Lz_pend.*cos(THE_Psi_pend).*cos(THE_Theta_pend))./2.0).*(cos(THE_Phi).*cos(THE_Psi)+sin(THE_Phi).*sin(THE_Psi).*sin(THE_Theta)))./2.0-(Lz_pend.*(cos(THE_Phi).*sin(THE_Psi)-cos(THE_Psi).*sin(THE_Phi).*sin(THE_Theta)).*(cos(THE_Phi_pend).*sin(THE_Psi_pend)-cos(THE_Psi_pend).*sin(THE_Phi_pend).*sin(THE_Theta_pend)))./4.0).*((Lz_pend.*sin(THE_Phi).*sin(THE_Theta).*(sin(THE_Phi_pend).*sin(THE_Psi_pend)+cos(THE_Phi_pend).*cos(THE_Psi_pend).*sin(THE_Theta_pend)))./2.0-cos(THE_Psi).*cos(THE_Theta).*sin(THE_Phi).*(Tv_Z_pend+(Lz_pend.*cos(THE_Psi_pend).*cos(THE_Theta_pend))./2.0)+(Lz_pend.*cos(THE_Theta).*sin(THE_Phi).*sin(THE_Psi).*(cos(THE_Phi_pend).*sin(THE_Psi_pend)-cos(THE_Psi_pend).*sin(THE_Phi_pend).*sin(THE_Theta_pend)))./2.0)+m_pend.*((Tv_Z_pend+(Lz_pend.*cos(THE_Psi_pend).*cos(THE_Theta_pend))./2.0).*(cos(THE_Phi).*cos(THE_Psi)+sin(THE_Phi).*sin(THE_Psi).*sin(THE_Theta))-(Lz_pend.*(cos(THE_Phi).*sin(THE_Psi)-cos(THE_Psi).*sin(THE_Phi).*sin(THE_Theta)).*(cos(THE_Phi_pend).*sin(THE_Psi_pend)-cos(THE_Psi_pend).*sin(THE_Phi_pend).*sin(THE_Theta_pend)))./2.0).*((Lz_pend.*sin(THE_Phi).*sin(THE_Theta).*(sin(THE_Phi_pend).*sin(THE_Psi_pend)+cos(THE_Phi_pend).*cos(THE_Psi_pend).*sin(THE_Theta_pend)))./4.0-(cos(THE_Psi).*cos(THE_Theta).*sin(THE_Phi).*(Tv_Z_pend+(Lz_pend.*cos(THE_Psi_pend).*cos(THE_Theta_pend))./2.0))./2.0+(Lz_pend.*cos(THE_Theta).*sin(THE_Phi).*sin(THE_Psi).*(cos(THE_Phi_pend).*sin(THE_Psi_pend)-cos(THE_Psi_pend).*sin(THE_Phi_pend).*sin(THE_Theta_pend)))./4.0)-m_pend.*(Lx_pend.^2./1.2e+1+Ly_pend.^2./1.2e+1).*(sin(THE_Phi_pend).*sin(THE_Psi_pend)+cos(THE_Phi_pend).*cos(THE_Psi_pend).*sin(THE_Theta_pend)).*((cos(THE_Psi).*(cos(THE_Phi_pend).*sin(THE_Psi_pend)-cos(THE_Psi_pend).*sin(THE_Phi_pend).*sin(THE_Theta_pend)))./2.0+(cos(THE_Psi_pend).*cos(THE_Theta_pend).*sin(THE_Psi))./2.0)-m_pend.*(Lx_pend.^2./1.2e+1+Ly_pend.^2./1.2e+1).*((sin(THE_Phi_pend).*sin(THE_Psi_pend))./2.0+(cos(THE_Phi_pend).*cos(THE_Psi_pend).*sin(THE_Theta_pend))./2.0).*(cos(THE_Psi).*(cos(THE_Phi_pend).*sin(THE_Psi_pend)-cos(THE_Psi_pend).*sin(THE_Phi_pend).*sin(THE_Theta_pend))+cos(THE_Psi_pend).*cos(THE_Theta_pend).*sin(THE_Psi))-m_pend.*(cos(THE_Psi).*(cos(THE_Phi_pend).*cos(THE_Psi_pend)+sin(THE_Phi_pend).*sin(THE_Psi_pend).*sin(THE_Theta_pend))-cos(THE_Theta_pend).*sin(THE_Psi).*sin(THE_Psi_pend)).*(Lx_pend.^2./1.2e+1+Lz_pend.^2./1.2e+1).*((cos(THE_Psi_pend).*sin(THE_Phi_pend))./2.0-(cos(THE_Phi_pend).*sin(THE_Psi_pend).*sin(THE_Theta_pend))./2.0)-m_pend.*((cos(THE_Psi).*(cos(THE_Phi_pend).*cos(THE_Psi_pend)+sin(THE_Phi_pend).*sin(THE_Psi_pend).*sin(THE_Theta_pend)))./2.0-(cos(THE_Theta_pend).*sin(THE_Psi).*sin(THE_Psi_pend))./2.0).*(Lx_pend.^2./1.2e+1+Lz_pend.^2./1.2e+1).*(cos(THE_Psi_pend).*sin(THE_Phi_pend)-cos(THE_Phi_pend).*sin(THE_Psi_pend).*sin(THE_Theta_pend))+(cg_to_mot_H.*mprop.*(cos(THE_Psi).*sin(THE_Phi)-cos(THE_Phi).*sin(THE_Psi).*sin(THE_Theta)).*(cg_to_mot_L.*cos(THE_Psi).*(sin(THE_Phi).*sin(THE_Psi)+cos(THE_Phi).*cos(THE_Psi).*sin(THE_Theta))-cg_to_mot_L.*sin(THE_Psi).*(cos(THE_Psi).*sin(THE_Phi)-cos(THE_Phi).*sin(THE_Psi).*sin(THE_Theta))+cg_to_mot_H.*cos(THE_Phi).*cos(THE_Psi).*cos(THE_Theta)))./2.0+(cg_to_mot_H.*mprop.*(cos(THE_Psi).*sin(THE_Phi)-cos(THE_Phi).*sin(THE_Psi).*sin(THE_Theta)).*(-cg_to_mot_L.*cos(THE_Psi).*(sin(THE_Phi).*sin(THE_Psi)+cos(THE_Phi).*cos(THE_Psi).*sin(THE_Theta))+cg_to_mot_L.*sin(THE_Psi).*(cos(THE_Psi).*sin(THE_Phi)-cos(THE_Phi).*sin(THE_Psi).*sin(THE_Theta))+cg_to_mot_H.*cos(THE_Phi).*cos(THE_Psi).*cos(THE_Theta)))./2.0+cg_to_mot_H.*mprop.*(cos(THE_Psi).*sin(THE_Phi)-cos(THE_Phi).*sin(THE_Psi).*sin(THE_Theta)).*(cg_to_mot_L.*cos(THE_Psi).*(sin(THE_Phi).*sin(THE_Psi)+cos(THE_Phi).*cos(THE_Psi).*sin(THE_Theta)).*(-1.0./2.0)+(cg_to_mot_L.*sin(THE_Psi).*(cos(THE_Psi).*sin(THE_Phi)-cos(THE_Phi).*sin(THE_Psi).*sin(THE_Theta)))./2.0+(cg_to_mot_H.*cos(THE_Phi).*cos(THE_Psi).*cos(THE_Theta))./2.0)+cg_to_mot_H.*mprop.*(cos(THE_Psi).*sin(THE_Phi)-cos(THE_Phi).*sin(THE_Psi).*sin(THE_Theta)).*((cg_to_mot_L.*cos(THE_Psi).*(sin(THE_Phi).*sin(THE_Psi)+cos(THE_Phi).*cos(THE_Psi).*sin(THE_Theta)))./2.0-(cg_to_mot_L.*sin(THE_Psi).*(cos(THE_Psi).*sin(THE_Phi)-cos(THE_Phi).*sin(THE_Psi).*sin(THE_Theta)))./2.0+(cg_to_mot_H.*cos(THE_Phi).*cos(THE_Psi).*cos(THE_Theta))./2.0)-(cg_to_mot_H.*mprop.*(cos(THE_Phi).*cos(THE_Psi)+sin(THE_Phi).*sin(THE_Psi).*sin(THE_Theta)).*(cg_to_mot_L.*cos(THE_Psi).*(cos(THE_Phi).*sin(THE_Psi)-cos(THE_Psi).*sin(THE_Phi).*sin(THE_Theta))-cg_to_mot_L.*sin(THE_Psi).*(cos(THE_Phi).*cos(THE_Psi)+sin(THE_Phi).*sin(THE_Psi).*sin(THE_Theta))+cg_to_mot_H.*cos(THE_Psi).*cos(THE_Theta).*sin(THE_Phi)))./2.0-(cg_to_mot_H.*mprop.*(cos(THE_Phi).*cos(THE_Psi)+sin(THE_Phi).*sin(THE_Psi).*sin(THE_Theta)).*(-cg_to_mot_L.*cos(THE_Psi).*(cos(THE_Phi).*sin(THE_Psi)-cos(THE_Psi).*sin(THE_Phi).*sin(THE_Theta))+cg_to_mot_L.*sin(THE_Psi).*(cos(THE_Phi).*cos(THE_Psi)+sin(THE_Phi).*sin(THE_Psi).*sin(THE_Theta))+cg_to_mot_H.*cos(THE_Psi).*cos(THE_Theta).*sin(THE_Phi)))./2.0-cg_to_mot_H.*mprop.*(cos(THE_Phi).*cos(THE_Psi)+sin(THE_Phi).*sin(THE_Psi).*sin(THE_Theta)).*(cg_to_mot_L.*cos(THE_Psi).*(cos(THE_Phi).*sin(THE_Psi)-cos(THE_Psi).*sin(THE_Phi).*sin(THE_Theta)).*(-1.0./2.0)+(cg_to_mot_L.*sin(THE_Psi).*(cos(THE_Phi).*cos(THE_Psi)+sin(THE_Phi).*sin(THE_Psi).*sin(THE_Theta)))./2.0+(cg_to_mot_H.*cos(THE_Psi).*cos(THE_Theta).*sin(THE_Phi))./2.0)-cg_to_mot_H.*mprop.*(cos(THE_Phi).*cos(THE_Psi)+sin(THE_Phi).*sin(THE_Psi).*sin(THE_Theta)).*((cg_to_mot_L.*cos(THE_Psi).*(cos(THE_Phi).*sin(THE_Psi)-cos(THE_Psi).*sin(THE_Phi).*sin(THE_Theta)))./2.0-(cg_to_mot_L.*sin(THE_Psi).*(cos(THE_Phi).*cos(THE_Psi)+sin(THE_Phi).*sin(THE_Psi).*sin(THE_Theta)))./2.0+(cg_to_mot_H.*cos(THE_Psi).*cos(THE_Theta).*sin(THE_Phi))./2.0)-(mprop.*sin(THE_Theta).*(cg_to_mot_H.*cos(THE_Psi)+cg_to_mot_L.*sin(THE_Psi)).*(cg_to_mot_L.*cos(THE_Psi).*cos(THE_Theta)-cg_to_mot_H.*cos(THE_Theta).*sin(THE_Psi)))./2.0+(mprop.*sin(THE_Theta).*(cg_to_mot_H.*cos(THE_Psi)-cg_to_mot_L.*sin(THE_Psi)).*(cg_to_mot_L.*cos(THE_Psi).*cos(THE_Theta)+cg_to_mot_H.*cos(THE_Theta).*sin(THE_Psi)))./2.0-mprop.*sin(THE_Theta).*(cg_to_mot_H.*cos(THE_Psi)+cg_to_mot_L.*sin(THE_Psi)).*((cg_to_mot_L.*cos(THE_Psi).*cos(THE_Theta))./2.0-(cg_to_mot_H.*cos(THE_Theta).*sin(THE_Psi))./2.0)+mprop.*sin(THE_Theta).*(cg_to_mot_H.*cos(THE_Psi)-cg_to_mot_L.*sin(THE_Psi)).*((cg_to_mot_L.*cos(THE_Psi).*cos(THE_Theta))./2.0+(cg_to_mot_H.*cos(THE_Theta).*sin(THE_Psi))./2.0)+(mprop.*cos(THE_Phi).*cos(THE_Theta).*(cg_to_mot_H.*cos(THE_Psi)+cg_to_mot_L.*sin(THE_Psi)).*(cg_to_mot_H.*(cos(THE_Psi).*sin(THE_Phi)-cos(THE_Phi).*sin(THE_Psi).*sin(THE_Theta))+cg_to_mot_L.*(sin(THE_Phi).*sin(THE_Psi)+cos(THE_Phi).*cos(THE_Psi).*sin(THE_Theta))))./2.0+(mprop.*cos(THE_Phi).*cos(THE_Theta).*(cg_to_mot_H.*cos(THE_Psi)-cg_to_mot_L.*sin(THE_Psi)).*(cg_to_mot_H.*(cos(THE_Psi).*sin(THE_Phi)-cos(THE_Phi).*sin(THE_Psi).*sin(THE_Theta))-cg_to_mot_L.*(sin(THE_Phi).*sin(THE_Psi)+cos(THE_Phi).*cos(THE_Psi).*sin(THE_Theta))))./2.0+mprop.*cos(THE_Phi).*cos(THE_Theta).*(cg_to_mot_H.*cos(THE_Psi)+cg_to_mot_L.*sin(THE_Psi)).*((cg_to_mot_H.*(cos(THE_Psi).*sin(THE_Phi)-cos(THE_Phi).*sin(THE_Psi).*sin(THE_Theta)))./2.0+(cg_to_mot_L.*(sin(THE_Phi).*sin(THE_Psi)+cos(THE_Phi).*cos(THE_Psi).*sin(THE_Theta)))./2.0)+mprop.*cos(THE_Phi).*cos(THE_Theta).*(cg_to_mot_H.*cos(THE_Psi)-cg_to_mot_L.*sin(THE_Psi)).*((cg_to_mot_H.*(cos(THE_Psi).*sin(THE_Phi)-cos(THE_Phi).*sin(THE_Psi).*sin(THE_Theta)))./2.0-(cg_to_mot_L.*(sin(THE_Phi).*sin(THE_Psi)+cos(THE_Phi).*cos(THE_Psi).*sin(THE_Theta)))./2.0)-(mprop.*cos(THE_Theta).*sin(THE_Phi).*(cg_to_mot_H.*cos(THE_Psi)+cg_to_mot_L.*sin(THE_Psi)).*(cg_to_mot_H.*(cos(THE_Phi).*cos(THE_Psi)+sin(THE_Phi).*sin(THE_Psi).*sin(THE_Theta))+cg_to_mot_L.*(cos(THE_Phi).*sin(THE_Psi)-cos(THE_Psi).*sin(THE_Phi).*sin(THE_Theta))))./2.0-(mprop.*cos(THE_Theta).*sin(THE_Phi).*(cg_to_mot_H.*cos(THE_Psi)-cg_to_mot_L.*sin(THE_Psi)).*(cg_to_mot_H.*(cos(THE_Phi).*cos(THE_Psi)+sin(THE_Phi).*sin(THE_Psi).*sin(THE_Theta))-cg_to_mot_L.*(cos(THE_Phi).*sin(THE_Psi)-cos(THE_Psi).*sin(THE_Phi).*sin(THE_Theta))))./2.0-mprop.*cos(THE_Theta).*sin(THE_Phi).*(cg_to_mot_H.*cos(THE_Psi)+cg_to_mot_L.*sin(THE_Psi)).*((cg_to_mot_H.*(cos(THE_Phi).*cos(THE_Psi)+sin(THE_Phi).*sin(THE_Psi).*sin(THE_Theta)))./2.0+(cg_to_mot_L.*(cos(THE_Phi).*sin(THE_Psi)-cos(THE_Psi).*sin(THE_Phi).*sin(THE_Theta)))./2.0)-mprop.*cos(THE_Theta).*sin(THE_Phi).*(cg_to_mot_H.*cos(THE_Psi)-cg_to_mot_L.*sin(THE_Psi)).*((cg_to_mot_H.*(cos(THE_Phi).*cos(THE_Psi)+sin(THE_Phi).*sin(THE_Psi).*sin(THE_Theta)))./2.0-(cg_to_mot_L.*(cos(THE_Phi).*sin(THE_Psi)-cos(THE_Psi).*sin(THE_Phi).*sin(THE_Theta)))./2.0)+(cg_to_mot_H.*mprop.*cos(THE_Theta).*sin(THE_Psi).*(cg_to_mot_H.*cos(THE_Psi).*sin(THE_Theta)+cg_to_mot_L.*cos(THE_Psi).^2.*cos(THE_Theta)+cg_to_mot_L.*cos(THE_Theta).*sin(THE_Psi).^2))./2.0-(cg_to_mot_H.*mprop.*cos(THE_Theta).*sin(THE_Psi).*(-cg_to_mot_H.*cos(THE_Psi).*sin(THE_Theta)+cg_to_mot_L.*cos(THE_Psi).^2.*cos(THE_Theta)+cg_to_mot_L.*cos(THE_Theta).*sin(THE_Psi).^2))./2.0-cg_to_mot_H.*mprop.*cos(THE_Theta).*sin(THE_Psi).*(cg_to_mot_H.*cos(THE_Psi).*sin(THE_Theta).*(-1.0./2.0)+(cg_to_mot_L.*cos(THE_Psi).^2.*cos(THE_Theta))./2.0+(cg_to_mot_L.*cos(THE_Theta).*sin(THE_Psi).^2)./2.0)+cg_to_mot_H.*mprop.*cos(THE_Theta).*sin(THE_Psi).*((cg_to_mot_H.*cos(THE_Psi).*sin(THE_Theta))./2.0+(cg_to_mot_L.*cos(THE_Psi).^2.*cos(THE_Theta))./2.0+(cg_to_mot_L.*cos(THE_Theta).*sin(THE_Psi).^2)./2.0)+(m_pend.*cos(THE_Phi_pend).*cos(THE_Theta_pend).*(Ly_pend.^2./1.2e+1+Lz_pend.^2./1.2e+1).*(sin(THE_Psi).*sin(THE_Theta_pend)+cos(THE_Psi).*cos(THE_Theta_pend).*sin(THE_Phi_pend)))./2.0+m_pend.*cos(THE_Phi_pend).*cos(THE_Theta_pend).*(Ly_pend.^2./1.2e+1+Lz_pend.^2./1.2e+1).*((sin(THE_Psi).*sin(THE_Theta_pend))./2.0+(cos(THE_Psi).*cos(THE_Theta_pend).*sin(THE_Phi_pend))./2.0),m_pend.*((Lz_pend.*cos(THE_Phi).*sin(THE_Theta).*(sin(THE_Phi_pend).*sin(THE_Psi_pend)+cos(THE_Phi_pend).*cos(THE_Psi_pend).*sin(THE_Theta_pend)))./2.0-cos(THE_Phi).*cos(THE_Psi).*cos(THE_Theta).*(Tv_Z_pend+(Lz_pend.*cos(THE_Psi_pend).*cos(THE_Theta_pend))./2.0)+(Lz_pend.*cos(THE_Phi).*cos(THE_Theta).*sin(THE_Psi).*(cos(THE_Phi_pend).*sin(THE_Psi_pend)-cos(THE_Psi_pend).*sin(THE_Phi_pend).*sin(THE_Theta_pend)))./2.0).*(-1.0./2.0)-m_pend.*((Lz_pend.*cos(THE_Phi).*sin(THE_Theta).*(sin(THE_Phi_pend).*sin(THE_Psi_pend)+cos(THE_Phi_pend).*cos(THE_Psi_pend).*sin(THE_Theta_pend)))./4.0-(cos(THE_Phi).*cos(THE_Psi).*cos(THE_Theta).*(Tv_Z_pend+(Lz_pend.*cos(THE_Psi_pend).*cos(THE_Theta_pend))./2.0))./2.0+(Lz_pend.*cos(THE_Phi).*cos(THE_Theta).*sin(THE_Psi).*(cos(THE_Phi_pend).*sin(THE_Psi_pend)-cos(THE_Psi_pend).*sin(THE_Phi_pend).*sin(THE_Theta_pend)))./4.0)+(mprop.*(cg_to_mot_L.*cos(THE_Psi).*(sin(THE_Phi).*sin(THE_Psi)+cos(THE_Phi).*cos(THE_Psi).*sin(THE_Theta))-cg_to_mot_L.*sin(THE_Psi).*(cos(THE_Psi).*sin(THE_Phi)-cos(THE_Phi).*sin(THE_Psi).*sin(THE_Theta))+cg_to_mot_H.*cos(THE_Phi).*cos(THE_Psi).*cos(THE_Theta)))./2.0+(mprop.*(-cg_to_mot_L.*cos(THE_Psi).*(sin(THE_Phi).*sin(THE_Psi)+cos(THE_Phi).*cos(THE_Psi).*sin(THE_Theta))+cg_to_mot_L.*sin(THE_Psi).*(cos(THE_Psi).*sin(THE_Phi)-cos(THE_Phi).*sin(THE_Psi).*sin(THE_Theta))+cg_to_mot_H.*cos(THE_Phi).*cos(THE_Psi).*cos(THE_Theta)))./2.0+mprop.*(cg_to_mot_L.*cos(THE_Psi).*(sin(THE_Phi).*sin(THE_Psi)+cos(THE_Phi).*cos(THE_Psi).*sin(THE_Theta)).*(-1.0./2.0)+(cg_to_mot_L.*sin(THE_Psi).*(cos(THE_Psi).*sin(THE_Phi)-cos(THE_Phi).*sin(THE_Psi).*sin(THE_Theta)))./2.0+(cg_to_mot_H.*cos(THE_Phi).*cos(THE_Psi).*cos(THE_Theta))./2.0)+mprop.*((cg_to_mot_L.*cos(THE_Psi).*(sin(THE_Phi).*sin(THE_Psi)+cos(THE_Phi).*cos(THE_Psi).*sin(THE_Theta)))./2.0-(cg_to_mot_L.*sin(THE_Psi).*(cos(THE_Psi).*sin(THE_Phi)-cos(THE_Phi).*sin(THE_Psi).*sin(THE_Theta)))./2.0+(cg_to_mot_H.*cos(THE_Phi).*cos(THE_Psi).*cos(THE_Theta))./2.0)+mprop.*cos(THE_Phi).*cos(THE_Theta).*(cg_to_mot_H.*cos(THE_Psi)+cg_to_mot_L.*sin(THE_Psi))+mprop.*cos(THE_Phi).*cos(THE_Theta).*(cg_to_mot_H.*cos(THE_Psi)-cg_to_mot_L.*sin(THE_Psi)),m_pend.*((Lz_pend.*sin(THE_Phi).*sin(THE_Theta).*(sin(THE_Phi_pend).*sin(THE_Psi_pend)+cos(THE_Phi_pend).*cos(THE_Psi_pend).*sin(THE_Theta_pend)))./2.0-cos(THE_Psi).*cos(THE_Theta).*sin(THE_Phi).*(Tv_Z_pend+(Lz_pend.*cos(THE_Psi_pend).*cos(THE_Theta_pend))./2.0)+(Lz_pend.*cos(THE_Theta).*sin(THE_Phi).*sin(THE_Psi).*(cos(THE_Phi_pend).*sin(THE_Psi_pend)-cos(THE_Psi_pend).*sin(THE_Phi_pend).*sin(THE_Theta_pend)))./2.0).*(-1.0./2.0)-m_pend.*((Lz_pend.*sin(THE_Phi).*sin(THE_Theta).*(sin(THE_Phi_pend).*sin(THE_Psi_pend)+cos(THE_Phi_pend).*cos(THE_Psi_pend).*sin(THE_Theta_pend)))./4.0-(cos(THE_Psi).*cos(THE_Theta).*sin(THE_Phi).*(Tv_Z_pend+(Lz_pend.*cos(THE_Psi_pend).*cos(THE_Theta_pend))./2.0))./2.0+(Lz_pend.*cos(THE_Theta).*sin(THE_Phi).*sin(THE_Psi).*(cos(THE_Phi_pend).*sin(THE_Psi_pend)-cos(THE_Psi_pend).*sin(THE_Phi_pend).*sin(THE_Theta_pend)))./4.0)+(mprop.*(cg_to_mot_L.*cos(THE_Psi).*(cos(THE_Phi).*sin(THE_Psi)-cos(THE_Psi).*sin(THE_Phi).*sin(THE_Theta))-cg_to_mot_L.*sin(THE_Psi).*(cos(THE_Phi).*cos(THE_Psi)+sin(THE_Phi).*sin(THE_Psi).*sin(THE_Theta))+cg_to_mot_H.*cos(THE_Psi).*cos(THE_Theta).*sin(THE_Phi)))./2.0+(mprop.*(-cg_to_mot_L.*cos(THE_Psi).*(cos(THE_Phi).*sin(THE_Psi)-cos(THE_Psi).*sin(THE_Phi).*sin(THE_Theta))+cg_to_mot_L.*sin(THE_Psi).*(cos(THE_Phi).*cos(THE_Psi)+sin(THE_Phi).*sin(THE_Psi).*sin(THE_Theta))+cg_to_mot_H.*cos(THE_Psi).*cos(THE_Theta).*sin(THE_Phi)))./2.0+mprop.*(cg_to_mot_L.*cos(THE_Psi).*(cos(THE_Phi).*sin(THE_Psi)-cos(THE_Psi).*sin(THE_Phi).*sin(THE_Theta)).*(-1.0./2.0)+(cg_to_mot_L.*sin(THE_Psi).*(cos(THE_Phi).*cos(THE_Psi)+sin(THE_Phi).*sin(THE_Psi).*sin(THE_Theta)))./2.0+(cg_to_mot_H.*cos(THE_Psi).*cos(THE_Theta).*sin(THE_Phi))./2.0)+mprop.*((cg_to_mot_L.*cos(THE_Psi).*(cos(THE_Phi).*sin(THE_Psi)-cos(THE_Psi).*sin(THE_Phi).*sin(THE_Theta)))./2.0-(cg_to_mot_L.*sin(THE_Psi).*(cos(THE_Phi).*cos(THE_Psi)+sin(THE_Phi).*sin(THE_Psi).*sin(THE_Theta)))./2.0+(cg_to_mot_H.*cos(THE_Psi).*cos(THE_Theta).*sin(THE_Phi))./2.0)+mprop.*cos(THE_Theta).*sin(THE_Phi).*(cg_to_mot_H.*cos(THE_Psi)+cg_to_mot_L.*sin(THE_Psi))+mprop.*cos(THE_Theta).*sin(THE_Phi).*(cg_to_mot_H.*cos(THE_Psi)-cg_to_mot_L.*sin(THE_Psi)),m_pend.*((Lz_pend.*cos(THE_Theta).*(sin(THE_Phi_pend).*sin(THE_Psi_pend)+cos(THE_Phi_pend).*cos(THE_Psi_pend).*sin(THE_Theta_pend)))./2.0+cos(THE_Psi).*sin(THE_Theta).*(Tv_Z_pend+(Lz_pend.*cos(THE_Psi_pend).*cos(THE_Theta_pend))./2.0)-(Lz_pend.*sin(THE_Psi).*sin(THE_Theta).*(cos(THE_Phi_pend).*sin(THE_Psi_pend)-cos(THE_Psi_pend).*sin(THE_Phi_pend).*sin(THE_Theta_pend)))./2.0).*(-1.0./2.0)-m_pend.*((Lz_pend.*cos(THE_Theta).*(sin(THE_Phi_pend).*sin(THE_Psi_pend)+cos(THE_Phi_pend).*cos(THE_Psi_pend).*sin(THE_Theta_pend)))./4.0+(cos(THE_Psi).*sin(THE_Theta).*(Tv_Z_pend+(Lz_pend.*cos(THE_Psi_pend).*cos(THE_Theta_pend))./2.0))./2.0-(Lz_pend.*sin(THE_Psi).*sin(THE_Theta).*(cos(THE_Phi_pend).*sin(THE_Psi_pend)-cos(THE_Psi_pend).*sin(THE_Phi_pend).*sin(THE_Theta_pend)))./4.0)-(mprop.*(cg_to_mot_H.*cos(THE_Psi).*sin(THE_Theta)+cg_to_mot_L.*cos(THE_Psi).^2.*cos(THE_Theta)+cg_to_mot_L.*cos(THE_Theta).*sin(THE_Psi).^2))./2.0+(mprop.*(-cg_to_mot_H.*cos(THE_Psi).*sin(THE_Theta)+cg_to_mot_L.*cos(THE_Psi).^2.*cos(THE_Theta)+cg_to_mot_L.*cos(THE_Theta).*sin(THE_Psi).^2))./2.0+mprop.*(cg_to_mot_H.*cos(THE_Psi).*sin(THE_Theta).*(-1.0./2.0)+(cg_to_mot_L.*cos(THE_Psi).^2.*cos(THE_Theta))./2.0+(cg_to_mot_L.*cos(THE_Theta).*sin(THE_Psi).^2)./2.0)-mprop.*((cg_to_mot_H.*cos(THE_Psi).*sin(THE_Theta))./2.0+(cg_to_mot_L.*cos(THE_Psi).^2.*cos(THE_Theta))./2.0+(cg_to_mot_L.*cos(THE_Theta).*sin(THE_Psi).^2)./2.0)-mprop.*sin(THE_Theta).*(cg_to_mot_H.*cos(THE_Psi)+cg_to_mot_L.*sin(THE_Psi))-mprop.*sin(THE_Theta).*(cg_to_mot_H.*cos(THE_Psi)-cg_to_mot_L.*sin(THE_Psi)),m_pend.*((Lz_pend.*sin(THE_Theta).*(cos(THE_Phi_pend).*sin(THE_Psi_pend)-cos(THE_Psi_pend).*sin(THE_Phi_pend).*sin(THE_Theta_pend)))./4.0-(Lz_pend.*cos(THE_Theta).*sin(THE_Psi).*(sin(THE_Phi_pend).*sin(THE_Psi_pend)+cos(THE_Phi_pend).*cos(THE_Psi_pend).*sin(THE_Theta_pend)))./4.0).*((Lz_pend.*cos(THE_Theta).*(sin(THE_Phi_pend).*sin(THE_Psi_pend)+cos(THE_Phi_pend).*cos(THE_Psi_pend).*sin(THE_Theta_pend)))./2.0+cos(THE_Psi).*sin(THE_Theta).*(Tv_Z_pend+(Lz_pend.*cos(THE_Psi_pend).*cos(THE_Theta_pend))./2.0)-(Lz_pend.*sin(THE_Psi).*sin(THE_Theta).*(cos(THE_Phi_pend).*sin(THE_Psi_pend)-cos(THE_Psi_pend).*sin(THE_Phi_pend).*sin(THE_Theta_pend)))./2.0)+m_pend.*((Lz_pend.*sin(THE_Theta).*(cos(THE_Phi_pend).*sin(THE_Psi_pend)-cos(THE_Psi_pend).*sin(THE_Phi_pend).*sin(THE_Theta_pend)))./2.0-(Lz_pend.*cos(THE_Theta).*sin(THE_Psi).*(sin(THE_Phi_pend).*sin(THE_Psi_pend)+cos(THE_Phi_pend).*cos(THE_Psi_pend).*sin(THE_Theta_pend)))./2.0).*((Lz_pend.*cos(THE_Theta).*(sin(THE_Phi_pend).*sin(THE_Psi_pend)+cos(THE_Phi_pend).*cos(THE_Psi_pend).*sin(THE_Theta_pend)))./4.0+(cos(THE_Psi).*sin(THE_Theta).*(Tv_Z_pend+(Lz_pend.*cos(THE_Psi_pend).*cos(THE_Theta_pend))./2.0))./2.0-(Lz_pend.*sin(THE_Psi).*sin(THE_Theta).*(cos(THE_Phi_pend).*sin(THE_Psi_pend)-cos(THE_Psi_pend).*sin(THE_Phi_pend).*sin(THE_Theta_pend)))./4.0)+m_pend.*((Lz_pend.*(cos(THE_Psi).*sin(THE_Phi)-cos(THE_Phi).*sin(THE_Psi).*sin(THE_Theta)).*(sin(THE_Phi_pend).*sin(THE_Psi_pend)+cos(THE_Phi_pend).*cos(THE_Psi_pend).*sin(THE_Theta_pend)))./4.0-(Lz_pend.*cos(THE_Phi).*cos(THE_Theta).*(cos(THE_Phi_pend).*sin(THE_Psi_pend)-cos(THE_Psi_pend).*sin(THE_Phi_pend).*sin(THE_Theta_pend)))./4.0).*((Lz_pend.*cos(THE_Phi).*sin(THE_Theta).*(sin(THE_Phi_pend).*sin(THE_Psi_pend)+cos(THE_Phi_pend).*cos(THE_Psi_pend).*sin(THE_Theta_pend)))./2.0-cos(THE_Phi).*cos(THE_Psi).*cos(THE_Theta).*(Tv_Z_pend+(Lz_pend.*cos(THE_Psi_pend).*cos(THE_Theta_pend))./2.0)+(Lz_pend.*cos(THE_Phi).*cos(THE_Theta).*sin(THE_Psi).*(cos(THE_Phi_pend).*sin(THE_Psi_pend)-cos(THE_Psi_pend).*sin(THE_Phi_pend).*sin(THE_Theta_pend)))./2.0)+m_pend.*((Lz_pend.*(cos(THE_Psi).*sin(THE_Phi)-cos(THE_Phi).*sin(THE_Psi).*sin(THE_Theta)).*(sin(THE_Phi_pend).*sin(THE_Psi_pend)+cos(THE_Phi_pend).*cos(THE_Psi_pend).*sin(THE_Theta_pend)))./2.0-(Lz_pend.*cos(THE_Phi).*cos(THE_Theta).*(cos(THE_Phi_pend).*sin(THE_Psi_pend)-cos(THE_Psi_pend).*sin(THE_Phi_pend).*sin(THE_Theta_pend)))./2.0).*((Lz_pend.*cos(THE_Phi).*sin(THE_Theta).*(sin(THE_Phi_pend).*sin(THE_Psi_pend)+cos(THE_Phi_pend).*cos(THE_Psi_pend).*sin(THE_Theta_pend)))./4.0-(cos(THE_Phi).*cos(THE_Psi).*cos(THE_Theta).*(Tv_Z_pend+(Lz_pend.*cos(THE_Psi_pend).*cos(THE_Theta_pend))./2.0))./2.0+(Lz_pend.*cos(THE_Phi).*cos(THE_Theta).*sin(THE_Psi).*(cos(THE_Phi_pend).*sin(THE_Psi_pend)-cos(THE_Psi_pend).*sin(THE_Phi_pend).*sin(THE_Theta_pend)))./4.0)-m_pend.*((Lz_pend.*(cos(THE_Phi).*cos(THE_Psi)+sin(THE_Phi).*sin(THE_Psi).*sin(THE_Theta)).*(sin(THE_Phi_pend).*sin(THE_Psi_pend)+cos(THE_Phi_pend).*cos(THE_Psi_pend).*sin(THE_Theta_pend)))./4.0+(Lz_pend.*cos(THE_Theta).*sin(THE_Phi).*(cos(THE_Phi_pend).*sin(THE_Psi_pend)-cos(THE_Psi_pend).*sin(THE_Phi_pend).*sin(THE_Theta_pend)))./4.0).*((Lz_pend.*sin(THE_Phi).*sin(THE_Theta).*(sin(THE_Phi_pend).*sin(THE_Psi_pend)+cos(THE_Phi_pend).*cos(THE_Psi_pend).*sin(THE_Theta_pend)))./2.0-cos(THE_Psi).*cos(THE_Theta).*sin(THE_Phi).*(Tv_Z_pend+(Lz_pend.*cos(THE_Psi_pend).*cos(THE_Theta_pend))./2.0)+(Lz_pend.*cos(THE_Theta).*sin(THE_Phi).*sin(THE_Psi).*(cos(THE_Phi_pend).*sin(THE_Psi_pend)-cos(THE_Psi_pend).*sin(THE_Phi_pend).*sin(THE_Theta_pend)))./2.0)-m_pend.*((Lz_pend.*(cos(THE_Phi).*cos(THE_Psi)+sin(THE_Phi).*sin(THE_Psi).*sin(THE_Theta)).*(sin(THE_Phi_pend).*sin(THE_Psi_pend)+cos(THE_Phi_pend).*cos(THE_Psi_pend).*sin(THE_Theta_pend)))./2.0+(Lz_pend.*cos(THE_Theta).*sin(THE_Phi).*(cos(THE_Phi_pend).*sin(THE_Psi_pend)-cos(THE_Psi_pend).*sin(THE_Phi_pend).*sin(THE_Theta_pend)))./2.0).*((Lz_pend.*sin(THE_Phi).*sin(THE_Theta).*(sin(THE_Phi_pend).*sin(THE_Psi_pend)+cos(THE_Phi_pend).*cos(THE_Psi_pend).*sin(THE_Theta_pend)))./4.0-(cos(THE_Psi).*cos(THE_Theta).*sin(THE_Phi).*(Tv_Z_pend+(Lz_pend.*cos(THE_Psi_pend).*cos(THE_Theta_pend))./2.0))./2.0+(Lz_pend.*cos(THE_Theta).*sin(THE_Phi).*sin(THE_Psi).*(cos(THE_Phi_pend).*sin(THE_Psi_pend)-cos(THE_Psi_pend).*sin(THE_Phi_pend).*sin(THE_Theta_pend)))./4.0)-(m_pend.*sin(THE_Theta_pend).*(Ly_pend.^2./1.2e+1+Lz_pend.^2./1.2e+1).*(sin(THE_Psi).*sin(THE_Theta_pend)+cos(THE_Psi).*cos(THE_Theta_pend).*sin(THE_Phi_pend)))./2.0-m_pend.*sin(THE_Theta_pend).*(Ly_pend.^2./1.2e+1+Lz_pend.^2./1.2e+1).*((sin(THE_Psi).*sin(THE_Theta_pend))./2.0+(cos(THE_Psi).*cos(THE_Theta_pend).*sin(THE_Phi_pend))./2.0)-(m_pend.*cos(THE_Psi_pend).*cos(THE_Theta_pend).*(Lx_pend.^2./1.2e+1+Ly_pend.^2./1.2e+1).*(cos(THE_Psi).*(cos(THE_Phi_pend).*sin(THE_Psi_pend)-cos(THE_Psi_pend).*sin(THE_Phi_pend).*sin(THE_Theta_pend))+cos(THE_Psi_pend).*cos(THE_Theta_pend).*sin(THE_Psi)))./2.0-m_pend.*cos(THE_Psi_pend).*cos(THE_Theta_pend).*(Lx_pend.^2./1.2e+1+Ly_pend.^2./1.2e+1).*((cos(THE_Psi).*(cos(THE_Phi_pend).*sin(THE_Psi_pend)-cos(THE_Psi_pend).*sin(THE_Phi_pend).*sin(THE_Theta_pend)))./2.0+(cos(THE_Psi_pend).*cos(THE_Theta_pend).*sin(THE_Psi))./2.0)+(m_pend.*cos(THE_Theta_pend).*sin(THE_Psi_pend).*(cos(THE_Psi).*(cos(THE_Phi_pend).*cos(THE_Psi_pend)+sin(THE_Phi_pend).*sin(THE_Psi_pend).*sin(THE_Theta_pend))-cos(THE_Theta_pend).*sin(THE_Psi).*sin(THE_Psi_pend)).*(Lx_pend.^2./1.2e+1+Lz_pend.^2./1.2e+1))./2.0+m_pend.*cos(THE_Theta_pend).*sin(THE_Psi_pend).*((cos(THE_Psi).*(cos(THE_Phi_pend).*cos(THE_Psi_pend)+sin(THE_Phi_pend).*sin(THE_Psi_pend).*sin(THE_Theta_pend)))./2.0-(cos(THE_Theta_pend).*sin(THE_Psi).*sin(THE_Psi_pend))./2.0).*(Lx_pend.^2./1.2e+1+Lz_pend.^2./1.2e+1),-m_pend.*((Lz_pend.*cos(THE_Psi_pend).*sin(THE_Theta_pend).*(cos(THE_Phi).*sin(THE_Psi)-cos(THE_Psi).*sin(THE_Phi).*sin(THE_Theta)))./2.0+(Lz_pend.*cos(THE_Psi_pend).*cos(THE_Theta_pend).*sin(THE_Phi_pend).*(cos(THE_Phi).*cos(THE_Psi)+sin(THE_Phi).*sin(THE_Psi).*sin(THE_Theta)))./2.0+(Lz_pend.*cos(THE_Theta).*cos(THE_Phi_pend).*cos(THE_Psi_pend).*cos(THE_Theta_pend).*sin(THE_Phi))./2.0).*((Lz_pend.*sin(THE_Phi).*sin(THE_Theta).*(sin(THE_Phi_pend).*sin(THE_Psi_pend)+cos(THE_Phi_pend).*cos(THE_Psi_pend).*sin(THE_Theta_pend)))./4.0-(cos(THE_Psi).*cos(THE_Theta).*sin(THE_Phi).*(Tv_Z_pend+(Lz_pend.*cos(THE_Psi_pend).*cos(THE_Theta_pend))./2.0))./2.0+(Lz_pend.*cos(THE_Theta).*sin(THE_Phi).*sin(THE_Psi).*(cos(THE_Phi_pend).*sin(THE_Psi_pend)-cos(THE_Psi_pend).*sin(THE_Phi_pend).*sin(THE_Theta_pend)))./4.0)-m_pend.*((Lz_pend.*cos(THE_Psi_pend).*sin(THE_Theta_pend).*(cos(THE_Phi).*sin(THE_Psi)-cos(THE_Psi).*sin(THE_Phi).*sin(THE_Theta)))./4.0+(Lz_pend.*cos(THE_Psi_pend).*cos(THE_Theta_pend).*sin(THE_Phi_pend).*(cos(THE_Phi).*cos(THE_Psi)+sin(THE_Phi).*sin(THE_Psi).*sin(THE_Theta)))./4.0+(Lz_pend.*cos(THE_Theta).*cos(THE_Phi_pend).*cos(THE_Psi_pend).*cos(THE_Theta_pend).*sin(THE_Phi))./4.0).*((Lz_pend.*sin(THE_Phi).*sin(THE_Theta).*(sin(THE_Phi_pend).*sin(THE_Psi_pend)+cos(THE_Phi_pend).*cos(THE_Psi_pend).*sin(THE_Theta_pend)))./2.0-cos(THE_Psi).*cos(THE_Theta).*sin(THE_Phi).*(Tv_Z_pend+(Lz_pend.*cos(THE_Psi_pend).*cos(THE_Theta_pend))./2.0)+(Lz_pend.*cos(THE_Theta).*sin(THE_Phi).*sin(THE_Psi).*(cos(THE_Phi_pend).*sin(THE_Psi_pend)-cos(THE_Psi_pend).*sin(THE_Phi_pend).*sin(THE_Theta_pend)))./2.0)+m_pend.*((Lz_pend.*cos(THE_Theta).*(sin(THE_Phi_pend).*sin(THE_Psi_pend)+cos(THE_Phi_pend).*cos(THE_Psi_pend).*sin(THE_Theta_pend)))./2.0+cos(THE_Psi).*sin(THE_Theta).*(Tv_Z_pend+(Lz_pend.*cos(THE_Psi_pend).*cos(THE_Theta_pend))./2.0)-(Lz_pend.*sin(THE_Psi).*sin(THE_Theta).*(cos(THE_Phi_pend).*sin(THE_Psi_pend)-cos(THE_Psi_pend).*sin(THE_Phi_pend).*sin(THE_Theta_pend)))./2.0).*((Lz_pend.*cos(THE_Psi).*cos(THE_Theta).*cos(THE_Psi_pend).*sin(THE_Theta_pend))./4.0+(Lz_pend.*cos(THE_Phi_pend).*cos(THE_Psi_pend).*cos(THE_Theta_pend).*sin(THE_Theta))./4.0-(Lz_pend.*cos(THE_Theta).*cos(THE_Psi_pend).*cos(THE_Theta_pend).*sin(THE_Psi).*sin(THE_Phi_pend))./4.0)+m_pend.*((Lz_pend.*cos(THE_Theta).*(sin(THE_Phi_pend).*sin(THE_Psi_pend)+cos(THE_Phi_pend).*cos(THE_Psi_pend).*sin(THE_Theta_pend)))./4.0+(cos(THE_Psi).*sin(THE_Theta).*(Tv_Z_pend+(Lz_pend.*cos(THE_Psi_pend).*cos(THE_Theta_pend))./2.0))./2.0-(Lz_pend.*sin(THE_Psi).*sin(THE_Theta).*(cos(THE_Phi_pend).*sin(THE_Psi_pend)-cos(THE_Psi_pend).*sin(THE_Phi_pend).*sin(THE_Theta_pend)))./4.0).*((Lz_pend.*cos(THE_Psi).*cos(THE_Theta).*cos(THE_Psi_pend).*sin(THE_Theta_pend))./2.0+(Lz_pend.*cos(THE_Phi_pend).*cos(THE_Psi_pend).*cos(THE_Theta_pend).*sin(THE_Theta))./2.0-(Lz_pend.*cos(THE_Theta).*cos(THE_Psi_pend).*cos(THE_Theta_pend).*sin(THE_Psi).*sin(THE_Phi_pend))./2.0)+m_pend.*((Lz_pend.*cos(THE_Psi_pend).*sin(THE_Theta_pend).*(sin(THE_Phi).*sin(THE_Psi)+cos(THE_Phi).*cos(THE_Psi).*sin(THE_Theta)))./2.0+(Lz_pend.*cos(THE_Psi_pend).*cos(THE_Theta_pend).*sin(THE_Phi_pend).*(cos(THE_Psi).*sin(THE_Phi)-cos(THE_Phi).*sin(THE_Psi).*sin(THE_Theta)))./2.0-(Lz_pend.*cos(THE_Phi).*cos(THE_Theta).*cos(THE_Phi_pend).*cos(THE_Psi_pend).*cos(THE_Theta_pend))./2.0).*((Lz_pend.*cos(THE_Phi).*sin(THE_Theta).*(sin(THE_Phi_pend).*sin(THE_Psi_pend)+cos(THE_Phi_pend).*cos(THE_Psi_pend).*sin(THE_Theta_pend)))./4.0-(cos(THE_Phi).*cos(THE_Psi).*cos(THE_Theta).*(Tv_Z_pend+(Lz_pend.*cos(THE_Psi_pend).*cos(THE_Theta_pend))./2.0))./2.0+(Lz_pend.*cos(THE_Phi).*cos(THE_Theta).*sin(THE_Psi).*(cos(THE_Phi_pend).*sin(THE_Psi_pend)-cos(THE_Psi_pend).*sin(THE_Phi_pend).*sin(THE_Theta_pend)))./4.0)+m_pend.*((Lz_pend.*cos(THE_Psi_pend).*sin(THE_Theta_pend).*(sin(THE_Phi).*sin(THE_Psi)+cos(THE_Phi).*cos(THE_Psi).*sin(THE_Theta)))./4.0+(Lz_pend.*cos(THE_Psi_pend).*cos(THE_Theta_pend).*sin(THE_Phi_pend).*(cos(THE_Psi).*sin(THE_Phi)-cos(THE_Phi).*sin(THE_Psi).*sin(THE_Theta)))./4.0-(Lz_pend.*cos(THE_Phi).*cos(THE_Theta).*cos(THE_Phi_pend).*cos(THE_Psi_pend).*cos(THE_Theta_pend))./4.0).*((Lz_pend.*cos(THE_Phi).*sin(THE_Theta).*(sin(THE_Phi_pend).*sin(THE_Psi_pend)+cos(THE_Phi_pend).*cos(THE_Psi_pend).*sin(THE_Theta_pend)))./2.0-cos(THE_Phi).*cos(THE_Psi).*cos(THE_Theta).*(Tv_Z_pend+(Lz_pend.*cos(THE_Psi_pend).*cos(THE_Theta_pend))./2.0)+(Lz_pend.*cos(THE_Phi).*cos(THE_Theta).*sin(THE_Psi).*(cos(THE_Phi_pend).*sin(THE_Psi_pend)-cos(THE_Psi_pend).*sin(THE_Phi_pend).*sin(THE_Theta_pend)))./2.0)+(m_pend.*sin(THE_Psi_pend).*(Lx_pend.^2./1.2e+1+Ly_pend.^2./1.2e+1).*(cos(THE_Psi).*(cos(THE_Phi_pend).*sin(THE_Psi_pend)-cos(THE_Psi_pend).*sin(THE_Phi_pend).*sin(THE_Theta_pend))+cos(THE_Psi_pend).*cos(THE_Theta_pend).*sin(THE_Psi)))./2.0+m_pend.*sin(THE_Psi_pend).*(Lx_pend.^2./1.2e+1+Ly_pend.^2./1.2e+1).*((cos(THE_Psi).*(cos(THE_Phi_pend).*sin(THE_Psi_pend)-cos(THE_Psi_pend).*sin(THE_Phi_pend).*sin(THE_Theta_pend)))./2.0+(cos(THE_Psi_pend).*cos(THE_Theta_pend).*sin(THE_Psi))./2.0)+(m_pend.*cos(THE_Psi_pend).*(cos(THE_Psi).*(cos(THE_Phi_pend).*cos(THE_Psi_pend)+sin(THE_Phi_pend).*sin(THE_Psi_pend).*sin(THE_Theta_pend))-cos(THE_Theta_pend).*sin(THE_Psi).*sin(THE_Psi_pend)).*(Lx_pend.^2./1.2e+1+Lz_pend.^2./1.2e+1))./2.0+m_pend.*cos(THE_Psi_pend).*((cos(THE_Psi).*(cos(THE_Phi_pend).*cos(THE_Psi_pend)+sin(THE_Phi_pend).*sin(THE_Psi_pend).*sin(THE_Theta_pend)))./2.0-(cos(THE_Theta_pend).*sin(THE_Psi).*sin(THE_Psi_pend))./2.0).*(Lx_pend.^2./1.2e+1+Lz_pend.^2./1.2e+1),(m_pend.*(Ly_pend.^2./1.2e+1+Lz_pend.^2./1.2e+1).*(sin(THE_Psi).*sin(THE_Theta_pend)+cos(THE_Psi).*cos(THE_Theta_pend).*sin(THE_Phi_pend)))./2.0+m_pend.*(Ly_pend.^2./1.2e+1+Lz_pend.^2./1.2e+1).*((sin(THE_Psi).*sin(THE_Theta_pend))./2.0+(cos(THE_Psi).*cos(THE_Theta_pend).*sin(THE_Phi_pend))./2.0)-m_pend.*((Lz_pend.*cos(THE_Phi).*sin(THE_Theta).*(sin(THE_Phi_pend).*sin(THE_Psi_pend)+cos(THE_Phi_pend).*cos(THE_Psi_pend).*sin(THE_Theta_pend)))./2.0-cos(THE_Phi).*cos(THE_Psi).*cos(THE_Theta).*(Tv_Z_pend+(Lz_pend.*cos(THE_Psi_pend).*cos(THE_Theta_pend))./2.0)+(Lz_pend.*cos(THE_Phi).*cos(THE_Theta).*sin(THE_Psi).*(cos(THE_Phi_pend).*sin(THE_Psi_pend)-cos(THE_Psi_pend).*sin(THE_Phi_pend).*sin(THE_Theta_pend)))./2.0).*((Lz_pend.*(cos(THE_Psi).*sin(THE_Phi)-cos(THE_Phi).*sin(THE_Psi).*sin(THE_Theta)).*(cos(THE_Phi_pend).*cos(THE_Psi_pend)+sin(THE_Phi_pend).*sin(THE_Psi_pend).*sin(THE_Theta_pend)))./4.0+(Lz_pend.*cos(THE_Phi).*cos(THE_Theta).*(cos(THE_Psi_pend).*sin(THE_Phi_pend)-cos(THE_Phi_pend).*sin(THE_Psi_pend).*sin(THE_Theta_pend)))./4.0-(Lz_pend.*cos(THE_Theta_pend).*sin(THE_Psi_pend).*(sin(THE_Phi).*sin(THE_Psi)+cos(THE_Phi).*cos(THE_Psi).*sin(THE_Theta)))./4.0)-m_pend.*((Lz_pend.*cos(THE_Phi).*sin(THE_Theta).*(sin(THE_Phi_pend).*sin(THE_Psi_pend)+cos(THE_Phi_pend).*cos(THE_Psi_pend).*sin(THE_Theta_pend)))./4.0-(cos(THE_Phi).*cos(THE_Psi).*cos(THE_Theta).*(Tv_Z_pend+(Lz_pend.*cos(THE_Psi_pend).*cos(THE_Theta_pend))./2.0))./2.0+(Lz_pend.*cos(THE_Phi).*cos(THE_Theta).*sin(THE_Psi).*(cos(THE_Phi_pend).*sin(THE_Psi_pend)-cos(THE_Psi_pend).*sin(THE_Phi_pend).*sin(THE_Theta_pend)))./4.0).*((Lz_pend.*(cos(THE_Psi).*sin(THE_Phi)-cos(THE_Phi).*sin(THE_Psi).*sin(THE_Theta)).*(cos(THE_Phi_pend).*cos(THE_Psi_pend)+sin(THE_Phi_pend).*sin(THE_Psi_pend).*sin(THE_Theta_pend)))./2.0+(Lz_pend.*cos(THE_Phi).*cos(THE_Theta).*(cos(THE_Psi_pend).*sin(THE_Phi_pend)-cos(THE_Phi_pend).*sin(THE_Psi_pend).*sin(THE_Theta_pend)))./2.0-(Lz_pend.*cos(THE_Theta_pend).*sin(THE_Psi_pend).*(sin(THE_Phi).*sin(THE_Psi)+cos(THE_Phi).*cos(THE_Psi).*sin(THE_Theta)))./2.0)-m_pend.*((Lz_pend.*sin(THE_Phi).*sin(THE_Theta).*(sin(THE_Phi_pend).*sin(THE_Psi_pend)+cos(THE_Phi_pend).*cos(THE_Psi_pend).*sin(THE_Theta_pend)))./2.0-cos(THE_Psi).*cos(THE_Theta).*sin(THE_Phi).*(Tv_Z_pend+(Lz_pend.*cos(THE_Psi_pend).*cos(THE_Theta_pend))./2.0)+(Lz_pend.*cos(THE_Theta).*sin(THE_Phi).*sin(THE_Psi).*(cos(THE_Phi_pend).*sin(THE_Psi_pend)-cos(THE_Psi_pend).*sin(THE_Phi_pend).*sin(THE_Theta_pend)))./2.0).*(Lz_pend.*(cos(THE_Phi).*cos(THE_Psi)+sin(THE_Phi).*sin(THE_Psi).*sin(THE_Theta)).*(cos(THE_Phi_pend).*cos(THE_Psi_pend)+sin(THE_Phi_pend).*sin(THE_Psi_pend).*sin(THE_Theta_pend)).*(-1.0./4.0)+(Lz_pend.*cos(THE_Theta_pend).*sin(THE_Psi_pend).*(cos(THE_Phi).*sin(THE_Psi)-cos(THE_Psi).*sin(THE_Phi).*sin(THE_Theta)))./4.0+(Lz_pend.*cos(THE_Theta).*sin(THE_Phi).*(cos(THE_Psi_pend).*sin(THE_Phi_pend)-cos(THE_Phi_pend).*sin(THE_Psi_pend).*sin(THE_Theta_pend)))./4.0)-m_pend.*((Lz_pend.*sin(THE_Phi).*sin(THE_Theta).*(sin(THE_Phi_pend).*sin(THE_Psi_pend)+cos(THE_Phi_pend).*cos(THE_Psi_pend).*sin(THE_Theta_pend)))./4.0-(cos(THE_Psi).*cos(THE_Theta).*sin(THE_Phi).*(Tv_Z_pend+(Lz_pend.*cos(THE_Psi_pend).*cos(THE_Theta_pend))./2.0))./2.0+(Lz_pend.*cos(THE_Theta).*sin(THE_Phi).*sin(THE_Psi).*(cos(THE_Phi_pend).*sin(THE_Psi_pend)-cos(THE_Psi_pend).*sin(THE_Phi_pend).*sin(THE_Theta_pend)))./4.0).*(Lz_pend.*(cos(THE_Phi).*cos(THE_Psi)+sin(THE_Phi).*sin(THE_Psi).*sin(THE_Theta)).*(cos(THE_Phi_pend).*cos(THE_Psi_pend)+sin(THE_Phi_pend).*sin(THE_Psi_pend).*sin(THE_Theta_pend)).*(-1.0./2.0)+(Lz_pend.*cos(THE_Theta_pend).*sin(THE_Psi_pend).*(cos(THE_Phi).*sin(THE_Psi)-cos(THE_Psi).*sin(THE_Phi).*sin(THE_Theta)))./2.0+(Lz_pend.*cos(THE_Theta).*sin(THE_Phi).*(cos(THE_Psi_pend).*sin(THE_Phi_pend)-cos(THE_Phi_pend).*sin(THE_Psi_pend).*sin(THE_Theta_pend)))./2.0)+m_pend.*((Lz_pend.*sin(THE_Theta).*(cos(THE_Psi_pend).*sin(THE_Phi_pend)-cos(THE_Phi_pend).*sin(THE_Psi_pend).*sin(THE_Theta_pend)))./4.0+(Lz_pend.*cos(THE_Theta).*sin(THE_Psi).*(cos(THE_Phi_pend).*cos(THE_Psi_pend)+sin(THE_Phi_pend).*sin(THE_Psi_pend).*sin(THE_Theta_pend)))./4.0+(Lz_pend.*cos(THE_Psi).*cos(THE_Theta).*cos(THE_Theta_pend).*sin(THE_Psi_pend))./4.0).*((Lz_pend.*cos(THE_Theta).*(sin(THE_Phi_pend).*sin(THE_Psi_pend)+cos(THE_Phi_pend).*cos(THE_Psi_pend).*sin(THE_Theta_pend)))./2.0+cos(THE_Psi).*sin(THE_Theta).*(Tv_Z_pend+(Lz_pend.*cos(THE_Psi_pend).*cos(THE_Theta_pend))./2.0)-(Lz_pend.*sin(THE_Psi).*sin(THE_Theta).*(cos(THE_Phi_pend).*sin(THE_Psi_pend)-cos(THE_Psi_pend).*sin(THE_Phi_pend).*sin(THE_Theta_pend)))./2.0)+m_pend.*((Lz_pend.*sin(THE_Theta).*(cos(THE_Psi_pend).*sin(THE_Phi_pend)-cos(THE_Phi_pend).*sin(THE_Psi_pend).*sin(THE_Theta_pend)))./2.0+(Lz_pend.*cos(THE_Theta).*sin(THE_Psi).*(cos(THE_Phi_pend).*cos(THE_Psi_pend)+sin(THE_Phi_pend).*sin(THE_Psi_pend).*sin(THE_Theta_pend)))./2.0+(Lz_pend.*cos(THE_Psi).*cos(THE_Theta).*cos(THE_Theta_pend).*sin(THE_Psi_pend))./2.0).*((Lz_pend.*cos(THE_Theta).*(sin(THE_Phi_pend).*sin(THE_Psi_pend)+cos(THE_Phi_pend).*cos(THE_Psi_pend).*sin(THE_Theta_pend)))./4.0+(cos(THE_Psi).*sin(THE_Theta).*(Tv_Z_pend+(Lz_pend.*cos(THE_Psi_pend).*cos(THE_Theta_pend))./2.0))./2.0-(Lz_pend.*sin(THE_Psi).*sin(THE_Theta).*(cos(THE_Phi_pend).*sin(THE_Psi_pend)-cos(THE_Psi_pend).*sin(THE_Phi_pend).*sin(THE_Theta_pend)))./4.0),